simulink model "dynamic_model"  (R2018b)
settings: Solver=ode15s  StartTime=0.0  StopTime=60  FixedStep=0.0001  RelTol=1e-4
undefined symbols (not defined in the file): X, Y, Z
libraries: sm_lib x47, nesl_utility x7
(part 2 of 13)

== matlab function dynamic_model/Dynamic Model/Inertia_matrix ==
  data: q1 input; H output; q2 input; q3 input; q4 input; q5 input; q6 input
function H = Inertia_matrix(q1,q2,q3,q4,q5,q6)
%#codegen

%    This function was generated by the Symbolic Math Toolbox version 9.0.
%    08-Oct-2021 16:14:21

t2 = conj(q1);
t3 = conj(q2);
t4 = conj(q3);
t5 = conj(q4);
t6 = conj(q5);
t7 = conj(q6);
t8 = cos(q1);
t9 = cos(q2);
t10 = cos(q4);
t11 = cos(q5);
t12 = cos(q6);
t13 = sin(q1);
t14 = sin(q2);
t15 = sin(q4);
t16 = sin(q5);
t17 = sin(q6);
t23 = q1+q2;
t44 = 9.007199254740992e+15;
t18 = cos(t2);
t19 = cos(t3);
t20 = cos(t5);
t21 = cos(t6);
t22 = cos(t7);
t24 = sin(t2);
t25 = sin(t3);
t26 = sin(t5);
t27 = sin(t6);
t28 = sin(t7);
t29 = cos(t23);
t30 = sin(t23);
t31 = t2+t3;
t45 = t11.*3.347317932164228e+33;
t48 = t8.*4.990478e-2;
t50 = t13.*4.990478e-2;
t51 = t8.*2.167433e-2;
t52 = t13.*2.167433e-2;
t53 = t10.*t12.*3.315051378778914e+33;
t54 = t8.*t9.*3.641522e-2;
t55 = t8.*t14.*3.641522e-2;
t56 = t9.*t13.*3.641522e-2;
t57 = t15.*t16.*1.990083581481952e+33;
t58 = t13.*t14.*3.641522e-2;
t62 = t13.*t14.*2.462267e-2;
t65 = t11.*t12.*1.025883768304404e+34;
t66 = t11.*t17.*5.575912001630188e+33;
t67 = t10.*t17.*6.099194893302011e+33;
t70 = t8.*t9.*2.462267e-2;
t71 = t8.*t14.*2.462267e-2;
t72 = t9.*t13.*2.462267e-2;
t74 = t15.*t16.*t17.*3.315051378778914e+33;
t81 = t12.*t15.*t16.*6.099194893302011e+33;
t89 = t15.*7.746286054220548e+49;
t92 = t10.*t11.*1.830618490855195e+48;
t94 = t10.*t16.*7.290917220067534e+49;
t96 = t10.*6.997781708721691e+52;
t100 = t10.*t11.*t17.*5.84291401185902e+49;
t102 = t15.*t16.*7.183572847808854e+52;
t103 = t10.*t11.*t12.*1.075008113939401e+50;
t104 = (q3.*t44)./9.007199254740992e+15;
t105 = t10.*t12.*1.196628789628727e+53;
t106 = (t4.*t44)./9.007199254740992e+15;
t109 = t10.*t17.*2.201616617347892e+53;
t110 = q3.*t44.*2.220446049250313e-16i;
t113 = t4.*t44.*2.220446049250313e-16i;
t118 = q3.*t44.*1.110223024625157e-16i;
t119 = t15.*t16.*t17.*1.196628789628727e+53;
t121 = t4.*t44.*1.110223024625157e-16i;
t124 = t12.*t15.*t16.*2.201616617347892e+53;
t128 = t10.*t16.*t44.*4.323455642275676e+17i;
t138 = t12.*t15.*t44.*7.201947557068188e+17i;
t140 = t15.*t17.*t44.*1.325049802940888e+18i;
t152 = t10.*t12.*t16.*t44.*1.325049802940888e+18i;
t154 = t10.*t16.*t17.*t44.*7.201947557068188e+17i;
t193 = t16.*t44.*1.746965228796509e+32i;
t210 = t10.*t44.*4.394953650240249e+33i;
t213 = t11.*t15.*t44.*1.03862462117543e+32i;
t217 = t11.*t44.*6.957746211523004e+33i;
t222 = t15.*t16.*t44.*4.136594366080324e+33i;
t224 = t15.*t44.*3.97028021545552e+36i;
t225 = t12.*t16.*t44.*1.025883768304404e+34i;
t226 = t16.*t17.*t44.*5.575912001630188e+33i;
t229 = t11.*t15.*t17.*t44.*3.315051378778914e+33i;
t234 = t10.*t16.*t44.*4.075691174875038e+36i;
t237 = t11.*t12.*t15.*t44.*6.099194893302011e+33i;
t239 = t12.*t15.*t44.*6.789225223739216e+36i;
t240 = t15.*t17.*t44.*1.249115114148252e+37i;
t249 = t10.*t12.*t16.*t44.*1.249115114148252e+37i;
t251 = t10.*t16.*t17.*t44.*6.789225223739216e+36i;
t284 = t8.*t9.*3.15365435562893e-2;
t285 = t8.*t14.*3.15365435562893e-2;
t286 = t9.*t13.*3.15365435562893e-2;
t287 = t8.*t9.*2.561099610858757e-2;
t289 = t13.*t14.*3.15365435562893e-2;
t290 = t8.*t14.*2.561099610858757e-2;
t291 = t9.*t13.*2.561099610858757e-2;
t292 = t13.*t14.*2.561099610858757e-2;
t294 = t8.*t9.*1.57299335562893e-2;
t296 = t8.*t14.*1.57299335562893e-2;
t297 = t9.*t13.*1.57299335562893e-2;
t298 = t13.*t14.*1.57299335562893e-2;
t299 = t8.*t9.*4.804434610858757e-2;
t300 = t8.*t14.*4.804434610858757e-2;
t301 = t9.*t13.*4.804434610858757e-2;
t302 = t13.*t14.*4.804434610858757e-2;
t311 = t8.*t9.*1.919581841189621e-2;
t313 = t8.*t9.*4.735389991350965e-2;
t315 = t8.*t14.*1.919581841189621e-2;
t316 = t9.*t13.*1.919581841189621e-2;
t317 = t8.*t14.*4.735389991350965e-2;
t318 = t9.*t13.*4.735389991350965e-2;
t319 = t13.*t14.*1.919581841189621e-2;
t320 = t13.*t14.*4.735389991350965e-2;
t321 = t8.*t9.*2.273122991350965e-2;
t322 = t8.*t9.*3.603517512464e-2;
t323 = t8.*t14.*2.273122991350965e-2;
t324 = t9.*t13.*2.273122991350965e-2;
t325 = t8.*t14.*3.603517512464e-2;
t326 = t9.*t13.*3.603517512464e-2;
t327 = t13.*t14.*2.273122991350965e-2;
t328 = t13.*t14.*3.603517512464e-2;
t330 = t8.*t9.*1.141250512464e-2;
t331 = t8.*t14.*1.141250512464e-2;
t332 = t9.*t13.*1.141250512464e-2;
t333 = t13.*t14.*1.141250512464e-2;
t337 = t8.*t9.*5.561103841189621e-2;
t338 = t8.*t14.*5.561103841189621e-2;
t339 = t9.*t13.*5.561103841189621e-2;
t341 = t13.*t14.*5.561103841189621e-2;
t342 = t8.*t9.*3.823389842399381e-2;
t343 = t8.*t14.*3.823389842399381e-2;
t344 = t9.*t13.*3.823389842399381e-2;
t346 = t8.*t9.*7.464911842399381e-2;
t349 = t13.*t14.*3.823389842399381e-2;
t350 = t8.*t14.*7.464911842399381e-2;
t351 = t9.*t13.*7.464911842399381e-2;
t354 = t13.*t14.*7.464911842399381e-2;
t374 = t8.*t9.*t10.*t16.*2.498039274760989e-3;
t375 = t8.*t10.*t14.*t16.*2.498039274760989e-3;
t376 = t9.*t10.*t13.*t16.*2.498039274760989e-3;
t378 = t8.*t9.*t10.*t11.*5.478347731418506e-3;
t379 = t10.*t13.*t14.*t16.*2.498039274760989e-3;
t384 = t8.*t10.*t11.*t14.*5.478347731418506e-3;
t385 = t9.*t10.*t11.*t13.*5.478347731418506e-3;
t388 = t10.*t11.*t13.*t14.*5.478347731418506e-3;
t397 = t8.*t9.*t10.*t16.*4.201698731382561e-3;
t398 = t8.*t10.*t14.*t16.*4.201698731382561e-3;
t399 = t9.*t10.*t13.*t16.*4.201698731382561e-3;
t402 = t10.*t13.*t14.*t16.*4.201698731382561e-3;
t403 = t8.*t9.*t10.*t11.*9.214573584066668e-3;
t404 = t8.*t10.*t11.*t14.*9.214573584066668e-3;
t405 = t9.*t10.*t11.*t13.*9.214573584066668e-3;
t406 = t10.*t11.*t13.*t14.*9.214573584066668e-3;
t410 = t8.*t9.*t15.*2.538961213904336e-3;
t411 = t8.*t14.*t15.*2.538961213904336e-3;
t412 = t9.*t13.*t15.*2.538961213904336e-3;
t413 = t13.*t14.*t15.*2.538961213904336e-3;
t415 = t8.*t9.*t10.*2.842045365580232e-6;
t416 = t8.*t10.*t14.*2.842045365580232e-6;
t417 = t9.*t10.*t13.*2.842045365580232e-6;
t418 = t10.*t13.*t14.*2.842045365580232e-6;
t419 = t10.*t13.*t14.*4.780316517734772e-6;
t420 = t8.*t9.*t15.*4.270529378491088e-3;
t421 = t8.*t14.*t15.*4.270529378491088e-3;
t422 = t9.*t13.*t15.*4.270529378491088e-3;
t423 = t13.*t14.*t15.*4.270529378491088e-3;
t425 = t8.*t9.*t10.*4.780316517734772e-6;
t426 = t8.*t10.*t14.*4.780316517734772e-6;
t427 = t9.*t10.*t13.*4.780316517734772e-6;
t32 = cos(t31);
t33 = sin(t31);
t34 = t30.*7.742227997977903e+15;
t35 = t29.*4.602992943936994e+15;
t36 = t30.*4.602992943936994e+15;
t37 = t29.*7.742227997977903e+15;
t46 = t21.*3.347317932164228e+33;
t47 = t29.*1.580661e-2;
t49 = t30.*1.580661e-2;
t61 = -t52;
t63 = -t53;
t64 = -t54;
t68 = t29.*2.243335e-2;
t69 = t30.*2.243335e-2;
t73 = -t62;
t76 = t20.*t22.*3.315051378778914e+33;
t77 = t26.*t27.*1.990083581481952e+33;
t78 = t21.*t22.*1.025883768304404e+34;
t79 = t21.*t28.*5.575912001630188e+33;
t80 = t20.*t28.*6.099194893302011e+33;
t85 = t26.*t27.*t28.*3.315051378778914e+33;
t86 = t22.*t26.*t27.*6.099194893302011e+33;
t90 = t26.*7.746286054220548e+49;
t91 = -t89;
t95 = -t94;
t97 = t20.*t21.*1.830618490855195e+48;
t98 = t20.*t27.*7.290917220067534e+49;
t99 = t20.*6.997781708721691e+52;
t107 = cos(t104);
t108 = sin(t104);
t111 = t20.*t21.*t28.*5.84291401185902e+49;
t112 = -t105;
t114 = exp(t110);
t115 = cos(t106);
t116 = sin(t106);
t117 = t26.*t27.*7.183572847808854e+52;
t120 = -t113;
t122 = exp(t118);
t123 = t20.*t28.*2.201616617347892e+53;
t125 = t20.*t21.*t22.*1.075008113939401e+50;
t126 = t20.*t22.*1.196628789628727e+53;
t127 = -t118;
t129 = -t121;
t134 = exp(t121);
t141 = t20.*t27.*t44.*4.323455642275676e+17i;
t144 = t26.*t27.*t28.*1.196628789628727e+53;
t148 = -t140;
t149 = t22.*t26.*t27.*2.201616617347892e+53;
t151 = t22.*t26.*t44.*7.201947557068188e+17i;
t153 = t26.*t28.*t44.*1.325049802940888e+18i;
t159 = t20.*t22.*t27.*t44.*1.325049802940888e+18i;
t160 = t20.*t27.*t28.*t44.*7.201947557068188e+17i;
t163 = t18.*7.234522890390001e-5;
t164 = t24.*7.234522890390001e-5;
t165 = t18.*1.665736718274e-4;
t166 = t24.*1.665736718274e-4;
t168 = t18.*1.4420704809832e-3;
t169 = t24.*1.4420704809832e-3;
t170 = t18.*5.42809301582e-4;
t171 = t24.*2.35749519977e-4;
t172 = t24.*5.42809301582e-4;
t173 = t18.*3.62675502933e-4;
t174 = t18.*6.263109763852e-4;
t175 = t24.*3.62675502933e-4;
t176 = t24.*6.263109763852e-4;
t177 = t18.*1.575149421255e-4;
t178 = t24.*1.575149421255e-4;
t180 = t18.*2.35749519977e-4;
t195 = t18.*t19.*2.64642149067e-4;
t196 = t18.*t25.*2.64642149067e-4;
t197 = t19.*t24.*2.64642149067e-4;
t198 = t24.*t25.*2.64642149067e-4;
t201 = t18.*t25.*1.789415608245e-4;
t202 = t19.*t24.*1.789415608245e-4;
t204 = t24.*t25.*1.789415608245e-4;
t211 = t27.*t44.*1.746965228796509e+32i;
t212 = t18.*t19.*1.789415608245e-4;
t215 = t20.*t44.*4.394953650240249e+33i;
t219 = -t210;
t221 = -t213;
t223 = t21.*t44.*6.957746211523004e+33i;
t227 = t21.*t26.*t44.*1.03862462117543e+32i;
t230 = -t224;
t231 = t26.*t27.*t44.*4.136594366080324e+33i;
t232 = t26.*t44.*3.97028021545552e+36i;
t233 = -t229;
t235 = t22.*t27.*t44.*1.025883768304404e+34i;
t236 = t27.*t28.*t44.*5.575912001630188e+33i;
t243 = -t237;
t244 = t20.*t27.*t44.*4.075691174875038e+36i;
t245 = t21.*t26.*t28.*t44.*3.315051378778914e+33i;
t246 = -t240;
t248 = t22.*t26.*t44.*6.789225223739216e+36i;
t250 = t26.*t28.*t44.*1.249115114148252e+37i;
t252 = t21.*t22.*t26.*t44.*6.099194893302011e+33i;
t254 = t20.*t22.*t27.*t44.*1.249115114148252e+37i;
t255 = t20.*t27.*t28.*t44.*6.789225223739216e+36i;
t303 = -t287;
t304 = -t289;
t308 = -t298;
t309 = -t299;
t334 = -t311;
t335 = -t315;
t336 = -t316;
t340 = -t320;
t345 = -t322;
t347 = -t323;
t348 = -t324;
t352 = -t327;
t353 = -t328;
t355 = -t330;
t356 = t18.*t19.*2.273122991350965e-2;
t357 = -t337;
t358 = t18.*t25.*2.273122991350965e-2;
t359 = t19.*t24.*2.273122991350965e-2;
t360 = -t338;
t361 = -t339;
t362 = t24.*t25.*2.273122991350965e-2;
t363 = -t346;
t364 = t18.*t19.*1.141250512464e-2;
t365 = -t349;
t366 = t18.*t25.*1.141250512464e-2;
t367 = t19.*t24.*1.141250512464e-2;
t368 = t24.*t25.*1.141250512464e-2;
t369 = t18.*t19.*1.919581841189621e-2;
t370 = t18.*t25.*1.919581841189621e-2;
t371 = t19.*t24.*1.919581841189621e-2;
t373 = t24.*t25.*1.919581841189621e-2;
t377 = t18.*t19.*3.823389842399381e-2;
t380 = t18.*t25.*3.823389842399381e-2;
t381 = t19.*t24.*3.823389842399381e-2;
t386 = t24.*t25.*3.823389842399381e-2;
t394 = -t374;
t395 = -t375;
t396 = -t376;
t401 = -t388;
t407 = -t398;
t408 = -t399;
t409 = -t402;
t414 = -t403;
t424 = -t413;
t428 = -t418;
t429 = -t420;
t430 = -t425;
t493 = t24.*t25.*5.250384412218911e-5;
t496 = t18.*t19.*8.548515114112684e-5;
t497 = t18.*t25.*8.548515114112684e-5;
t498 = t19.*t24.*8.548515114112684e-5;
t499 = t18.*t19.*1.052636211784891e-4;
t500 = t24.*t25.*8.548515114112684e-5;
t502 = t18.*t25.*1.052636211784891e-4;
t503 = t19.*t24.*1.052636211784891e-4;
t504 = t24.*t25.*1.052636211784891e-4;
t505 = t18.*t19.*5.250384412218911e-5;
t507 = t18.*t25.*5.250384412218911e-5;
t508 = t19.*t24.*5.250384412218911e-5;
t515 = t18.*t19.*1.603638597716268e-4;
t517 = t18.*t25.*1.603638597716268e-4;
t518 = t19.*t24.*1.603638597716268e-4;
t520 = t24.*t25.*1.603638597716268e-4;
t529 = t18.*t19.*1.041288275878652e-3;
t532 = t18.*t25.*1.041288275878652e-3;
t533 = t19.*t24.*1.041288275878652e-3;
t534 = t24.*t25.*1.041288275878652e-3;
t538 = t18.*t19.*5.150636339692531e-4;
t540 = t18.*t25.*5.150636339692531e-4;
t541 = t19.*t24.*5.150636339692531e-4;
t542 = t24.*t25.*5.150636339692531e-4;
t546 = t18.*t19.*8.119509961859382e-4;
t547 = t18.*t19.*1.606961034807054e-3;
t548 = t18.*t25.*8.119509961859382e-4;
t549 = t19.*t24.*8.119509961859382e-4;
t550 = t18.*t25.*1.606961034807054e-3;
t551 = t19.*t24.*1.606961034807054e-3;
t552 = t24.*t25.*8.119509961859382e-4;
t553 = t24.*t25.*1.606961034807054e-3;
t575 = t18.*t19.*t26.*2.761602722751607e-5;
t576 = t18.*t25.*t26.*2.761602722751607e-5;
t577 = t19.*t24.*t26.*2.761602722751607e-5;
t578 = t24.*t25.*t26.*2.761602722751607e-5;
t581 = t18.*t19.*t20.*t21.*5.958744043986595e-5;
t582 = t18.*t20.*t21.*t25.*5.958744043986595e-5;
t583 = t19.*t20.*t21.*t24.*5.958744043986595e-5;
t584 = t20.*t21.*t24.*t25.*5.958744043986595e-5;
t586 = t18.*t19.*t20.*t27.*2.71709233876478e-5;
t587 = t18.*t20.*t25.*t27.*2.71709233876478e-5;
t588 = t19.*t20.*t24.*t27.*2.71709233876478e-5;
t589 = t20.*t24.*t25.*t27.*2.71709233876478e-5;
t591 = t18.*t19.*t20.*t27.*4.570145693137498e-5;
t592 = t18.*t20.*t25.*t27.*4.570145693137498e-5;
t593 = t19.*t20.*t24.*t27.*4.570145693137498e-5;
t594 = t18.*t19.*t20.*3.091264323687963e-8;
t597 = t20.*t24.*t25.*t27.*4.570145693137498e-5;
t598 = t18.*t20.*t25.*3.091264323687963e-8;
t599 = t19.*t20.*t24.*3.091264323687963e-8;
t601 = t20.*t24.*t25.*3.091264323687963e-8;
t603 = t18.*t19.*t26.*4.645012099690971e-5;
t604 = t18.*t25.*t26.*4.645012099690971e-5;
t605 = t19.*t24.*t26.*4.645012099690971e-5;
t606 = t24.*t25.*t26.*4.645012099690971e-5;
t610 = t18.*t19.*t20.*t21.*1.002259954165347e-4;
t612 = t18.*t20.*t21.*t25.*1.002259954165347e-4;
t613 = t19.*t20.*t21.*t24.*1.002259954165347e-4;
t616 = t20.*t21.*t24.*t25.*1.002259954165347e-4;
t625 = t18.*t19.*t20.*5.199502473174935e-8;
t626 = t18.*t20.*t25.*5.199502473174935e-8;
t627 = t19.*t20.*t24.*5.199502473174935e-8;
t628 = t20.*t24.*t25.*5.199502473174935e-8;
t38 = -t36;
t39 = t32.*4.602992943936994e+15;
t40 = t33.*4.602992943936994e+15;
t41 = t32.*7.742227997977903e+15;
t42 = t33.*7.742227997977903e+15;
t59 = -t47;
t60 = -t49;
t75 = -t69;
t82 = -t76;
t83 = t34+t35;
t93 = -t90;
t101 = -t98;
t130 = 1.0./t122;
t131 = t10.*t107;
t132 = t15.*t107;
t133 = exp(t120);
t135 = -t126;
t136 = -t115;
t137 = exp(t129);
t139 = t108.*1i;
t142 = t116.*1i;
t143 = t20.*t115;
t145 = t26.*t115;
t146 = t122-1.0;
t150 = -t141;
t157 = -t151;
t161 = -t159;
t162 = -t160;
t167 = -t164;
t181 = -t171;
t182 = t33.*1.71926916309e-4;
t183 = t32.*4.567547574683999e-4;
t184 = t33.*4.567547574683999e-4;
t185 = -t176;
t186 = t32.*1.148721671835e-4;
t187 = t33.*1.148721671835e-4;
t188 = -t178;
t189 = t32.*1.71926916309e-4;
t200 = t32.*2.44005304615e-4;
t203 = t33.*2.44005304615e-4;
t205 = t32.*6.48243952274e-4;
t206 = t33.*6.48243952274e-4;
t207 = -t195;
t208 = t32.*1.630310061225e-4;
t209 = t33.*1.630310061225e-4;
t216 = -t204;
t220 = -t211;
t228 = -t223;
t238 = -t231;
t241 = -t235;
t242 = -t236;
t247 = -t244;
t253 = -t248;
t256 = -t254;
t257 = -t255;
t258 = t114.*3.064357668490995e+34;
t259 = t45.*t114;
t263 = t53.*t114;
t265 = t57.*t114;
t269 = t10.*t12.*t114.*-3.315051378778914e+33;
t271 = t65.*t114;
t272 = t66.*t114;
t274 = t67.*t114;
t276 = t74.*t114;
t295 = t81.*t114;
t382 = -t358;
t383 = -t359;
t387 = -t362;
t390 = -t364;
t391 = -t369;
t392 = -t370;
t393 = -t371;
t400 = -t386;
t431 = t89.*t114;
t432 = t15.*t114.*-7.746286054220548e+49;
t433 = t92.*t114;
t434 = t94.*t114;
t435 = t10.*t16.*t114.*-7.290917220067534e+49;
t436 = t96.*t114;
t438 = t100.*t114;
t440 = t103.*t114;
t442 = t102.*t114;
t443 = t109.*t114;
t444 = t105.*t114;
t447 = t10.*t12.*t114.*-1.196628789628727e+53;
t449 = t114.*t124;
t450 = t114.*t119;
t451 = t114.*t128;
t454 = t114.*t138;
t455 = t114.*t140;
t457 = t10.*t16.*t44.*t114.*-4.323455642275676e+17i;
t460 = t12.*t15.*t44.*t114.*-7.201947557068188e+17i;
t465 = t114.*t152;
t466 = t114.*t154;
t468 = t107.*7.38843356682345e-1;
t469 = t107.*2.61156643317655e-1;
t472 = t10.*t12.*t16.*t44.*t114.*-1.325049802940888e+18i;
t473 = t10.*t16.*t17.*t44.*t114.*-7.201947557068188e+17i;
t476 = t115.*7.38843356682345e-1;
t477 = t115.*2.61156643317655e-1;
t481 = t107.*4.721390555247569e-2;
t482 = t16.*t107.*1.07201054193752e-2;
t483 = t11.*t107.*4.888197259476159e-3;
t492 = t114.*t193;
t494 = t114.*t210;
t501 = t16.*t44.*t114.*-1.746965228796509e+32i;
t509 = -t493;
t512 = t114.*t213;
t513 = -t496;
t514 = -t504;
t516 = t114.*t217;
t521 = t114.*t222;
t524 = -t515;
t525 = t11.*t44.*t114.*-6.957746211523004e+33i;
t526 = t114.*t225;
t527 = t114.*t226;
t528 = t15.*t16.*t44.*t114.*-4.136594366080324e+33i;
t531 = t114.*t224;
t535 = t12.*t16.*t44.*t114.*-1.025883768304404e+34i;
t536 = t16.*t17.*t44.*t114.*-5.575912001630188e+33i;
t537 = t114.*t229;
t543 = -t529;
t545 = -t534;
t555 = t114.*t234;
H = ft_1({t10,t100,t101,t102,t103,t107,t108,t109,t11,t111,t112,t114,t115,t116,t117,t119,t12,t123,t124,t125,t126,t128,t13,t130,t131,t132,t133,t134,t135,t136,t137,t138,t139,t14,t141,t142,t143,t144,t145,t146,t148,t149,t15,t150,t151,t152,t153,t154,t157,t159,t16,t160,t161,t162,t163,t164,t165,t166,t167,t168,t169,t17,t170,t172,t173,t174,t175,t176,t177,t18,t180,t181,t182,t183,t184,t185,t186,t187,t188,t189,t19,t193,t196,t197,t198,t20,t200,t201,t202,t203,t205,t206,t207,t208,t209,t21,t211,t212,t215,t216,t217,t219,t22,t220,t221,t222,t223,t225,t226,t227,t228,t230,t231,t232,t233,t234,t235,t236,t237,t238,t239,t24,t240,t241,t242,t243,t244,t245,t246,t247,t248,t249,t25,t250,t251,t252,t253,t254,t255,t256,t257,t258,t259,t26,t265,t269,t27,t271,t272,t274,t276,t28,t284,t285,t286,t29,t290,t291,t292,t294,t295,t296,t297,t30,t300,t301,t302,t303,t304,t308,t309,t313,t317,t318,t319,t32,t320,t321,t322,t323,t324,t325,t326,t328,t33,t331,t332,t333,t334,t335,t336,t338,t339,t340,t341,t342,t343,t344,t345,t347,t348,t349,t350,t351,t352,t353,t354,t355,t356,t357,t358,t359,t36,t360,t361,t363,t365,t366,t367,t368,t37,t373,t375,t376,t377,t378,t379,t38,t380,t381,t382,t383,t384,t385,t386,t387,t39,t390,t391,t392,t393,t394,t395,t396,t397,t40,t400,t401,t402,t403,t404,t405,t406,t407,t408,t409,t41,t410,t411,t412,t414,t415,t416,t417,t419,t42,t420,t421,t422,t423,t424,t425,t426,t427,t428,t429,t430,t432,t433,t435,t436,t438,t44,t440,t442,t443,t447,t449,t45,t450,t455,t457,t46,t460,t468,t469,t47,t472,t473,t476,t477,t48,t481,t482,t483,t49,t493,t494,t497,t498,t499,t50,t500,t501,t502,t503,t504,t505,t507,t508,t509,t51,t512,t513,t514,t517,t518,t52,t520,t524,t525,t528,t529,t531,t532,t533,t534,t535,t536,t537,t538,t540,t541,t542,t543,t545,t546,t547,t548,t549,t55,t550,t551,t552,t553,t56,t57,t575,t576,t577,t578,t58,t581,t582,t583,t584,t586,t587,t588,t589,t59,t591,t592,t593,t594,t597,t598,t599,t60,t601,t603,t604,t605,t606,t61,t610,t612,t613,t616,t625,t626,t627,t628,t63,t64,t65,t66,t67,t68,t69,t70,t71,t72,t73,t74,t75,t76,t77,t78,t79,t8,t80,t81,t82,t83,t85,t86,t9,t90,t91,t92,t93,t95,t96,t97,t98,t99});
end
function H = ft_1(ct)
t10 = ct{1};
t100 = ct{2};
t101 = ct{3};
t102 = ct{4};
t103 = ct{5};
t107 = ct{6};
t108 = ct{7};
t109 = ct{8};
t11 = ct{9};
t111 = ct{10};
t112 = ct{11};
t114 = ct{12};
t115 = ct{13};
t116 = ct{14};
t117 = ct{15};
t119 = ct{16};
t12 = ct{17};
t123 = ct{18};
t124 = ct{19};
t125 = ct{20};
t126 = ct{21};
t128 = ct{22};
t13 = ct{23};
t130 = ct{24};
t131 = ct{25};
t132 = ct{26};
t133 = ct{27};
t134 = ct{28};
t135 = ct{29};
t136 = ct{30};
t137 = ct{31};
t138 = ct{32};
t139 = ct{33};
t14 = ct{34};
t141 = ct{35};
t142 = ct{36};
t143 = ct{37};
t144 = ct{38};
t145 = ct{39};
t146 = ct{40};
t148 = ct{41};
t149 = ct{42};
t15 = ct{43};
t150 = ct{44};
t151 = ct{45};
t152 = ct{46};
t153 = ct{47};
t154 = ct{48};
t157 = ct{49};
t159 = ct{50};
t16 = ct{51};
t160 = ct{52};
t161 = ct{53};
t162 = ct{54};
t163 = ct{55};
t164 = ct{56};
t165 = ct{57};
t166 = ct{58};
t167 = ct{59};
t168 = ct{60};
t169 = ct{61};
t17 = ct{62};
t170 = ct{63};
t172 = ct{64};
t173 = ct{65};
t174 = ct{66};
t175 = ct{67};
t176 = ct{68};
t177 = ct{69};
t18 = ct{70};
t180 = ct{71};
t181 = ct{72};
t182 = ct{73};
t183 = ct{74};
t184 = ct{75};
t185 = ct{76};
t186 = ct{77};
t187 = ct{78};
t188 = ct{79};
t189 = ct{80};
t19 = ct{81};
t193 = ct{82};
t196 = ct{83};
t197 = ct{84};
t198 = ct{85};
t20 = ct{86};
t200 = ct{87};
t201 = ct{88};
t202 = ct{89};
t203 = ct{90};
t205 = ct{91};
t206 = ct{92};
t207 = ct{93};
t208 = ct{94};
t209 = ct{95};
t21 = ct{96};
t211 = ct{97};
t212 = ct{98};
t215 = ct{99};
t216 = ct{100};
t217 = ct{101};
t219 = ct{102};
t22 = ct{103};
t220 = ct{104};
t221 = ct{105};
t222 = ct{106};
t223 = ct{107};
t225 = ct{108};
t226 = ct{109};
t227 = ct{110};
t228 = ct{111};
t230 = ct{112};
t231 = ct{113};
t232 = ct{114};
t233 = ct{115};
t234 = ct{116};
t235 = ct{117};
t236 = ct{118};
t237 = ct{119};
t238 = ct{120};
t239 = ct{121};
t24 = ct{122};
t240 = ct{123};
t241 = ct{124};
t242 = ct{125};
t243 = ct{126};
t244 = ct{127};
t245 = ct{128};
t246 = ct{129};
t247 = ct{130};
t248 = ct{131};
t249 = ct{132};
t25 = ct{133};
t250 = ct{134};
t251 = ct{135};
t252 = ct{136};
t253 = ct{137};
t254 = ct{138};
t255 = ct{139};
t256 = ct{140};
t257 = ct{141};
t258 = ct{142};
t259 = ct{143};
t26 = ct{144};
t265 = ct{145};
t269 = ct{146};
t27 = ct{147};
t271 = ct{148};
t272 = ct{149};
t274 = ct{150};
t276 = ct{151};
t28 = ct{152};
t284 = ct{153};
t285 = ct{154};
t286 = ct{155};
t29 = ct{156};
t290 = ct{157};
t291 = ct{158};
t292 = ct{159};
t294 = ct{160};
t295 = ct{161};
t296 = ct{162};
t297 = ct{163};
t30 = ct{164};
t300 = ct{165};
t301 = ct{166};
t302 = ct{167};
t303 = ct{168};
t304 = ct{169};
t308 = ct{170};
t309 = ct{171};
t313 = ct{172};
t317 = ct{173};
t318 = ct{174};
t319 = ct{175};
t32 = ct{176};
t320 = ct{177};
t321 = ct{178};
t322 = ct{179};
t323 = ct{180};
t324 = ct{181};
t325 = ct{182};
t326 = ct{183};
t328 = ct{184};
t33 = ct{185};
t331 = ct{186};
t332 = ct{187};
t333 = ct{188};
t334 = ct{189};
t335 = ct{190};
t336 = ct{191};
t338 = ct{192};
t339 = ct{193};
t340 = ct{194};
t341 = ct{195};
t342 = ct{196};
t343 = ct{197};
t344 = ct{198};
t345 = ct{199};
t347 = ct{200};
t348 = ct{201};
t349 = ct{202};
t350 = ct{203};
t351 = ct{204};
t352 = ct{205};
t353 = ct{206};
t354 = ct{207};
t355 = ct{208};
t356 = ct{209};
t357 = ct{210};
t358 = ct{211};
t359 = ct{212};
t36 = ct{213};
t360 = ct{214};
t361 = ct{215};
t363 = ct{216};
t365 = ct{217};
t366 = ct{218};
t367 = ct{219};
t368 = ct{220};
t37 = ct{221};
t373 = ct{222};
t375 = ct{223};
t376 = ct{224};
t377 = ct{225};
t378 = ct{226};
t379 = ct{227};
t38 = ct{228};
t380 = ct{229};
t381 = ct{230};
t382 = ct{231};
t383 = ct{232};
t384 = ct{233};
t385 = ct{234};
t386 = ct{235};
t387 = ct{236};
t39 = ct{237};
t390 = ct{238};
t391 = ct{239};
t392 = ct{240};
t393 = ct{241};
t394 = ct{242};
t395 = ct{243};
t396 = ct{244};
t397 = ct{245};
t40 = ct{246};
t400 = ct{247};
t401 = ct{248};
t402 = ct{249};
t403 = ct{250};
t404 = ct{251};
t405 = ct{252};
t406 = ct{253};
t407 = ct{254};
t408 = ct{255};
t409 = ct{256};
t41 = ct{257};
t410 = ct{258};
t411 = ct{259};
t412 = ct{260};
t414 = ct{261};
t415 = ct{262};
t416 = ct{263};
t417 = ct{264};
t419 = ct{265};
t42 = ct{266};
t420 = ct{267};
t421 = ct{268};
t422 = ct{269};
t423 = ct{270};
t424 = ct{271};
t425 = ct{272};
t426 = ct{273};
t427 = ct{274};
t428 = ct{275};
t429 = ct{276};
t430 = ct{277};
t432 = ct{278};
t433 = ct{279};
t435 = ct{280};
t436 = ct{281};
t438 = ct{282};
t44 = ct{283};
t440 = ct{284};
t442 = ct{285};
t443 = ct{286};
t447 = ct{287};
t449 = ct{288};
t45 = ct{289};
t450 = ct{290};
t455 = ct{291};
t457 = ct{292};
t46 = ct{293};
t460 = ct{294};
t468 = ct{295};
t469 = ct{296};
t47 = ct{297};
t472 = ct{298};
t473 = ct{299};
t476 = ct{300};
t477 = ct{301};
t48 = ct{302};
t481 = ct{303};
t482 = ct{304};
t483 = ct{305};
t49 = ct{306};
t493 = ct{307};
t494 = ct{308};
t497 = ct{309};
t498 = ct{310};
t499 = ct{311};
t50 = ct{312};
t500 = ct{313};
t501 = ct{314};
t502 = ct{315};
t503 = ct{316};
t504 = ct{317};
t505 = ct{318};
t507 = ct{319};
t508 = ct{320};
t509 = ct{321};
t51 = ct{322};
t512 = ct{323};
t513 = ct{324};
t514 = ct{325};
t517 = ct{326};
t518 = ct{327};
t52 = ct{328};
t520 = ct{329};
t524 = ct{330};
t525 = ct{331};
t528 = ct{332};
t529 = ct{333};
t531 = ct{334};
t532 = ct{335};
t533 = ct{336};
t534 = ct{337};
t535 = ct{338};
t536 = ct{339};
t537 = ct{340};
t538 = ct{341};
t540 = ct{342};
t541 = ct{343};
t542 = ct{344};
t543 = ct{345};
t545 = ct{346};
t546 = ct{347};
t547 = ct{348};
t548 = ct{349};
t549 = ct{350};
t55 = ct{351};
t550 = ct{352};
t551 = ct{353};
t552 = ct{354};
t553 = ct{355};
t56 = ct{356};
t57 = ct{357};
t575 = ct{358};
t576 = ct{359};
t577 = ct{360};
t578 = ct{361};
t58 = ct{362};
t581 = ct{363};
t582 = ct{364};
t583 = ct{365};
t584 = ct{366};
t586 = ct{367};
t587 = ct{368};
t588 = ct{369};
t589 = ct{370};
t59 = ct{371};
t591 = ct{372};
t592 = ct{373};
t593 = ct{374};
t594 = ct{375};
t597 = ct{376};
t598 = ct{377};
t599 = ct{378};
t60 = ct{379};
t601 = ct{380};
t603 = ct{381};
t604 = ct{382};
t605 = ct{383};
t606 = ct{384};
t61 = ct{385};
t610 = ct{386};
t612 = ct{387};
t613 = ct{388};
t616 = ct{389};
t625 = ct{390};
t626 = ct{391};
t627 = ct{392};
t628 = ct{393};
t63 = ct{394};
t64 = ct{395};
t65 = ct{396};
t66 = ct{397};
t67 = ct{398};
t68 = ct{399};
t69 = ct{400};
t70 = ct{401};
t71 = ct{402};
t72 = ct{403};
t73 = ct{404};
t74 = ct{405};
t75 = ct{406};
t76 = ct{407};
t77 = ct{408};
t78 = ct{409};
t79 = ct{410};
t8 = ct{411};
t80 = ct{412};
t81 = ct{413};
t82 = ct{414};
t83 = ct{415};
t85 = ct{416};
t86 = ct{417};
t9 = ct{418};
t90 = ct{419};
t91 = ct{420};
t92 = ct{421};
t93 = ct{422};
t95 = ct{423};
t96 = ct{424};
t97 = ct{425};
t98 = ct{426};
t99 = ct{427};
t556 = -t542;
t557 = t114.*t237;
t558 = -t546;
t559 = -t547;
t560 = -t550;
t561 = -t551;
t564 = t10.*t16.*t44.*t114.*-4.075691174875038e+36i;
t565 = t114.*t239;
t567 = t114.*t240;
t570 = t12.*t15.*t44.*t114.*-6.789225223739216e+36i;
t572 = t114.*t249;
t573 = t114.*t251;
t579 = t10.*t12.*t16.*t44.*t114.*-1.249115114148252e+37i;
t580 = t10.*t16.*t17.*t44.*t114.*-6.789225223739216e+36i;
t595 = -t576;
t596 = -t577;
t600 = -t578;
t607 = -t582;
t608 = -t583;
t609 = -t584;
t614 = -t586;
t617 = -t591;
t618 = -t592;
t619 = -t593;
t620 = -t598;
t621 = -t599;
t622 = -t601;
t624 = -t606;
t630 = -t616;
t631 = -t628;
t633 = t10.*t44.*t108.*5.673626844500105e-17;
t634 = t15.*t44.*t108.*5.673626844500105e-17;
t635 = t11.*t44.*t108.*9.543032792050485e-17;
t636 = t16.*t44.*t108.*9.543032792050485e-17;
t640 = t20.*t44.*t116.*5.673626844500105e-17;
t641 = t26.*t44.*t116.*5.673626844500105e-17;
t642 = t21.*t44.*t116.*9.543032792050485e-17;
t643 = t27.*t44.*t116.*9.543032792050485e-17;
t646 = t11.*t44.*t108.*5.725819675230291e-19;
t647 = t15.*t44.*t108.*7.194245199571015e-21;
t648 = t10.*t11.*t44.*t108.*1.384627967837559e-18;
t649 = t10.*t16.*t44.*t108.*6.313682909819818e-19;
t652 = t21.*t44.*t116.*5.725819675230291e-19;
t654 = t10.*t44.*t108.*5.673626844500105e-25;
t655 = t16.*t44.*t108.*9.543032792050485e-25;
t656 = t107.*t115.*2.2e-7;
t657 = t8.*t9.*t107.*1.374006108587572e-3;
t658 = t8.*t14.*t107.*1.374006108587572e-3;
t659 = t9.*t13.*t107.*1.374006108587572e-3;
t660 = t13.*t14.*t107.*1.374006108587572e-3;
t661 = t13.*t14.*t107.*6.463878411896211e-3;
t662 = t8.*t9.*t107.*2.311076443710702e-3;
t665 = t8.*t14.*t107.*2.311076443710702e-3;
t666 = t9.*t13.*t107.*2.311076443710702e-3;
t668 = t13.*t14.*t107.*2.311076443710702e-3;
t669 = t8.*t9.*t107.*6.463878411896211e-3;
t670 = t8.*t14.*t107.*6.463878411896211e-3;
t671 = t9.*t13.*t107.*6.463878411896211e-3;
t673 = t8.*t9.*t107.*1.087223487536e-2;
t675 = t8.*t14.*t107.*1.087223487536e-2;
t676 = t9.*t13.*t107.*1.087223487536e-2;
t677 = t13.*t14.*t107.*1.087223487536e-2;
t678 = t8.*t9.*t107.*2.550195842399381e-2;
t679 = t8.*t14.*t107.*2.550195842399381e-2;
t680 = t9.*t13.*t107.*2.550195842399381e-2;
t681 = t13.*t14.*t107.*2.550195842399381e-2;
t682 = t115.*5.135409293037228e-4;
t691 = t8.*t9.*t107.*4.289426008649035e-2;
t692 = t8.*t14.*t107.*4.289426008649035e-2;
t693 = t9.*t13.*t107.*4.289426008649035e-2;
t694 = t13.*t14.*t107.*4.289426008649035e-2;
t695 = t18.*t19.*t115.*6.463878411896211e-3;
t696 = t18.*t25.*t115.*6.463878411896211e-3;
t697 = t19.*t24.*t115.*6.463878411896211e-3;
t698 = t24.*t25.*t115.*6.463878411896211e-3;
t700 = t21.*t115.*5.316843277159623e-5;
t701 = t27.*t115.*1.166015146360021e-4;
t710 = t18.*t19.*t115.*1.087223487536e-2;
t715 = t18.*t25.*t115.*1.087223487536e-2;
t716 = t19.*t24.*t115.*1.087223487536e-2;
t720 = t24.*t25.*t115.*1.087223487536e-2;
t728 = t18.*t19.*t115.*2.550195842399381e-2;
t729 = t18.*t25.*t115.*2.550195842399381e-2;
t730 = t19.*t24.*t115.*2.550195842399381e-2;
t731 = t24.*t25.*t115.*2.550195842399381e-2;
t735 = t18.*t25.*t115.*4.289426008649035e-2;
t736 = t19.*t24.*t115.*4.289426008649035e-2;
t737 = t24.*t25.*t115.*4.289426008649035e-2;
t757 = t18.*t19.*t115.*4.289426008649035e-2;
t779 = t10.*t44.*t108.*(t36-t37).*(-1.232595164407831e-32);
t781 = t15.*t44.*t108.*(t36-t37).*(-1.232595164407831e-32);
t782 = (t10.*t44.*t108.*(t36-t37))./8.112963841460668e+31;
t783 = t44.*t108.*1.930470600839964e-18;
t784 = t15.*t44.*t108.*5.582848814988104e-22;
t785 = t44.*t108.*3.311325901843639e-18;
t786 = t44.*t108.*5.241796502683603e-18;
t787 = t44.*t116.*1.930470600839964e-18;
t788 = t44.*t116.*3.311325901843639e-18;
t790 = t44.*t116.*5.241796502683603e-18;
t791 = t11.*t44.*t108.*5.426989146380022e-19;
t793 = t10.*t44.*t108.*3.31613276532711e-19;
t795 = t16.*t44.*t108.*1.190170786299927e-18;
t798 = t10.*t44.*t108.*3.676510195236068e-21;
t800 = t10.*t44.*t108.*4.442449819243582e-22;
t802 = t10.*t44.*t108.*3.517648643590065e-23;
t803 = t44.*t108.*3.091942624624357e-22;
t805 = t10.*t11.*t44.*t108.*7.075931802640439e-19;
t809 = t10.*t44.*t108.*1.838255097618034e-22;
t810 = t10.*t16.*t44.*t108.*3.226512155691387e-19;
t811 = t21.*t44.*t116.*5.426989146380022e-19;
t812 = t20.*t44.*t116.*3.31613276532711e-19;
t813 = t44.*t108.*2.967883198327701e-22;
t814 = t27.*t44.*t116.*1.190170786299927e-18;
t817 = t15.*t44.*t108.*3.279367663374749e-19;
t819 = t10.*t44.*t108.*3.670836568391568e-22;
t820 = t15.*t44.*t108.*3.670836568391568e-22;
t822 = t11.*t44.*t108.*2.988305288502687e-20;
t823 = t20.*t44.*t116.*3.676510195236068e-21;
t824 = t11.*t44.*t108.*5.439528691468777e-23;
t825 = t16.*t44.*t108.*9.733893447891495e-23;
t829 = t16.*t44.*t108.*2.290327870092116e-23;
t830 = t26.*t44.*t116.*3.670836568391568e-22;
t831 = t21.*t44.*t116.*2.988305288502687e-20;
t832 = t8.*t9.*t15.*t16.*t44.*t108.*3.226512155691387e-19;
t833 = t8.*t14.*t15.*t16.*t44.*t108.*3.226512155691387e-19;
t834 = t9.*t13.*t15.*t16.*t44.*t108.*3.226512155691387e-19;
t835 = t13.*t14.*t15.*t16.*t44.*t108.*3.226512155691387e-19;
t836 = t8.*t9.*t15.*t16.*t44.*t108.*5.426989146380022e-19;
t837 = t8.*t14.*t15.*t16.*t44.*t108.*5.426989146380022e-19;
t838 = t9.*t13.*t15.*t16.*t44.*t108.*5.426989146380022e-19;
t839 = t26.*t44.*t116.*7.825108561121397e-23;
t841 = t13.*t14.*t15.*t16.*t44.*t108.*5.426989146380022e-19;
t842 = t8.*t9.*t11.*t15.*t44.*t108.*1.190170786299927e-18;
t844 = t8.*t11.*t14.*t15.*t44.*t108.*1.190170786299927e-18;
t845 = t9.*t11.*t13.*t15.*t44.*t108.*1.190170786299927e-18;
t846 = t11.*t13.*t14.*t15.*t44.*t108.*1.190170786299927e-18;
t847 = t8.*t9.*t11.*t15.*t44.*t108.*7.075931802640439e-19;
t848 = t8.*t11.*t14.*t15.*t44.*t108.*7.075931802640439e-19;
t849 = t9.*t11.*t13.*t15.*t44.*t108.*7.075931802640439e-19;
t850 = t11.*t13.*t14.*t15.*t44.*t108.*7.075931802640439e-19;
t851 = t11.*t44.*t108.*3.817213116820194e-24;
t852 = t16.*t44.*t108.*3.817213116820194e-24;
t854 = t20.*t27.*t44.*t116.*6.867329764181918e-21;
t862 = t20.*t21.*t44.*t116.*1.506045994337235e-20;
t864 = t8.*t9.*t10.*t44.*t108.*3.279367663374749e-19;
t867 = t8.*t10.*t14.*t44.*t108.*3.279367663374749e-19;
t868 = t9.*t10.*t13.*t44.*t108.*3.279367663374749e-19;
t870 = t10.*t13.*t14.*t44.*t108.*3.279367663374749e-19;
t871 = t8.*t14.*t15.*t44.*t108.*(-3.670836568391568e-22);
t872 = t9.*t13.*t15.*t44.*t108.*(-3.670836568391568e-22);
t873 = t8.*t9.*t15.*t44.*t108.*6.174342216456664e-22;
t874 = t13.*t14.*t15.*t44.*t108.*(-3.670836568391568e-22);
t875 = t8.*t14.*t15.*t44.*t108.*6.174342216456664e-22;
t876 = t9.*t13.*t15.*t44.*t108.*6.174342216456664e-22;
t877 = t13.*t14.*t15.*t44.*t108.*6.174342216456664e-22;
t879 = t8.*t9.*t10.*t44.*t108.*5.515892039870764e-19;
t880 = t8.*t10.*t14.*t44.*t108.*5.515892039870764e-19;
t881 = t9.*t10.*t13.*t44.*t108.*5.515892039870764e-19;
t882 = t10.*t13.*t14.*t44.*t108.*5.515892039870764e-19;
t892 = t18.*t19.*t115.*7.713980286110892e-6;
t893 = t18.*t25.*t115.*7.713980286110892e-6;
t894 = t19.*t24.*t115.*7.713980286110892e-6;
t895 = t24.*t25.*t115.*7.713980286110892e-6;
t896 = t18.*t19.*t115.*4.586198809426854e-6;
t897 = t18.*t25.*t115.*4.586198809426854e-6;
t898 = t19.*t24.*t115.*4.586198809426854e-6;
t899 = t24.*t25.*t115.*4.586198809426854e-6;
t904 = t24.*t25.*t115.*1.867830746966542e-4;
t909 = t18.*t19.*t115.*1.867830746966542e-4;
t910 = t18.*t25.*t115.*1.867830746966542e-4;
t911 = t19.*t24.*t115.*1.867830746966542e-4;
t915 = t18.*t19.*t115.*4.665565775347468e-4;
t916 = t18.*t25.*t115.*4.665565775347468e-4;
t917 = t19.*t24.*t115.*4.665565775347468e-4;
t918 = t18.*t19.*t115.*2.773822515819383e-4;
t919 = t24.*t25.*t115.*4.665565775347468e-4;
t920 = t18.*t19.*t115.*3.141688827417478e-4;
t921 = t18.*t25.*t115.*2.773822515819383e-4;
t922 = t19.*t24.*t115.*2.773822515819383e-4;
t923 = t18.*t25.*t115.*3.141688827417478e-4;
t924 = t19.*t24.*t115.*3.141688827417478e-4;
t925 = t24.*t25.*t115.*2.773822515819383e-4;
t926 = t24.*t25.*t115.*3.141688827417478e-4;
t983 = t15.*t44.*t108.*(t36-t37).*(-7.204296868834178e-35);
t986 = t15.*t44.*t108.*(t36-t37).*(-7.987216665362745e-37);
t987 = t15.*t44.*t108.*(t36-t37).*7.204296868834178e-35;
t990 = t10.*t44.*t108.*(t36-t37).*(-7.974890713718666e-38);
t993 = t10.*t44.*t108.*(t36-t37).*7.974890713718666e-38;
t1006 = t20.*t21.*t44.*t116.*7.696420262413979e-21;
t1007 = t26.*t44.*t116.*3.566935413776081e-21;
t1011 = t20.*t27.*t44.*t116.*3.509445006623964e-21;
t1017 = t20.*t44.*t116.*3.992732227073824e-24;
t1018 = t108.*t116.*7.913131956031502e-8;
t1019 = t108.*t116.*2.393852475650798e-6;
t1021 = t108.*t116.*2.297802839282093e-6;
t1022 = t18.*t19.*t26.*t27.*t44.*t116.*3.509445006623964e-21;
t1023 = t18.*t25.*t26.*t27.*t44.*t116.*3.509445006623964e-21;
t1024 = t19.*t24.*t26.*t27.*t44.*t116.*3.509445006623964e-21;
t1026 = t24.*t25.*t26.*t27.*t44.*t116.*3.509445006623964e-21;
t1027 = t18.*t19.*t21.*t26.*t44.*t116.*7.696420262413979e-21;
t1028 = t18.*t19.*t20.*t44.*t116.*3.566935413776081e-21;
t1029 = t18.*t21.*t25.*t26.*t44.*t116.*7.696420262413979e-21;
t1030 = t19.*t21.*t24.*t26.*t44.*t116.*7.696420262413979e-21;
t1031 = t18.*t20.*t25.*t44.*t116.*3.566935413776081e-21;
t1032 = t19.*t20.*t24.*t44.*t116.*3.566935413776081e-21;
t1033 = t21.*t24.*t25.*t26.*t44.*t116.*7.696420262413979e-21;
t1034 = t20.*t24.*t25.*t44.*t116.*3.566935413776081e-21;
t1035 = t18.*t19.*t26.*t44.*t116.*3.992732227073824e-24;
t1036 = t18.*t25.*t26.*t44.*t116.*3.992732227073824e-24;
t1037 = t19.*t24.*t26.*t44.*t116.*3.992732227073824e-24;
t1038 = t18.*t19.*t26.*t27.*t44.*t116.*5.902881824626087e-21;
t1040 = t18.*t19.*t21.*t26.*t44.*t116.*1.294536862550567e-20;
t1043 = t24.*t25.*t26.*t44.*t116.*3.992732227073824e-24;
t1044 = t18.*t25.*t26.*t27.*t44.*t116.*5.902881824626087e-21;
t1045 = t19.*t24.*t26.*t27.*t44.*t116.*5.902881824626087e-21;
t1046 = t18.*t19.*t20.*t44.*t116.*5.999580612847032e-21;
t1048 = t18.*t21.*t25.*t26.*t44.*t116.*1.294536862550567e-20;
t1049 = t19.*t21.*t24.*t26.*t44.*t116.*1.294536862550567e-20;
t1050 = t24.*t25.*t26.*t27.*t44.*t116.*5.902881824626087e-21;
t1051 = t18.*t20.*t25.*t44.*t116.*5.999580612847032e-21;
t1052 = t19.*t20.*t24.*t44.*t116.*5.999580612847032e-21;
t1055 = t21.*t24.*t25.*t26.*t44.*t116.*1.294536862550567e-20;
t1056 = t20.*t24.*t25.*t44.*t116.*5.999580612847032e-21;
t1059 = t18.*t19.*t26.*t44.*t116.*6.715770285417749e-24;
t1063 = t18.*t25.*t26.*t44.*t116.*6.715770285417749e-24;
t1064 = t19.*t24.*t26.*t44.*t116.*6.715770285417749e-24;
t1065 = t24.*t25.*t26.*t44.*t116.*6.715770285417749e-24;
t43 = -t40;
t84 = t37+t38;
t87 = t39+t42;
t147 = -t139;
t155 = t146.^2;
t156 = t137-1.0;
t179 = t132./1.0e+8;
t190 = -t182;
t191 = -t184;
t192 = -t186;
t194 = -t187;
t199 = -t189;
t214 = -t203;
t218 = -t209;
t260 = t132.*5.84482e-3;
t261 = t131.*9.840000000000001e-6;
t262 = t133.*3.064357668490995e+34;
t264 = t132.*6.48e-5;
t266 = t11.*t132.*1.247162e-2;
t267 = t145.*5.84482e-3;
t268 = t46.*t133;
t273 = t16.*t132.*5.68686e-3;
t275 = t145.*6.48e-5;
t277 = t131.*5.78002e-3;
t278 = t132.*3.24e-6;
t279 = t131.*6.47e-6;
t280 = t132.*7.83e-6;
t281 = t132.*6.47e-6;
t282 = t132.*6.2e-7;
t305 = t143.*6.47e-6;
t306 = t76.*t133;
t307 = t77.*t133;
t310 = t78.*t133;
t312 = t79.*t133;
t314 = t80.*t133;
t329 = t20.*t22.*t133.*-3.315051378778914e+33;
t372 = t85.*t133;
t389 = t86.*t133;
t437 = t90.*t133;
t439 = t26.*t133.*-7.746286054220548e+49;
t441 = t97.*t133;
t445 = t99.*t133;
t446 = t98.*t133;
t448 = t20.*t27.*t133.*-7.290917220067534e+49;
t452 = t117.*t133;
t453 = t111.*t133;
t456 = t123.*t133;
t458 = t125.*t133;
t459 = t126.*t133;
t462 = t20.*t22.*t133.*-1.196628789628727e+53;
t463 = t115+t142;
t464 = t107+t139-1.0;
t467 = t133.*t144;
t470 = t133.*t149;
t471 = t133.*t141;
t474 = t133.*t151;
t475 = t133.*t153;
t479 = t26.*t28.*t44.*t133.*-1.325049802940888e+18i;
t480 = t136+t142+1.0;
t484 = t133.*t159;
t485 = t133.*t160;
t486 = t131.*3.311505989057797e-5;
t488 = t16.*t132.*2.906183788415621e-3;
t490 = t11.*t132.*6.373432765934105e-3;
t495 = t21.*t145.*1.35652563578e-4;
t506 = t27.*t145.*6.1855407534e-5;
t510 = t145.*7.0373543e-8;
t511 = t143.*6.2868699538e-5;
t523 = t133.*t211;
t530 = t133.*t215;
t539 = t133.*t223;
t544 = t20.*t44.*t133.*-4.394953650240249e+33i;
t554 = t133.*t227;
t562 = t133.*t231;
t563 = t21.*t26.*t44.*t133.*-1.03862462117543e+32i;
t566 = t133.*t232;
t568 = t133.*t235;
t569 = t133.*t236;
t571 = t26.*t44.*t133.*-3.97028021545552e+36i;
t574 = t133.*t245;
t585 = t133.*t244;
t590 = t21.*t26.*t28.*t44.*t133.*-3.315051378778914e+33i;
t602 = t133.*t252;
t611 = t133.*t248;
t615 = t133.*t250;
t623 = t21.*t22.*t26.*t44.*t133.*-6.099194893302011e+33i;
t629 = t26.*t28.*t44.*t133.*-1.249115114148252e+37i;
t632 = t133.*t255;
t637 = t133.*t254;
t638 = -t634;
t639 = -t635;
t644 = -t641;
t645 = -t642;
t650 = -t646;
t651 = -t648;
t653 = -t652;
t663 = -t658;
t664 = -t659;
t667 = -t660;
t672 = -t661;
t674 = -t668;
t683 = -t670;
t684 = -t671;
t685 = -t673;
t686 = -t677;
t687 = -t678;
t688 = -t679;
t689 = -t680;
t690 = -t681;
t699 = t143.*3.601891949238275e-7;
t702 = -t692;
t703 = -t693;
t704 = -t694;
t705 = t13.*t14.*t132.*1.509490621508912e-3;
t706 = -t698;
t708 = t8.*t9.*t16.*t131.*2.498039274760989e-3;
t709 = t8.*t9.*t11.*t131.*3.257046415933332e-3;
t711 = t8.*t14.*t16.*t131.*2.498039274760989e-3;
t712 = t9.*t13.*t16.*t131.*2.498039274760989e-3;
t713 = t8.*t11.*t14.*t131.*3.257046415933332e-3;
t714 = t9.*t11.*t13.*t131.*3.257046415933332e-3;
t717 = t8.*t9.*t11.*t131.*5.478347731418506e-3;
t718 = t13.*t14.*t16.*t131.*2.498039274760989e-3;
t719 = t11.*t13.*t14.*t131.*3.257046415933332e-3;
t721 = t8.*t9.*t16.*t131.*1.485161268617439e-3;
t722 = t8.*t11.*t14.*t131.*5.478347731418506e-3;
t723 = t9.*t11.*t13.*t131.*5.478347731418506e-3;
t724 = t8.*t14.*t16.*t131.*1.485161268617439e-3;
t725 = t9.*t13.*t16.*t131.*1.485161268617439e-3;
t726 = t11.*t13.*t14.*t131.*5.478347731418506e-3;
t727 = t13.*t14.*t16.*t131.*1.485161268617439e-3;
t732 = t8.*t9.*t132.*1.509490621508912e-3;
t733 = t8.*t14.*t132.*1.509490621508912e-3;
t734 = t9.*t13.*t132.*1.509490621508912e-3;
t738 = t8.*t9.*t131.*1.689683482265228e-6;
t739 = t8.*t14.*t131.*1.689683482265228e-6;
t740 = t9.*t13.*t131.*1.689683482265228e-6;
t741 = t13.*t14.*t131.*1.689683482265228e-6;
t743 = -t710;
t751 = -t728;
t752 = -t729;
t753 = -t730;
t754 = t27.*t145.*3.161027044821787e-5;
t756 = t21.*t145.*6.932319085178867e-5;
t758 = -t735;
t759 = -t736;
t760 = -t737;
t762 = t8.*t9.*t131.*2.842045365580232e-6;
t763 = t8.*t14.*t131.*2.842045365580232e-6;
t764 = t9.*t13.*t131.*2.842045365580232e-6;
t765 = t13.*t14.*t131.*2.842045365580232e-6;
t766 = t8.*t9.*t132.*2.538961213904336e-3;
t767 = t8.*t14.*t132.*2.538961213904336e-3;
t768 = t9.*t13.*t132.*2.538961213904336e-3;
t770 = t13.*t14.*t132.*2.538961213904336e-3;
t777 = (t10.*t44.*t83.*t108)./8.112963841460668e+31;
t778 = (t15.*t44.*t83.*t108)./8.112963841460668e+31;
t789 = -t784;
t792 = -t785;
t794 = -t786;
t796 = -t788;
t801 = -t790;
t804 = t20.*t44.*t116.*(t40-t41).*(-1.232595164407831e-32);
t806 = -t798;
t808 = t26.*t44.*t116.*(t40-t41).*(-1.232595164407831e-32);
t815 = -t803;
t816 = (t20.*t44.*t116.*(t40-t41))./8.112963841460668e+31;
t818 = -t810;
t821 = -t813;
t826 = -t820;
t827 = -t822;
t828 = -t823;
t840 = -t830;
t843 = -t831;
t853 = -t832;
t855 = t8.*t9.*t820;
t856 = -t836;
t857 = t8.*t14.*t820;
t858 = t9.*t13.*t820;
t859 = -t837;
t860 = -t838;
t861 = t13.*t14.*t820;
t863 = -t846;
t865 = -t848;
t866 = -t849;
t869 = -t850;
t878 = -t862;
t883 = -t864;
t884 = -t877;
t885 = -t879;
t886 = -t880;
t887 = -t881;
t888 = t468+2.61156643317655e-1;
t889 = t469+7.38843356682345e-1;
t890 = t476+2.61156643317655e-1;
t891 = t477+7.38843356682345e-1;
t900 = -t895;
t901 = -t897;
t902 = -t898;
t903 = -t899;
t912 = -t904;
t913 = -t910;
t914 = -t911;
t927 = -t919;
t928 = -t920;
t929 = -t921;
t930 = -t922;
t931 = -t925;
t932 = -t926;
t937 = t18.*t19.*t21.*t143.*3.542656816146526e-5;
t938 = t18.*t21.*t25.*t143.*3.542656816146526e-5;
t939 = t19.*t21.*t24.*t143.*3.542656816146526e-5;
t940 = t21.*t24.*t25.*t143.*3.542656816146526e-5;
t941 = t18.*t19.*t145.*1.641857854109028e-5;
t942 = t18.*t25.*t145.*1.641857854109028e-5;
t943 = t19.*t24.*t145.*1.641857854109028e-5;
t944 = t24.*t25.*t145.*1.641857854109028e-5;
t945 = t18.*t25.*t145.*2.761602722751607e-5;
t946 = t19.*t24.*t145.*2.761602722751607e-5;
t947 = t24.*t25.*t145.*2.761602722751607e-5;
t948 = t18.*t19.*t27.*t143.*1.615395060262503e-5;
t949 = t18.*t19.*t143.*1.837851826825065e-8;
t950 = t18.*t25.*t27.*t143.*1.615395060262503e-5;
t951 = t19.*t24.*t27.*t143.*1.615395060262503e-5;
t953 = t18.*t25.*t143.*1.837851826825065e-8;
t954 = t19.*t24.*t143.*1.837851826825065e-8;
t955 = t18.*t19.*t21.*t143.*5.958744043986595e-5;
t956 = t24.*t25.*t27.*t143.*1.615395060262503e-5;
t957 = t24.*t25.*t143.*1.837851826825065e-8;
t958 = t18.*t21.*t25.*t143.*5.958744043986595e-5;
t959 = t19.*t21.*t24.*t143.*5.958744043986595e-5;
t960 = t21.*t24.*t25.*t143.*5.958744043986595e-5;
t961 = t18.*t19.*t27.*t143.*2.71709233876478e-5;
t962 = t18.*t25.*t27.*t143.*2.71709233876478e-5;
t963 = t19.*t24.*t27.*t143.*2.71709233876478e-5;
t964 = t24.*t25.*t27.*t143.*2.71709233876478e-5;
t966 = t18.*t19.*t145.*2.761602722751607e-5;
t967 = t18.*t19.*t143.*3.091264323687963e-8;
t968 = t18.*t25.*t143.*3.091264323687963e-8;
t969 = t19.*t24.*t143.*3.091264323687963e-8;
t970 = t24.*t25.*t143.*3.091264323687963e-8;
t981 = t15.*t44.*t83.*t108.*7.204296868834178e-35;
t982 = t15.*t44.*t83.*t108.*7.987216665362745e-37;
t984 = t132+t633;
t989 = t10.*t44.*t83.*t108.*7.974890713718666e-38;
t997 = t145+t640;
t999 = t26.*t44.*t116.*(t40-t41).*(-7.204296868834178e-35);
t1003 = t26.*t44.*t116.*(t40-t41).*(-7.987216665362745e-37);
t1004 = t26.*t44.*t116.*(t40-t41).*7.204296868834178e-35;
t1008 = t20.*t44.*t116.*(t40-t41).*(-7.974890713718666e-38);
t1012 = t20.*t44.*t116.*(t40-t41).*7.974890713718666e-38;
t1016 = -t1011;
t1042 = -t1026;
t1047 = -t1027;
t1053 = -t1029;
t1054 = -t1030;
t1057 = -t1034;
t1058 = -t1035;
t1060 = -t1036;
t1061 = -t1037;
t1062 = -t1038;
t1066 = -t1046;
t1067 = -t1048;
t1068 = -t1049;
t1069 = -t1055;
t1070 = -t1063;
t1071 = -t1064;
t1072 = -t1065;
t1125 = t26.*t44.*t116.*(t40-t41).*(-2.081785322124547e-36);
t1129 = t26.*t44.*t116.*(t40-t41).*2.081785322124547e-36;
t1131 = t26.*t44.*t116.*(t40-t41).*(-8.687615694748404e-39);
t1134 = t20.*t44.*t116.*(t40-t41).*(-2.304459510155286e-39);
t1138 = t20.*t44.*t116.*(t40-t41).*2.304459510155286e-39;
H = ft_2({t10,t100,t1003,t1004,t1006,t1007,t101,t1012,t1016,t1017,t1018,t1019,t102,t1021,t1022,t1023,t1024,t1026,t1027,t1028,t103,t1031,t1032,t1033,t1034,t1035,t1040,t1042,t1043,t1044,t1045,t1047,t1048,t1049,t1050,t1051,t1052,t1053,t1054,t1056,t1057,t1058,t1059,t1060,t1061,t1062,t1063,t1064,t1066,t1067,t1068,t1069,t107,t1070,t1071,t1072,t108,t109,t11,t111,t112,t1125,t1129,t1131,t1134,t1138,t115,t116,t117,t119,t12,t123,t124,t125,t128,t130,t131,t132,t134,t135,t138,t143,t144,t145,t147,t148,t149,t15,t150,t152,t153,t154,t155,t156,t157,t16,t161,t162,t163,t164,t165,t166,t167,t168,t169,t17,t170,t172,t173,t174,t175,t176,t177,t179,t18,t180,t181,t183,t185,t188,t189,t190,t191,t192,t193,t194,t196,t197,t198,t199,t20,t200,t201,t202,t203,t205,t206,t207,t208,t21,t212,t214,t215,t216,t217,t218,t219,t22,t220,t221,t222,t225,t226,t227,t228,t230,t232,t233,t234,t238,t239,t24,t241,t242,t243,t245,t246,t247,t249,t250,t251,t252,t253,t256,t257,t258,t259,t26,t260,t261,t262,t264,t265,t266,t267,t268,t269,t27,t271,t272,t273,t274,t275,t276,t277,t278,t279,t28,t280,t281,t282,t284,t285,t286,t29,t290,t291,t292,t294,t295,t296,t297,t30,t300,t301,t302,t303,t304,t305,t307,t308,t309,t310,t312,t313,t314,t317,t318,t319,t32,t320,t321,t322,t323,t324,t325,t326,t328,t329,t33,t331,t332,t333,t334,t335,t336,t338,t339,t340,t341,t342,t343,t344,t345,t347,t348,t349,t350,t351,t352,t353,t354,t355,t356,t357,t358,t359,t36,t360,t361,t363,t365,t366,t367,t368,t37,t372,t373,t375,t376,t377,t378,t379,t380,t381,t382,t383,t384,t385,t386,t387,t389,t390,t391,t392,t393,t394,t395,t396,t397,t40,t400,t401,t402,t403,t404,t405,t406,t407,t408,t409,t41,t410,t411,t412,t414,t415,t416,t417,t419,t420,t421,t422,t423,t424,t425,t426,t427,t428,t429,t43,t430,t432,t433,t435,t436,t438,t439,t44,t440,t441,t442,t443,t445,t447,t448,t449,t45,t450,t452,t453,t455,t456,t457,t458,t46,t460,t462,t463,t464,t467,t47,t470,t471,t472,t473,t474,t479,t48,t480,t481,t482,t483,t484,t485,t486,t488,t49,t490,t493,t494,t495,t497,t498,t499,t50,t500,t501,t502,t503,t504,t505,t506,t507,t508,t509,t51,t510,t511,t512,t513,t514,t517,t518,t52,t520,t523,t524,t525,t528,t529,t531,t532,t533,t534,t535,t536,t537,t538,t539,t540,t541,t542,t543,t544,t545,t548,t549,t55,t550,t551,t552,t553,t556,t557,t558,t559,t56,t560,t561,t562,t563,t564,t567,t568,t569,t57,t570,t571,t575,t576,t577,t579,t58,t580,t581,t582,t583,t585,t587,t588,t589,t59,t590,t591,t594,t595,t596,t597,t598,t599,t60,t600,t603,t604,t605,t606,t607,t608,t609,t61,t610,t611,t612,t613,t614,t616,t617,t618,t619,t620,t621,t622,t623,t624,t625,t626,t627,t628,t629,t63,t630,t631,t632,t635,t636,t637,t638,t639,t64,t642,t643,t644,t645,t646,t647,t649,t65,t650,t651,t652,t653,t654,t655,t656,t657,t66,t662,t663,t664,t665,t666,t667,t669,t67,t670,t671,t672,t673,t674,t675,t676,t677,t678,t679,t68,t680,t681,t682,t683,t684,t685,t686,t687,t688,t689,t69,t690,t691,t692,t693,t694,t695,t696,t697,t699,t70,t700,t701,t702,t703,t704,t705,t706,t708,t709,t71,t711,t712,t713,t714,t715,t716,t717,t718,t719,t72,t720,t721,t722,t723,t724,t725,t726,t727,t728,t73,t731,t732,t733,t734,t735,t736,t738,t739,t74,t740,t741,t743,t75,t751,t752,t753,t754,t756,t757,t758,t759,t760,t762,t763,t764,t765,t766,t767,t768,t77,t770,t777,t778,t78,t781,t782,t783,t786,t787,t789,t79,t790,t791,t792,t793,t794,t795,t796,t8,t80,t800,t801,t802,t805,t806,t808,t809,t81,t811,t812,t814,t815,t816,t817,t818,t819,t82,t821,t824,t825,t826,t827,t828,t829,t83,t832,t833,t834,t835,t837,t838,t839,t840,t841,t842,t843,t844,t845,t847,t85,t850,t851,t852,t853,t854,t855,t856,t859,t86,t860,t861,t863,t864,t865,t866,t867,t868,t869,t87,t870,t871,t872,t873,t874,t875,t876,t878,t880,t881,t882,t883,t884,t885,t886,t887,t888,t889,t890,t891,t892,t893,t894,t895,t896,t897,t898,t9,t900,t901,t902,t903,t909,t91,t910,t911,t912,t913,t914,t915,t916,t917,t918,t919,t92,t920,t921,t922,t923,t924,t926,t927,t928,t929,t93,t930,t931,t932,t937,t938,t939,t940,t941,t942,t943,t944,t945,t946,t947,t948,t949,t95,t950,t951,t953,t954,t955,t956,t957,t958,t959,t96,t960,t961,t962,t963,t964,t966,t967,t968,t969,t97,t970,t981,t982,t983,t984,t986,t987,t989,t99,t990,t993,t997});
end
function H = ft_2(ct)
t10 = ct{1};
t100 = ct{2};
t1003 = ct{3};
t1004 = ct{4};
t1006 = ct{5};
t1007 = ct{6};
t101 = ct{7};
t1012 = ct{8};
t1016 = ct{9};
t1017 = ct{10};
t1018 = ct{11};
t1019 = ct{12};
t102 = ct{13};
t1021 = ct{14};
t1022 = ct{15};
t1023 = ct{16};
t1024 = ct{17};
t1026 = ct{18};
t1027 = ct{19};
t1028 = ct{20};
t103 = ct{21};
t1031 = ct{22};
t1032 = ct{23};
t1033 = ct{24};
t1034 = ct{25};
t1035 = ct{26};
t1040 = ct{27};
t1042 = ct{28};
t1043 = ct{29};
t1044 = ct{30};
t1045 = ct{31};
t1047 = ct{32};
t1048 = ct{33};
t1049 = ct{34};
t1050 = ct{35};
t1051 = ct{36};
t1052 = ct{37};
t1053 = ct{38};
t1054 = ct{39};
t1056 = ct{40};
t1057 = ct{41};
t1058 = ct{42};
t1059 = ct{43};
t1060 = ct{44};
t1061 = ct{45};
t1062 = ct{46};
t1063 = ct{47};
t1064 = ct{48};
t1066 = ct{49};
t1067 = ct{50};
t1068 = ct{51};
t1069 = ct{52};
t107 = ct{53};
t1070 = ct{54};
t1071 = ct{55};
t1072 = ct{56};
t108 = ct{57};
t109 = ct{58};
t11 = ct{59};
t111 = ct{60};
t112 = ct{61};
t1125 = ct{62};
t1129 = ct{63};
t1131 = ct{64};
t1134 = ct{65};
t1138 = ct{66};
t115 = ct{67};
t116 = ct{68};
t117 = ct{69};
t119 = ct{70};
t12 = ct{71};
t123 = ct{72};
t124 = ct{73};
t125 = ct{74};
t128 = ct{75};
t130 = ct{76};
t131 = ct{77};
t132 = ct{78};
t134 = ct{79};
t135 = ct{80};
t138 = ct{81};
t143 = ct{82};
t144 = ct{83};
t145 = ct{84};
t147 = ct{85};
t148 = ct{86};
t149 = ct{87};
t15 = ct{88};
t150 = ct{89};
t152 = ct{90};
t153 = ct{91};
t154 = ct{92};
t155 = ct{93};
t156 = ct{94};
t157 = ct{95};
t16 = ct{96};
t161 = ct{97};
t162 = ct{98};
t163 = ct{99};
t164 = ct{100};
t165 = ct{101};
t166 = ct{102};
t167 = ct{103};
t168 = ct{104};
t169 = ct{105};
t17 = ct{106};
t170 = ct{107};
t172 = ct{108};
t173 = ct{109};
t174 = ct{110};
t175 = ct{111};
t176 = ct{112};
t177 = ct{113};
t179 = ct{114};
t18 = ct{115};
t180 = ct{116};
t181 = ct{117};
t183 = ct{118};
t185 = ct{119};
t188 = ct{120};
t189 = ct{121};
t190 = ct{122};
t191 = ct{123};
t192 = ct{124};
t193 = ct{125};
t194 = ct{126};
t196 = ct{127};
t197 = ct{128};
t198 = ct{129};
t199 = ct{130};
t20 = ct{131};
t200 = ct{132};
t201 = ct{133};
t202 = ct{134};
t203 = ct{135};
t205 = ct{136};
t206 = ct{137};
t207 = ct{138};
t208 = ct{139};
t21 = ct{140};
t212 = ct{141};
t214 = ct{142};
t215 = ct{143};
t216 = ct{144};
t217 = ct{145};
t218 = ct{146};
t219 = ct{147};
t22 = ct{148};
t220 = ct{149};
t221 = ct{150};
t222 = ct{151};
t225 = ct{152};
t226 = ct{153};
t227 = ct{154};
t228 = ct{155};
t230 = ct{156};
t232 = ct{157};
t233 = ct{158};
t234 = ct{159};
t238 = ct{160};
t239 = ct{161};
t24 = ct{162};
t241 = ct{163};
t242 = ct{164};
t243 = ct{165};
t245 = ct{166};
t246 = ct{167};
t247 = ct{168};
t249 = ct{169};
t250 = ct{170};
t251 = ct{171};
t252 = ct{172};
t253 = ct{173};
t256 = ct{174};
t257 = ct{175};
t258 = ct{176};
t259 = ct{177};
t26 = ct{178};
t260 = ct{179};
t261 = ct{180};
t262 = ct{181};
t264 = ct{182};
t265 = ct{183};
t266 = ct{184};
t267 = ct{185};
t268 = ct{186};
t269 = ct{187};
t27 = ct{188};
t271 = ct{189};
t272 = ct{190};
t273 = ct{191};
t274 = ct{192};
t275 = ct{193};
t276 = ct{194};
t277 = ct{195};
t278 = ct{196};
t279 = ct{197};
t28 = ct{198};
t280 = ct{199};
t281 = ct{200};
t282 = ct{201};
t284 = ct{202};
t285 = ct{203};
t286 = ct{204};
t29 = ct{205};
t290 = ct{206};
t291 = ct{207};
t292 = ct{208};
t294 = ct{209};
t295 = ct{210};
t296 = ct{211};
t297 = ct{212};
t30 = ct{213};
t300 = ct{214};
t301 = ct{215};
t302 = ct{216};
t303 = ct{217};
t304 = ct{218};
t305 = ct{219};
t307 = ct{220};
t308 = ct{221};
t309 = ct{222};
t310 = ct{223};
t312 = ct{224};
t313 = ct{225};
t314 = ct{226};
t317 = ct{227};
t318 = ct{228};
t319 = ct{229};
t32 = ct{230};
t320 = ct{231};
t321 = ct{232};
t322 = ct{233};
t323 = ct{234};
t324 = ct{235};
t325 = ct{236};
t326 = ct{237};
t328 = ct{238};
t329 = ct{239};
t33 = ct{240};
t331 = ct{241};
t332 = ct{242};
t333 = ct{243};
t334 = ct{244};
t335 = ct{245};
t336 = ct{246};
t338 = ct{247};
t339 = ct{248};
t340 = ct{249};
t341 = ct{250};
t342 = ct{251};
t343 = ct{252};
t344 = ct{253};
t345 = ct{254};
t347 = ct{255};
t348 = ct{256};
t349 = ct{257};
t350 = ct{258};
t351 = ct{259};
t352 = ct{260};
t353 = ct{261};
t354 = ct{262};
t355 = ct{263};
t356 = ct{264};
t357 = ct{265};
t358 = ct{266};
t359 = ct{267};
t36 = ct{268};
t360 = ct{269};
t361 = ct{270};
t363 = ct{271};
t365 = ct{272};
t366 = ct{273};
t367 = ct{274};
t368 = ct{275};
t37 = ct{276};
t372 = ct{277};
t373 = ct{278};
t375 = ct{279};
t376 = ct{280};
t377 = ct{281};
t378 = ct{282};
t379 = ct{283};
t380 = ct{284};
t381 = ct{285};
t382 = ct{286};
t383 = ct{287};
t384 = ct{288};
t385 = ct{289};
t386 = ct{290};
t387 = ct{291};
t389 = ct{292};
t390 = ct{293};
t391 = ct{294};
t392 = ct{295};
t393 = ct{296};
t394 = ct{297};
t395 = ct{298};
t396 = ct{299};
t397 = ct{300};
t40 = ct{301};
t400 = ct{302};
t401 = ct{303};
t402 = ct{304};
t403 = ct{305};
t404 = ct{306};
t405 = ct{307};
t406 = ct{308};
t407 = ct{309};
t408 = ct{310};
t409 = ct{311};
t41 = ct{312};
t410 = ct{313};
t411 = ct{314};
t412 = ct{315};
t414 = ct{316};
t415 = ct{317};
t416 = ct{318};
t417 = ct{319};
t419 = ct{320};
t420 = ct{321};
t421 = ct{322};
t422 = ct{323};
t423 = ct{324};
t424 = ct{325};
t425 = ct{326};
t426 = ct{327};
t427 = ct{328};
t428 = ct{329};
t429 = ct{330};
t43 = ct{331};
t430 = ct{332};
t432 = ct{333};
t433 = ct{334};
t435 = ct{335};
t436 = ct{336};
t438 = ct{337};
t439 = ct{338};
t44 = ct{339};
t440 = ct{340};
t441 = ct{341};
t442 = ct{342};
t443 = ct{343};
t445 = ct{344};
t447 = ct{345};
t448 = ct{346};
t449 = ct{347};
t45 = ct{348};
t450 = ct{349};
t452 = ct{350};
t453 = ct{351};
t455 = ct{352};
t456 = ct{353};
t457 = ct{354};
t458 = ct{355};
t46 = ct{356};
t460 = ct{357};
t462 = ct{358};
t463 = ct{359};
t464 = ct{360};
t467 = ct{361};
t47 = ct{362};
t470 = ct{363};
t471 = ct{364};
t472 = ct{365};
t473 = ct{366};
t474 = ct{367};
t479 = ct{368};
t48 = ct{369};
t480 = ct{370};
t481 = ct{371};
t482 = ct{372};
t483 = ct{373};
t484 = ct{374};
t485 = ct{375};
t486 = ct{376};
t488 = ct{377};
t49 = ct{378};
t490 = ct{379};
t493 = ct{380};
t494 = ct{381};
t495 = ct{382};
t497 = ct{383};
t498 = ct{384};
t499 = ct{385};
t50 = ct{386};
t500 = ct{387};
t501 = ct{388};
t502 = ct{389};
t503 = ct{390};
t504 = ct{391};
t505 = ct{392};
t506 = ct{393};
t507 = ct{394};
t508 = ct{395};
t509 = ct{396};
t51 = ct{397};
t510 = ct{398};
t511 = ct{399};
t512 = ct{400};
t513 = ct{401};
t514 = ct{402};
t517 = ct{403};
t518 = ct{404};
t52 = ct{405};
t520 = ct{406};
t523 = ct{407};
t524 = ct{408};
t525 = ct{409};
t528 = ct{410};
t529 = ct{411};
t531 = ct{412};
t532 = ct{413};
t533 = ct{414};
t534 = ct{415};
t535 = ct{416};
t536 = ct{417};
t537 = ct{418};
t538 = ct{419};
t539 = ct{420};
t540 = ct{421};
t541 = ct{422};
t542 = ct{423};
t543 = ct{424};
t544 = ct{425};
t545 = ct{426};
t548 = ct{427};
t549 = ct{428};
t55 = ct{429};
t550 = ct{430};
t551 = ct{431};
t552 = ct{432};
t553 = ct{433};
t556 = ct{434};
t557 = ct{435};
t558 = ct{436};
t559 = ct{437};
t56 = ct{438};
t560 = ct{439};
t561 = ct{440};
t562 = ct{441};
t563 = ct{442};
t564 = ct{443};
t567 = ct{444};
t568 = ct{445};
t569 = ct{446};
t57 = ct{447};
t570 = ct{448};
t571 = ct{449};
t575 = ct{450};
t576 = ct{451};
t577 = ct{452};
t579 = ct{453};
t58 = ct{454};
t580 = ct{455};
t581 = ct{456};
t582 = ct{457};
t583 = ct{458};
t585 = ct{459};
t587 = ct{460};
t588 = ct{461};
t589 = ct{462};
t59 = ct{463};
t590 = ct{464};
t591 = ct{465};
t594 = ct{466};
t595 = ct{467};
t596 = ct{468};
t597 = ct{469};
t598 = ct{470};
t599 = ct{471};
t60 = ct{472};
t600 = ct{473};
t603 = ct{474};
t604 = ct{475};
t605 = ct{476};
t606 = ct{477};
t607 = ct{478};
t608 = ct{479};
t609 = ct{480};
t61 = ct{481};
t610 = ct{482};
t611 = ct{483};
t612 = ct{484};
t613 = ct{485};
t614 = ct{486};
t616 = ct{487};
t617 = ct{488};
t618 = ct{489};
t619 = ct{490};
t620 = ct{491};
t621 = ct{492};
t622 = ct{493};
t623 = ct{494};
t624 = ct{495};
t625 = ct{496};
t626 = ct{497};
t627 = ct{498};
t628 = ct{499};
t629 = ct{500};
t63 = ct{501};
t630 = ct{502};
t631 = ct{503};
t632 = ct{504};
t635 = ct{505};
t636 = ct{506};
t637 = ct{507};
t638 = ct{508};
t639 = ct{509};
t64 = ct{510};
t642 = ct{511};
t643 = ct{512};
t644 = ct{513};
t645 = ct{514};
t646 = ct{515};
t647 = ct{516};
t649 = ct{517};
t65 = ct{518};
t650 = ct{519};
t651 = ct{520};
t652 = ct{521};
t653 = ct{522};
t654 = ct{523};
t655 = ct{524};
t656 = ct{525};
t657 = ct{526};
t66 = ct{527};
t662 = ct{528};
t663 = ct{529};
t664 = ct{530};
t665 = ct{531};
t666 = ct{532};
t667 = ct{533};
t669 = ct{534};
t67 = ct{535};
t670 = ct{536};
t671 = ct{537};
t672 = ct{538};
t673 = ct{539};
t674 = ct{540};
t675 = ct{541};
t676 = ct{542};
t677 = ct{543};
t678 = ct{544};
t679 = ct{545};
t68 = ct{546};
t680 = ct{547};
t681 = ct{548};
t682 = ct{549};
t683 = ct{550};
t684 = ct{551};
t685 = ct{552};
t686 = ct{553};
t687 = ct{554};
t688 = ct{555};
t689 = ct{556};
t69 = ct{557};
t690 = ct{558};
t691 = ct{559};
t692 = ct{560};
t693 = ct{561};
t694 = ct{562};
t695 = ct{563};
t696 = ct{564};
t697 = ct{565};
t699 = ct{566};
t70 = ct{567};
t700 = ct{568};
t701 = ct{569};
t702 = ct{570};
t703 = ct{571};
t704 = ct{572};
t705 = ct{573};
t706 = ct{574};
t708 = ct{575};
t709 = ct{576};
t71 = ct{577};
t711 = ct{578};
t712 = ct{579};
t713 = ct{580};
t714 = ct{581};
t715 = ct{582};
t716 = ct{583};
t717 = ct{584};
t718 = ct{585};
t719 = ct{586};
t72 = ct{587};
t720 = ct{588};
t721 = ct{589};
t722 = ct{590};
t723 = ct{591};
t724 = ct{592};
t725 = ct{593};
t726 = ct{594};
t727 = ct{595};
t728 = ct{596};
t73 = ct{597};
t731 = ct{598};
t732 = ct{599};
t733 = ct{600};
t734 = ct{601};
t735 = ct{602};
t736 = ct{603};
t738 = ct{604};
t739 = ct{605};
t74 = ct{606};
t740 = ct{607};
t741 = ct{608};
t743 = ct{609};
t75 = ct{610};
t751 = ct{611};
t752 = ct{612};
t753 = ct{613};
t754 = ct{614};
t756 = ct{615};
t757 = ct{616};
t758 = ct{617};
t759 = ct{618};
t760 = ct{619};
t762 = ct{620};
t763 = ct{621};
t764 = ct{622};
t765 = ct{623};
t766 = ct{624};
t767 = ct{625};
t768 = ct{626};
t77 = ct{627};
t770 = ct{628};
t777 = ct{629};
t778 = ct{630};
t78 = ct{631};
t781 = ct{632};
t782 = ct{633};
t783 = ct{634};
t786 = ct{635};
t787 = ct{636};
t789 = ct{637};
t79 = ct{638};
t790 = ct{639};
t791 = ct{640};
t792 = ct{641};
t793 = ct{642};
t794 = ct{643};
t795 = ct{644};
t796 = ct{645};
t8 = ct{646};
t80 = ct{647};
t800 = ct{648};
t801 = ct{649};
t802 = ct{650};
t805 = ct{651};
t806 = ct{652};
t808 = ct{653};
t809 = ct{654};
t81 = ct{655};
t811 = ct{656};
t812 = ct{657};
t814 = ct{658};
t815 = ct{659};
t816 = ct{660};
t817 = ct{661};
t818 = ct{662};
t819 = ct{663};
t82 = ct{664};
t821 = ct{665};
t824 = ct{666};
t825 = ct{667};
t826 = ct{668};
t827 = ct{669};
t828 = ct{670};
t829 = ct{671};
t83 = ct{672};
t832 = ct{673};
t833 = ct{674};
t834 = ct{675};
t835 = ct{676};
t837 = ct{677};
t838 = ct{678};
t839 = ct{679};
t840 = ct{680};
t841 = ct{681};
t842 = ct{682};
t843 = ct{683};
t844 = ct{684};
t845 = ct{685};
t847 = ct{686};
t85 = ct{687};
t850 = ct{688};
t851 = ct{689};
t852 = ct{690};
t853 = ct{691};
t854 = ct{692};
t855 = ct{693};
t856 = ct{694};
t859 = ct{695};
t86 = ct{696};
t860 = ct{697};
t861 = ct{698};
t863 = ct{699};
t864 = ct{700};
t865 = ct{701};
t866 = ct{702};
t867 = ct{703};
t868 = ct{704};
t869 = ct{705};
t87 = ct{706};
t870 = ct{707};
t871 = ct{708};
t872 = ct{709};
t873 = ct{710};
t874 = ct{711};
t875 = ct{712};
t876 = ct{713};
t878 = ct{714};
t880 = ct{715};
t881 = ct{716};
t882 = ct{717};
t883 = ct{718};
t884 = ct{719};
t885 = ct{720};
t886 = ct{721};
t887 = ct{722};
t888 = ct{723};
t889 = ct{724};
t890 = ct{725};
t891 = ct{726};
t892 = ct{727};
t893 = ct{728};
t894 = ct{729};
t895 = ct{730};
t896 = ct{731};
t897 = ct{732};
t898 = ct{733};
t9 = ct{734};
t900 = ct{735};
t901 = ct{736};
t902 = ct{737};
t903 = ct{738};
t909 = ct{739};
t91 = ct{740};
t910 = ct{741};
t911 = ct{742};
t912 = ct{743};
t913 = ct{744};
t914 = ct{745};
t915 = ct{746};
t916 = ct{747};
t917 = ct{748};
t918 = ct{749};
t919 = ct{750};
t92 = ct{751};
t920 = ct{752};
t921 = ct{753};
t922 = ct{754};
t923 = ct{755};
t924 = ct{756};
t926 = ct{757};
t927 = ct{758};
t928 = ct{759};
t929 = ct{760};
t93 = ct{761};
t930 = ct{762};
t931 = ct{763};
t932 = ct{764};
t937 = ct{765};
t938 = ct{766};
t939 = ct{767};
t940 = ct{768};
t941 = ct{769};
t942 = ct{770};
t943 = ct{771};
t944 = ct{772};
t945 = ct{773};
t946 = ct{774};
t947 = ct{775};
t948 = ct{776};
t949 = ct{777};
t95 = ct{778};
t950 = ct{779};
t951 = ct{780};
t953 = ct{781};
t954 = ct{782};
t955 = ct{783};
t956 = ct{784};
t957 = ct{785};
t958 = ct{786};
t959 = ct{787};
t96 = ct{788};
t960 = ct{789};
t961 = ct{790};
t962 = ct{791};
t963 = ct{792};
t964 = ct{793};
t966 = ct{794};
t967 = ct{795};
t968 = ct{796};
t969 = ct{797};
t97 = ct{798};
t970 = ct{799};
t981 = ct{800};
t982 = ct{801};
t983 = ct{802};
t984 = ct{803};
t986 = ct{804};
t987 = ct{805};
t989 = ct{806};
t99 = ct{807};
t990 = ct{808};
t993 = ct{809};
t997 = ct{810};
t1176 = t44.*t107.*t116.*(t40-t41).*(-2.711709361697228e-39);
t1633 = t45+t57+t63+t65+t66+t67+t74+t81+t128+t138+t148+t152+t154+t258+t259+t265+t269+t271+t272+t274+t276+t295+t455+t457+t460+t472+t473+3.064357668490995e+34;
t1638 = t92+t95+t100+t103+t193+t217+t221+t222+t225+t226+t233+t243+t433+t435+t438+t440+t501+t512+t525+t528+t535+t536+t537+t557;
t1685 = t91+t96+t102+t109+t112+t119+t124+t219+t230+t234+t239+t246+t249+t251+t432+t436+t442+t443+t447+t449+t450+t494+t531+t564+t567+t570+t579+t580;
t88 = t41+t43;
t158 = t156.^2;
t270 = -t264;
t283 = -t273;
t288 = -t275;
t293 = -t277;
t461 = t107+t147;
t478 = t464.^2;
t487 = t480.^2;
t489 = -t486;
t491 = -t490;
t519 = -t506;
t522 = -t511;
t707 = -t699;
t742 = -t709;
t744 = -t717;
t745 = -t718;
t746 = -t722;
t747 = -t723;
t748 = -t724;
t749 = -t725;
t750 = -t727;
t755 = -t732;
t761 = -t738;
t769 = -t756;
t771 = -t762;
t772 = -t763;
t773 = -t764;
t774 = -t766;
t775 = -t767;
t776 = -t768;
t780 = -t778;
t797 = (t20.*t44.*t87.*t116)./8.112963841460668e+31;
t799 = (t26.*t44.*t87.*t116)./8.112963841460668e+31;
t905 = t29.*t888;
t906 = t29.*t889;
t907 = t30.*t888;
t908 = t30.*t889;
t933 = t32.*t890;
t934 = t32.*t891;
t935 = t33.*t890;
t936 = t33.*t891;
t952 = -t940;
t965 = -t944;
t971 = -t948;
t972 = -t950;
t973 = -t951;
t974 = -t955;
t975 = -t957;
t976 = -t962;
t977 = -t963;
t978 = -t964;
t979 = -t966;
t980 = -t967;
t985 = -t982;
t988 = t131+t638;
t991 = t12.*t984;
t992 = t17.*t984;
t994 = t26.*t44.*t87.*t116.*7.204296868834178e-35;
t998 = t26.*t44.*t87.*t116.*7.987216665362745e-37;
t1001 = t143+t644;
t1005 = t20.*t44.*t87.*t116.*7.974890713718666e-38;
t1009 = t22.*t997;
t1010 = t28.*t997;
t1073 = t29.*t130.*t155.*2.79634861451666e-3;
t1074 = t30.*t130.*t155.*2.79634861451666e-3;
t1081 = t29.*t130.*t155.*1.44134945686578e-2;
t1083 = t30.*t130.*t155.*1.44134945686578e-2;
t1122 = t26.*t44.*t87.*t116.*2.081785322124547e-36;
t1126 = t26.*t44.*t87.*t116.*8.687615694748404e-39;
t1132 = t20.*t44.*t87.*t116.*2.304459510155286e-39;
t1174 = t44.*t87.*t107.*t116.*2.711709361697228e-39;
t1177 = t261+t789;
t1207 = t44.*t116.*t984.*9.543032792050485e-25;
t1216 = t44.*t116.*t984.*5.916680331071301e-23;
t1218 = t44.*t116.*t984.*3.091942624624357e-22;
t1219 = t44.*t116.*t984.*7.472194676175529e-22;
t1236 = (t984.*t997)./1.0e+8;
t1238 = t984.*t997.*6.2e-7;
t1239 = t280+t800+t815;
t1240 = t278+t809+t821;
t1404 = t260+t279+t792+t793+t826;
t1408 = t267+t305+t796+t812+t840;
t1462 = t292+t296+t297+t303+t657+t665+t666+t667;
t1463 = t290+t291+t294+t308+t662+t663+t664+t674;
t1469 = t50+t51+t285+t286+t302+t309+t657+t665+t666+t667;
t1470 = t48+t61+t284+t300+t301+t304+t662+t663+t664+t674;
t1530 = t500+t507+t508+t513+t893+t894+t896+t903;
t1531 = t497+t498+t505+t509+t892+t900+t901+t902;
t1551 = t163+t166+t502+t503+t520+t524+t893+t894+t896+t903;
t1552 = t165+t167+t499+t514+t517+t518+t892+t900+t901+t902;
t1634 = t46+t77+t78+t79+t80+t82+t85+t86+t150+t153+t157+t161+t162+t262+t268+t307+t310+t312+t314+t329+t372+t389+t471+t474+t479+t484+t485+3.064357668490995e+34;
t1660 = t97+t101+t111+t125+t220+t227+t228+t238+t241+t242+t245+t252+t441+t448+t453+t458+t523+t539+t562+t563+t568+t569+t590+t623;
t1692 = t93+t99+t117+t123+t135+t144+t149+t215+t232+t247+t250+t253+t256+t257+t439+t445+t452+t456+t462+t467+t470+t544+t571+t585+t611+t629+t632+t637;
t807 = -t799;
t995 = t11.*t988;
t996 = t16.*t988;
t1000 = -t992;
t1002 = -t998;
t1013 = t21.*t1001;
t1014 = t27.*t1001;
t1075 = t905.*5.110348748545983e-1;
t1076 = -t1073;
t1077 = t907.*5.110348748545983e-1;
t1078 = -t1074;
t1079 = t906.*8.595599785252598e-1;
t1082 = t908.*8.595599785252598e-1;
t1084 = t905.*2.311164e-2;
t1085 = t907.*2.311164e-2;
t1086 = -t1081;
t1087 = t906.*1.273194e-2;
t1088 = -t1083;
t1089 = t905.*4.251385e-2;
t1090 = t908.*1.273194e-2;
t1091 = t907.*4.251385e-2;
t1094 = t933.*5.110348748545983e-1;
t1095 = t905.*6.562549e-2;
t1097 = t935.*5.110348748545983e-1;
t1098 = t907.*6.562549e-2;
t1100 = t32.*t134.*t158.*2.79634861451666e-3;
t1101 = t33.*t134.*t158.*2.79634861451666e-3;
t1103 = t934.*8.595599785252598e-1;
t1105 = t936.*8.595599785252598e-1;
t1108 = t934.*1.273194e-2;
t1109 = t933.*4.251385e-2;
t1110 = t936.*1.273194e-2;
t1111 = t935.*4.251385e-2;
t1112 = t32.*t134.*t158.*1.44134945686578e-2;
t1113 = t33.*t134.*t158.*1.44134945686578e-2;
t1115 = t933.*6.562549e-2;
t1117 = t935.*6.562549e-2;
t1123 = t991.*9.99471e-3;
t1124 = t992.*1.838876e-2;
t1136 = t991.*9.3e-7;
t1137 = t992.*1.02e-6;
t1140 = t1009.*9.99471e-3;
t1141 = t1010.*1.838876e-2;
t1146 = t991.*9.0e-8;
t1148 = t992.*9.0e-8;
t1159 = t32.*t134.*t158.*2.032204410370765e-5;
t1160 = t33.*t134.*t158.*2.032204410370765e-5;
t1163 = t933.*6.678441185616e-4;
t1164 = t935.*6.678441185616e-4;
t1165 = t934.*9.2527464159e-5;
t1166 = t936.*9.2527464159e-5;
t1167 = t32.*t134.*t158.*1.047479097535352e-4;
t1168 = t33.*t134.*t158.*1.047479097535352e-4;
t1171 = t933.*4.769234047515e-4;
t1172 = t935.*4.769234047515e-4;
t1175 = -t1174;
t1178 = t29.*t461.*t478.*2.196325630278387e-1;
t1179 = t30.*t461.*t478.*2.196325630278387e-1;
t1182 = t33.*t463.*t487.*2.196325630278387e-1;
t1183 = t32.*t463.*t487.*2.196325630278387e-1;
t1186 = t29.*t461.*t478.*1.122398993609262e-1;
t1187 = t30.*t461.*t478.*1.122398993609262e-1;
t1190 = t29.*t461.*t478.*1.887873611596568e-1;
t1191 = t30.*t461.*t478.*1.887873611596568e-1;
t1193 = t29.*t461.*t478.*5.076068728976717e-3;
t1194 = t30.*t461.*t478.*5.076068728976717e-3;
t1196 = t32.*t463.*t487.*1.122398993609262e-1;
t1197 = t33.*t463.*t487.*1.122398993609262e-1;
t1200 = t32.*t463.*t487.*1.887873611596568e-1;
t1201 = t33.*t463.*t487.*1.887873611596568e-1;
t1202 = t32.*t463.*t487.*5.076068728976717e-3;
t1203 = t33.*t463.*t487.*5.076068728976717e-3;
t1215 = t44.*t116.*t988.*9.390344267377678e-22;
t1217 = t32.*t463.*t487.*1.46680315462752e-4;
t1220 = t33.*t463.*t487.*1.46680315462752e-4;
t1221 = -t1218;
t1222 = -t1219;
t1241 = t1001.*t1177;
t1334 = t44.*t116.*t1240.*9.543032792050485e-17;
t1344 = t997.*t1239;
t1471 = t266+t281+t283+t293+t805+t817+t818+t819;
t1488 = t481+t482+t483+t488+t489+t491+t647+t649+t651;
t1546 = t495+t510+t519+t522+t1006+t1007+t1016+t1017;
t1554 = t682+t700+t701+t707+t754+t769+t839+t854+t878;
t1822 = t378+t379+t394+t401+t404+t405+t407+t408+t410+t415+t421+t422+t424+t426+t427+t428+t708+t713+t714+t726+t733+t734+t739+t740+t744+t745+t748+t749+t765+t770+t771+t774+t833+t834+t841+t842+t856+t863+t865+t866+t867+t868+t871+t872+t873+t882+t884+t885;
t1823 = t384+t385+t395+t396+t397+t406+t409+t411+t412+t414+t416+t417+t419+t423+t429+t430+t705+t711+t712+t719+t721+t741+t742+t746+t747+t750+t755+t761+t772+t773+t775+t776+t835+t844+t845+t847+t853+t855+t859+t860+t869+t870+t874+t875+t876+t883+t886+t887;
t1858 = t575+t581+t589+t594+t600+t604+t605+t609+t612+t613+t614+t618+t619+t622+t626+t627+t938+t939+t942+t943+t947+t953+t954+t960+t961+t970+t972+t973+t974+t978+t979+t980+t1023+t1024+t1031+t1032+t1040+t1050+t1053+t1054+t1056+t1059+t1060+t1061+t1062+t1066+t1069+t1072;
t1859 = t587+t588+t595+t596+t597+t603+t607+t608+t610+t617+t620+t621+t624+t625+t630+t631+t937+t941+t945+t946+t949+t952+t956+t958+t959+t965+t968+t969+t971+t975+t976+t977+t1022+t1028+t1033+t1042+t1043+t1044+t1045+t1047+t1051+t1052+t1057+t1058+t1067+t1068+t1070+t1071;
t1015 = t996.*(3.0./5.0e+2);
t1025 = t1014.*(3.0./5.0e+2);
t1041 = t995./1.0e+8;
t1080 = -t1077;
t1092 = -t1084;
t1093 = -t1087;
t1096 = -t1090;
t1099 = -t1091;
t1102 = -t1095;
t1104 = -t1097;
t1106 = -t1100;
t1107 = -t1101;
t1114 = -t1108;
t1116 = -t1110;
t1118 = -t1111;
t1119 = -t1112;
t1120 = -t1113;
t1121 = -t1115;
t1127 = -t1123;
t1128 = -t1124;
t1130 = t995.*1.247162e-2;
t1133 = t996.*5.68686e-3;
t1139 = t996.*3.131399999999998e-4;
t1142 = t996.*5.7e-7;
t1143 = t995.*1.02e-6;
t1144 = -t1137;
t1145 = -t1140;
t1147 = -t1141;
t1150 = t995.*2.4e-7;
t1151 = t1013.*1.247162e-2;
t1152 = -t1148;
t1153 = t1014.*5.68686e-3;
t1154 = t995.*4.0e-8;
t1155 = t996.*4.0e-8;
t1158 = t1014.*3.131399999999998e-4;
t1161 = -t1159;
t1162 = -t1160;
t1169 = -t1163;
t1170 = -t1165;
t1173 = -t1168;
t1180 = -t1178;
t1181 = -t1179;
t1184 = -t1182;
t1185 = -t1183;
t1188 = -t1186;
t1189 = -t1187;
t1192 = -t1190;
t1195 = -t1194;
t1198 = -t1196;
t1199 = -t1197;
t1204 = -t1200;
t1205 = t636+t995;
t1206 = t639+t996;
t1208 = -t12.*(t635-t996);
t1209 = -t17.*(t635-t996);
t1210 = t643+t1013;
t1211 = t645+t1014;
t1212 = -t22.*(t642-t1014);
t1213 = -t28.*(t642-t1014);
t1214 = t22.*(t642-t1014);
t1223 = -t1220;
t1224 = t17.*(t635-t996).*(-9.99471e-3);
t1225 = t12.*(t635-t996).*(-1.838876e-2);
t1226 = t17.*(t635-t996).*9.99471e-3;
t1227 = t12.*(t635-t996).*1.838876e-2;
t1228 = t12.*(t635-t996).*(-1.02e-6);
t1229 = t17.*(t635-t996).*(-9.3e-7);
t1230 = t12.*(t635-t996).*(-9.0e-8);
t1231 = t17.*(t635-t996).*(-9.0e-8);
t1232 = t28.*(t642-t1014).*(-9.99471e-3);
t1234 = t28.*(t642-t1014).*9.99471e-3;
t1242 = t906+t1179;
t1243 = t907+t1178;
t1258 = t934+t1182;
t1259 = t935+t1183;
t1276 = t44.*t116.*(t635-t996).*(-5.439528691468777e-23);
t1278 = t44.*t116.*(t635-t996).*5.439528691468777e-23;
t1279 = t44.*t116.*(t635-t996).*(-3.817213116820194e-24);
t1280 = t44.*t116.*(t635-t996).*3.817213116820194e-24;
t1335 = -t1334;
t1337 = t997.*(t635-t996).*(-5.7e-7);
t1339 = t997.*(t635-t996).*5.7e-7;
t1341 = t997.*(t635-t996).*(-4.0e-8);
t1342 = t997.*(t635-t996).*4.0e-8;
t1423 = t44.*t116.*(t992+t12.*(t635-t996)).*(-9.733893447891495e-23);
t1425 = t44.*t116.*(t992+t12.*(t635-t996)).*9.733893447891495e-23;
t1427 = t44.*t116.*(t992+t12.*(t635-t996)).*(-8.588729512845436e-24);
t1428 = t44.*t116.*(t992+t12.*(t635-t996)).*8.588729512845436e-24;
t1445 = t997.*(t992+t12.*(t635-t996)).*(-1.02e-6);
t1446 = t997.*(t992+t12.*(t635-t996)).*(-9.0e-8);
t1543 = t44.*t83.*t108.*(t1097-t1103+t1196-t1201).*(-2.711709361697228e-39);
t1020 = -t1015;
t1039 = -t1025;
t1135 = -t1133;
t1149 = -t1142;
t1156 = -t1153;
t1157 = -t1155;
t1233 = t1214.*(-1.838876e-2);
t1235 = t1214.*1.838876e-2;
t1237 = t825+t1143;
t1244 = t905+t1181;
t1245 = t908+t1180;
t1246 = t44.*t116.*t1205.*9.543032792050485e-25;
t1247 = t10.*t1242;
t1248 = t11.*t1243;
t1249 = t15.*t1242;
t1250 = t16.*t1243;
t1260 = t933+t1184;
t1261 = t936+t1185;
t1262 = t20.*t1258;
t1263 = t21.*t1259;
t1264 = t26.*t1258;
t1265 = t27.*t1259;
t1274 = t44.*t116.*t1205.*9.733893447891495e-23;
t1275 = t44.*t116.*t1205.*2.290327870092116e-23;
t1277 = t44.*t116.*t1205.*3.817213116820194e-24;
t1315 = t991+t1209;
t1316 = t1000+t1208;
t1317 = (t997.*t1205)./1.0e+8;
t1318 = t1009+t1213;
t1319 = t1010+t1214;
t1336 = t997.*t1205.*1.02e-6;
t1338 = t997.*t1205.*2.4e-7;
t1340 = t997.*t1205.*4.0e-8;
t1343 = t282+t655+t802+t1041;
t1363 = t44.*t108.*t1258.*4.306286555174926e-24;
t1366 = t44.*t108.*t1259.*7.660522649005482e-24;
t1429 = t1205.*t1210.*1.02e-6;
t1453 = t1210.*(t992+t12.*(t635-t996)).*(-1.02e-6);
t1455 = t1210.*(t992+t12.*(t635-t996)).*1.02e-6;
t1456 = t1210.*(t992+t12.*(t635-t996)).*(-9.0e-8);
t1457 = t1240.*t1259;
t1458 = t1210.*(t992+t12.*(t635-t996)).*9.0e-8;
t1464 = t1243.*t1259.*3.24e-6;
t1465 = t1243.*t1259.*3.11e-6;
t1472 = t1075+t1082+t1189+t1192;
t1473 = t1079+t1080+t1188+t1191;
t1477 = t1094+t1105+t1199+t1204;
t1478 = t1103+t1104+t1198+t1201;
t1534 = t1136+t1152+t1229+t1230;
t1535 = t1144+t1146+t1228+t1231;
t1560 = t1243.*(t1097-t1103+t1196-t1201).*(-1.1e-7);
t1561 = t1243.*(t1097-t1103+t1196-t1201).*(-3.24e-6);
t1563 = t1243.*(t1097-t1103+t1196-t1201).*1.1e-7;
t1564 = t1243.*(t1097-t1103+t1196-t1201).*(-3.11e-6);
t1566 = t1243.*(t1097-t1103+t1196-t1201).*3.24e-6;
t1568 = t1243.*(t1097-t1103+t1196-t1201).*3.11e-6;
t1569 = t1242.*(t1097-t1103+t1196-t1201).*(-5.0e-8);
t1570 = t1243.*(t1097-t1103+t1196-t1201).*(-5.0e-8);
t1571 = t1242.*(t1097-t1103+t1196-t1201).*(-1.6e-7);
t1573 = t1243.*(t1097-t1103+t1196-t1201).*5.0e-8;
t1584 = t1241+t1335+t1344;
t1589 = t650+t794+t1015+t1123+t1128+t1224+t1225;
t1655 = t270+t795+t806+t827+t1123+t1128+t1130+t1139+t1224+t1225;
t1251 = t10.*t1245;
t1252 = t11.*t1244;
t1253 = t15.*t1245;
t1254 = t16.*t1244;
t1255 = t1248.*(3.0./5.0e+2);
t1266 = t20.*t1261;
t1267 = t21.*t1260;
t1268 = t26.*t1261;
t1269 = t27.*t1260;
t1270 = -t1265;
t1271 = t1263.*(3.0./5.0e+2);
t1281 = t1250.*1.247162e-2;
t1282 = t1247.*5.84482e-3;
t1285 = t1248.*5.68686e-3;
t1286 = t1247.*6.48e-5;
t1293 = t1248.*3.131399999999998e-4;
t1294 = t1249.*6.47e-6;
t1299 = t1265.*1.247162e-2;
t1300 = t1262.*5.84482e-3;
t1303 = t1262.*6.48e-5;
t1308 = t1263.*3.131399999999998e-4;
t1309 = t1264.*6.47e-6;
t1310 = t1263.*4.36041e-5;
t1320 = t1265.*1.35652563578e-4;
t1321 = t1262.*1.688944904408e-4;
t1322 = t1263.*6.1855407534e-5;
t1327 = t1262.*7.0482312e-7;
t1329 = t1264.*1.869599668e-7;
t1345 = t777+t1249;
t1346 = t780+t1247;
t1351 = -t12.*(t778-t1247);
t1352 = -t17.*(t778-t1247);
t1365 = t44.*t108.*t1261.*4.306286555174926e-24;
t1367 = t44.*t108.*t1260.*7.660522649005482e-24;
t1369 = t797+t1264;
t1370 = t807+t1262;
t1375 = -t22.*(t799-t1262);
t1376 = -t28.*(t799-t1262);
t1380 = t22.*(t799-t1262);
t1390 = t12.*(t778-t1247).*(-9.99471e-3);
t1391 = t17.*(t778-t1247).*(-1.838876e-2);
t1393 = t12.*(t778-t1247).*9.99471e-3;
t1395 = t17.*(t778-t1247).*1.838876e-2;
t1407 = t28.*(t799-t1262).*(-1.838876e-2);
t1411 = t28.*(t799-t1262).*1.838876e-2;
t1421 = t44.*t116.*t1315.*8.875020496606951e-23;
t1424 = t44.*t116.*t1315.*8.588729512845436e-24;
t1433 = t28.*(t799-t1262).*(-1.33637554986e-4);
t1442 = t1210.*t1237;
t1443 = t997.*t1315.*9.3e-7;
t1444 = t997.*t1315.*9.0e-8;
t1447 = t997.*t1343;
t1448 = t824+t852+t1149+t1154;
t1449 = t1210.*t1315.*9.3e-7;
t1451 = t1210.*t1315.*9.0e-8;
t1460 = t1240.*t1260;
t1466 = t1244.*t1260.*3.24e-6;
t1467 = t1244.*t1260.*3.11e-6;
t1468 = t179+t654+t829+t851+t1150+t1157;
t1474 = -t1239.*(t799-t1262);
t1476 = t1239.*(t799-t1262);
t1489 = t1259.*(t778-t1247).*(-1.0e-8);
t1509 = t1259.*(t778-t1247).*(-6.2e-7);
t1512 = t1259.*(t778-t1247).*(-3.24e-6);
t1513 = t1259.*(t778-t1247).*(-7.83e-6);
t1516 = t1259.*(t778-t1247).*3.24e-6;
t1517 = t1259.*(t778-t1247).*7.83e-6;
t1536 = t270+t786+t791+t795+t806+t1130+t1135;
t1539 = t288+t790+t811+t814+t828+t1151+t1156;
t1540 = -t1343.*(t799-t1262);
t1544 = t44.*t108.*t1477.*(t36-t37).*(-2.711709361697228e-39);
t1545 = t44.*t108.*t1477.*(t36-t37).*2.711709361697228e-39;
t1547 = ((t778-t1247).*(t799-t1262))./1.0e+8;
t1549 = (t778-t1247).*(t799-t1262).*6.2e-7;
t1557 = t1175+t1363+t1366;
t1562 = t1244.*t1477.*1.1e-7;
t1565 = t1244.*t1477.*3.24e-6;
t1567 = t1244.*t1477.*3.11e-6;
t1572 = t1244.*t1477.*5.0e-8;
t1574 = t1245.*t1477.*5.0e-8;
t1575 = t1245.*t1477.*1.6e-7;
t1590 = t653+t801+t1025+t1140+t1147+t1232+t1233;
t1591 = ((t778-t1247).*(t1097-t1103+t1196-t1201))./1.0e+8;
t1594 = -t1318.*(-t1136+t1148+t12.*(t635-t996).*9.0e-8+t17.*(t635-t996).*9.3e-7);
t1595 = -t1319.*(t1137-t1146+t12.*(t635-t996).*1.02e-6+t17.*(t635-t996).*9.0e-8);
t1597 = (t778-t1247).*(t1097-t1103+t1196-t1201).*6.2e-7;
t1598 = (t778-t1247).*(t1097-t1103+t1196-t1201).*3.24e-6;
t1599 = (t778-t1247).*(t1097-t1103+t1196-t1201).*7.83e-6;
t1603 = t1319.*(t1137-t1146+t12.*(t635-t996).*1.02e-6+t17.*(t635-t996).*9.0e-8);
t1608 = t44.*t108.*t1584.*9.543032792050485e-17;
t1639 = t260+t279+t646+t783+t793+t826+t1020+t1124+t1127+t1226+t1227;
t1659 = t267+t305+t652+t787+t812+t840+t1039+t1141+t1145+t1234+t1235;
t1662 = t288+t814+t828+t843+t1140+t1147+t1151+t1158+t1232+t1233;
t1700 = -t1655.*(t778-t1247);
t1256 = t1252.*(3.0./5.0e+2);
t1257 = -t1255;
t1272 = t1267.*(3.0./5.0e+2);
t1273 = -t1271;
t1283 = t1254.*1.247162e-2;
t1284 = -t1281;
t1287 = -t1282;
t1288 = t1251.*5.84482e-3;
t1289 = t1252.*5.68686e-3;
t1290 = -t1286;
t1291 = t1251.*6.48e-5;
t1295 = t1252.*3.131399999999998e-4;
t1296 = t1253.*6.47e-6;
t1301 = t1269.*1.247162e-2;
t1302 = -t1299;
t1304 = -t1300;
t1305 = t1266.*5.84482e-3;
t1306 = t1266.*6.48e-5;
t1311 = t1267.*3.131399999999998e-4;
t1312 = t1268.*6.47e-6;
t1313 = t1267.*4.36041e-5;
t1323 = t1269.*1.35652563578e-4;
t1324 = -t1321;
t1325 = t1266.*1.688944904408e-4;
t1326 = t1267.*6.1855407534e-5;
t1330 = -t1327;
t1331 = t1266.*7.0482312e-7;
t1332 = t1268.*1.869599668e-7;
t1347 = t781+t1251;
t1348 = t782+t1253;
t1349 = t11.*t1345;
t1350 = t16.*t1345;
t1368 = -t1367;
t1371 = t808+t1266;
t1372 = t816+t1268;
t1373 = t21.*t1369;
t1374 = t27.*t1369;
t1406 = t1380.*(-9.99471e-3);
t1409 = t1380.*9.99471e-3;
t1422 = -t1421;
t1426 = -t1424;
t1434 = t1380.*(-7.26350557185e-5);
t1436 = t1380.*7.26350557185e-5;
t1450 = -t1449;
t1452 = t1177.*t1369;
t1454 = -t1451;
t1494 = -t1448.*(t642-t1014);
t1498 = t1448.*(t642-t1014);
t1506 = t1259.*t1345.*9.840000000000001e-6;
t1553 = t1210.*t1468;
t1593 = t1345.*(t1097-t1103+t1196-t1201).*(-9.840000000000001e-6);
t1686 = t1543+t1545;
t1688 = -t1557.*(t1077-t1079+t1186-t1191);
t1689 = t1557.*(t1077-t1079+t1186-t1191);
t1690 = -t1472.*(-t1365+t1367+t44.*t107.*t116.*(t40-t41).*2.711709361697228e-39);
t1691 = t1472.*(-t1365+t1367+t44.*t107.*t116.*(t40-t41).*2.711709361697228e-39);
t1694 = t1243.*t1639;
t1695 = t1244.*t1639;
t1696 = t1259.*t1659.*7.26735e-3;
t1697 = t1260.*t1659.*7.26735e-3;
t1723 = t1662.*(t799-t1262).*(-7.26735e-3);
t1760 = t1442+t1594+t1603;
t1803 = t1562+t1563+t1569+t1574;
t1804 = t1571+t1572+t1573+t1575;
t1292 = -t1288;
t1297 = -t1295;
H = ft_3({t10,t1001,t1002,t1003,t1004,t1005,t1012,t1014,t1018,t1019,t1020,t1021,t1022,t1026,t1027,t1028,t1033,t1034,t1035,t1039,t1043,t1044,t1045,t1048,t1049,t1051,t1052,t1063,t1064,t107,t1073,t1074,t1076,t1077,t1078,t1079,t108,t1081,t1083,t1084,t1085,t1086,t1087,t1088,t1089,t1090,t1092,t1093,t1095,t1096,t1097,t1098,t1099,t11,t1100,t1101,t1102,t1103,t1106,t1107,t1108,t1109,t1110,t1112,t1113,t1114,t1116,t1117,t1118,t1119,t1120,t1121,t1122,t1124,t1125,t1126,t1127,t1129,t1131,t1132,t1134,t1136,t1137,t1138,t1141,t1145,t1146,t1148,t115,t116,t1161,t1162,t1163,t1164,t1166,t1167,t1169,t1170,t1171,t1172,t1173,t1176,t1177,t1186,t1191,t1193,t1194,t1195,t1196,t12,t1201,t1202,t1203,t1205,t1207,t1210,t1215,t1216,t1217,t1220,t1221,t1222,t1223,t1226,t1227,t1234,t1235,t1236,t1237,t1238,t1239,t1243,t1244,t1246,t1247,t1248,t1250,t1252,t1254,t1255,t1256,t1257,t1258,t1259,t1260,t1261,t1262,t1263,t1265,t1267,t1269,t1270,t1272,t1273,t1274,t1275,t1277,t1278,t1280,t1281,t1283,t1284,t1285,t1286,t1287,t1288,t1289,t1290,t1291,t1292,t1293,t1294,t1296,t1297,t1299,t130,t1301,t1302,t1303,t1304,t1305,t1306,t1308,t1309,t131,t1310,t1311,t1312,t1313,t1317,t1318,t1319,t132,t1320,t1322,t1323,t1324,t1325,t1326,t1329,t1330,t1331,t1332,t1336,t1337,t1338,t1339,t134,t1340,t1342,t1343,t1347,t1348,t1349,t1350,t1351,t1352,t1365,t1368,t1369,t1371,t1372,t1373,t1374,t1376,t1380,t1390,t1391,t1393,t1395,t1404,t1406,t1407,t1408,t1409,t1411,t1422,t1425,t1426,t1428,t1429,t143,t1433,t1436,t1443,t1444,t1445,t1446,t1447,t1448,t145,t1450,t1452,t1454,t1455,t1457,t1458,t1460,t1462,t1463,t1464,t1465,t1466,t1467,t1468,t1469,t1470,t1471,t1472,t1476,t1477,t1488,t1489,t1498,t15,t1506,t1509,t1516,t1517,t1530,t1536,t1539,t1540,t1546,t1547,t1549,t1551,t1553,t1554,t1565,t1566,t1567,t1568,t1584,t1591,t1593,t1597,t1598,t1599,t16,t1608,t1633,t1634,t1638,t164,t165,t1655,t1660,t1662,t168,t1685,t1686,t1689,t169,t1691,t1692,t1694,t1695,t1696,t1697,t17,t170,t1700,t172,t1723,t173,t174,t175,t176,t1760,t177,t18,t180,t1803,t1804,t181,t1822,t183,t185,t1858,t188,t189,t190,t191,t192,t194,t196,t197,t198,t199,t20,t200,t201,t202,t203,t205,t206,t207,t208,t21,t212,t214,t216,t218,t22,t24,t26,t27,t28,t313,t317,t318,t319,t32,t320,t321,t322,t323,t324,t325,t326,t328,t33,t331,t332,t333,t334,t335,t336,t338,t339,t340,t341,t342,t343,t344,t345,t347,t348,t349,t350,t351,t352,t353,t354,t355,t356,t357,t358,t359,t36,t360,t361,t363,t365,t366,t367,t368,t37,t373,t375,t376,t377,t380,t381,t382,t383,t384,t385,t386,t387,t390,t391,t392,t393,t397,t40,t400,t402,t403,t406,t41,t411,t412,t416,t417,t419,t420,t423,t425,t44,t47,t48,t49,t493,t497,t498,t499,t50,t504,t505,t51,t517,t518,t52,t529,t532,t533,t534,t538,t540,t541,t542,t543,t545,t548,t549,t55,t550,t551,t552,t553,t556,t558,t559,t56,t560,t561,t576,t577,t58,t582,t583,t587,t588,t59,t591,t597,t598,t599,t60,t603,t606,t61,t610,t616,t625,t628,t635,t64,t642,t646,t652,t656,t669,t670,t671,t672,t673,t675,t676,t677,t678,t679,t68,t680,t681,t683,t684,t685,t686,t687,t688,t689,t69,t690,t691,t692,t693,t694,t695,t696,t697,t70,t702,t703,t704,t705,t706,t709,t71,t711,t712,t715,t716,t719,t72,t720,t721,t722,t723,t727,t728,t73,t731,t732,t735,t736,t738,t741,t743,t75,t751,t752,t753,t757,t758,t759,t760,t763,t764,t767,t768,t778,t786,t790,t799,t8,t832,t835,t837,t838,t844,t845,t847,t850,t861,t864,t87,t870,t875,t876,t880,t881,t892,t895,t897,t898,t9,t909,t910,t911,t912,t913,t914,t915,t916,t917,t918,t919,t920,t921,t922,t923,t924,t926,t927,t928,t929,t930,t931,t932,t937,t940,t941,t944,t945,t946,t948,t949,t956,t957,t958,t959,t962,t963,t968,t969,t981,t982,t983,t984,t985,t986,t987,t989,t990,t993,t994,t996,t997,t998});
end
function H = ft_3(ct)
t10 = ct{1};
t1001 = ct{2};
t1002 = ct{3};
t1003 = ct{4};
t1004 = ct{5};
t1005 = ct{6};
t1012 = ct{7};
t1014 = ct{8};
t1018 = ct{9};
t1019 = ct{10};
t1020 = ct{11};
t1021 = ct{12};
t1022 = ct{13};
t1026 = ct{14};
t1027 = ct{15};
t1028 = ct{16};
t1033 = ct{17};
t1034 = ct{18};
t1035 = ct{19};
t1039 = ct{20};
t1043 = ct{21};
t1044 = ct{22};
t1045 = ct{23};
t1048 = ct{24};
t1049 = ct{25};
t1051 = ct{26};
t1052 = ct{27};
t1063 = ct{28};
t1064 = ct{29};
t107 = ct{30};
t1073 = ct{31};
t1074 = ct{32};
t1076 = ct{33};
t1077 = ct{34};
t1078 = ct{35};
t1079 = ct{36};
t108 = ct{37};
t1081 = ct{38};
t1083 = ct{39};
t1084 = ct{40};
t1085 = ct{41};
t1086 = ct{42};
t1087 = ct{43};
t1088 = ct{44};
t1089 = ct{45};
t1090 = ct{46};
t1092 = ct{47};
t1093 = ct{48};
t1095 = ct{49};
t1096 = ct{50};
t1097 = ct{51};
t1098 = ct{52};
t1099 = ct{53};
t11 = ct{54};
t1100 = ct{55};
t1101 = ct{56};
t1102 = ct{57};
t1103 = ct{58};
t1106 = ct{59};
t1107 = ct{60};
t1108 = ct{61};
t1109 = ct{62};
t1110 = ct{63};
t1112 = ct{64};
t1113 = ct{65};
t1114 = ct{66};
t1116 = ct{67};
t1117 = ct{68};
t1118 = ct{69};
t1119 = ct{70};
t1120 = ct{71};
t1121 = ct{72};
t1122 = ct{73};
t1124 = ct{74};
t1125 = ct{75};
t1126 = ct{76};
t1127 = ct{77};
t1129 = ct{78};
t1131 = ct{79};
t1132 = ct{80};
t1134 = ct{81};
t1136 = ct{82};
t1137 = ct{83};
t1138 = ct{84};
t1141 = ct{85};
t1145 = ct{86};
t1146 = ct{87};
t1148 = ct{88};
t115 = ct{89};
t116 = ct{90};
t1161 = ct{91};
t1162 = ct{92};
t1163 = ct{93};
t1164 = ct{94};
t1166 = ct{95};
t1167 = ct{96};
t1169 = ct{97};
t1170 = ct{98};
t1171 = ct{99};
t1172 = ct{100};
t1173 = ct{101};
t1176 = ct{102};
t1177 = ct{103};
t1186 = ct{104};
t1191 = ct{105};
t1193 = ct{106};
t1194 = ct{107};
t1195 = ct{108};
t1196 = ct{109};
t12 = ct{110};
t1201 = ct{111};
t1202 = ct{112};
t1203 = ct{113};
t1205 = ct{114};
t1207 = ct{115};
t1210 = ct{116};
t1215 = ct{117};
t1216 = ct{118};
t1217 = ct{119};
t1220 = ct{120};
t1221 = ct{121};
t1222 = ct{122};
t1223 = ct{123};
t1226 = ct{124};
t1227 = ct{125};
t1234 = ct{126};
t1235 = ct{127};
t1236 = ct{128};
t1237 = ct{129};
t1238 = ct{130};
t1239 = ct{131};
t1243 = ct{132};
t1244 = ct{133};
t1246 = ct{134};
t1247 = ct{135};
t1248 = ct{136};
t1250 = ct{137};
t1252 = ct{138};
t1254 = ct{139};
t1255 = ct{140};
t1256 = ct{141};
t1257 = ct{142};
t1258 = ct{143};
t1259 = ct{144};
t1260 = ct{145};
t1261 = ct{146};
t1262 = ct{147};
t1263 = ct{148};
t1265 = ct{149};
t1267 = ct{150};
t1269 = ct{151};
t1270 = ct{152};
t1272 = ct{153};
t1273 = ct{154};
t1274 = ct{155};
t1275 = ct{156};
t1277 = ct{157};
t1278 = ct{158};
t1280 = ct{159};
t1281 = ct{160};
t1283 = ct{161};
t1284 = ct{162};
t1285 = ct{163};
t1286 = ct{164};
t1287 = ct{165};
t1288 = ct{166};
t1289 = ct{167};
t1290 = ct{168};
t1291 = ct{169};
t1292 = ct{170};
t1293 = ct{171};
t1294 = ct{172};
t1296 = ct{173};
t1297 = ct{174};
t1299 = ct{175};
t130 = ct{176};
t1301 = ct{177};
t1302 = ct{178};
t1303 = ct{179};
t1304 = ct{180};
t1305 = ct{181};
t1306 = ct{182};
t1308 = ct{183};
t1309 = ct{184};
t131 = ct{185};
t1310 = ct{186};
t1311 = ct{187};
t1312 = ct{188};
t1313 = ct{189};
t1317 = ct{190};
t1318 = ct{191};
t1319 = ct{192};
t132 = ct{193};
t1320 = ct{194};
t1322 = ct{195};
t1323 = ct{196};
t1324 = ct{197};
t1325 = ct{198};
t1326 = ct{199};
t1329 = ct{200};
t1330 = ct{201};
t1331 = ct{202};
t1332 = ct{203};
t1336 = ct{204};
t1337 = ct{205};
t1338 = ct{206};
t1339 = ct{207};
t134 = ct{208};
t1340 = ct{209};
t1342 = ct{210};
t1343 = ct{211};
t1347 = ct{212};
t1348 = ct{213};
t1349 = ct{214};
t1350 = ct{215};
t1351 = ct{216};
t1352 = ct{217};
t1365 = ct{218};
t1368 = ct{219};
t1369 = ct{220};
t1371 = ct{221};
t1372 = ct{222};
t1373 = ct{223};
t1374 = ct{224};
t1376 = ct{225};
t1380 = ct{226};
t1390 = ct{227};
t1391 = ct{228};
t1393 = ct{229};
t1395 = ct{230};
t1404 = ct{231};
t1406 = ct{232};
t1407 = ct{233};
t1408 = ct{234};
t1409 = ct{235};
t1411 = ct{236};
t1422 = ct{237};
t1425 = ct{238};
t1426 = ct{239};
t1428 = ct{240};
t1429 = ct{241};
t143 = ct{242};
t1433 = ct{243};
t1436 = ct{244};
t1443 = ct{245};
t1444 = ct{246};
t1445 = ct{247};
t1446 = ct{248};
t1447 = ct{249};
t1448 = ct{250};
t145 = ct{251};
t1450 = ct{252};
t1452 = ct{253};
t1454 = ct{254};
t1455 = ct{255};
t1457 = ct{256};
t1458 = ct{257};
t1460 = ct{258};
t1462 = ct{259};
t1463 = ct{260};
t1464 = ct{261};
t1465 = ct{262};
t1466 = ct{263};
t1467 = ct{264};
t1468 = ct{265};
t1469 = ct{266};
t1470 = ct{267};
t1471 = ct{268};
t1472 = ct{269};
t1476 = ct{270};
t1477 = ct{271};
t1488 = ct{272};
t1489 = ct{273};
t1498 = ct{274};
t15 = ct{275};
t1506 = ct{276};
t1509 = ct{277};
t1516 = ct{278};
t1517 = ct{279};
t1530 = ct{280};
t1536 = ct{281};
t1539 = ct{282};
t1540 = ct{283};
t1546 = ct{284};
t1547 = ct{285};
t1549 = ct{286};
t1551 = ct{287};
t1553 = ct{288};
t1554 = ct{289};
t1565 = ct{290};
t1566 = ct{291};
t1567 = ct{292};
t1568 = ct{293};
t1584 = ct{294};
t1591 = ct{295};
t1593 = ct{296};
t1597 = ct{297};
t1598 = ct{298};
t1599 = ct{299};
t16 = ct{300};
t1608 = ct{301};
t1633 = ct{302};
t1634 = ct{303};
t1638 = ct{304};
t164 = ct{305};
t165 = ct{306};
t1655 = ct{307};
t1660 = ct{308};
t1662 = ct{309};
t168 = ct{310};
t1685 = ct{311};
t1686 = ct{312};
t1689 = ct{313};
t169 = ct{314};
t1691 = ct{315};
t1692 = ct{316};
t1694 = ct{317};
t1695 = ct{318};
t1696 = ct{319};
t1697 = ct{320};
t17 = ct{321};
t170 = ct{322};
t1700 = ct{323};
t172 = ct{324};
t1723 = ct{325};
t173 = ct{326};
t174 = ct{327};
t175 = ct{328};
t176 = ct{329};
t1760 = ct{330};
t177 = ct{331};
t18 = ct{332};
t180 = ct{333};
t1803 = ct{334};
t1804 = ct{335};
t181 = ct{336};
t1822 = ct{337};
t183 = ct{338};
t185 = ct{339};
t1858 = ct{340};
t188 = ct{341};
t189 = ct{342};
t190 = ct{343};
t191 = ct{344};
t192 = ct{345};
t194 = ct{346};
t196 = ct{347};
t197 = ct{348};
t198 = ct{349};
t199 = ct{350};
t20 = ct{351};
t200 = ct{352};
t201 = ct{353};
t202 = ct{354};
t203 = ct{355};
t205 = ct{356};
t206 = ct{357};
t207 = ct{358};
t208 = ct{359};
t21 = ct{360};
t212 = ct{361};
t214 = ct{362};
t216 = ct{363};
t218 = ct{364};
t22 = ct{365};
t24 = ct{366};
t26 = ct{367};
t27 = ct{368};
t28 = ct{369};
t313 = ct{370};
t317 = ct{371};
t318 = ct{372};
t319 = ct{373};
t32 = ct{374};
t320 = ct{375};
t321 = ct{376};
t322 = ct{377};
t323 = ct{378};
t324 = ct{379};
t325 = ct{380};
t326 = ct{381};
t328 = ct{382};
t33 = ct{383};
t331 = ct{384};
t332 = ct{385};
t333 = ct{386};
t334 = ct{387};
t335 = ct{388};
t336 = ct{389};
t338 = ct{390};
t339 = ct{391};
t340 = ct{392};
t341 = ct{393};
t342 = ct{394};
t343 = ct{395};
t344 = ct{396};
t345 = ct{397};
t347 = ct{398};
t348 = ct{399};
t349 = ct{400};
t350 = ct{401};
t351 = ct{402};
t352 = ct{403};
t353 = ct{404};
t354 = ct{405};
t355 = ct{406};
t356 = ct{407};
t357 = ct{408};
t358 = ct{409};
t359 = ct{410};
t36 = ct{411};
t360 = ct{412};
t361 = ct{413};
t363 = ct{414};
t365 = ct{415};
t366 = ct{416};
t367 = ct{417};
t368 = ct{418};
t37 = ct{419};
t373 = ct{420};
t375 = ct{421};
t376 = ct{422};
t377 = ct{423};
t380 = ct{424};
t381 = ct{425};
t382 = ct{426};
t383 = ct{427};
t384 = ct{428};
t385 = ct{429};
t386 = ct{430};
t387 = ct{431};
t390 = ct{432};
t391 = ct{433};
t392 = ct{434};
t393 = ct{435};
t397 = ct{436};
t40 = ct{437};
t400 = ct{438};
t402 = ct{439};
t403 = ct{440};
t406 = ct{441};
t41 = ct{442};
t411 = ct{443};
t412 = ct{444};
t416 = ct{445};
t417 = ct{446};
t419 = ct{447};
t420 = ct{448};
t423 = ct{449};
t425 = ct{450};
t44 = ct{451};
t47 = ct{452};
t48 = ct{453};
t49 = ct{454};
t493 = ct{455};
t497 = ct{456};
t498 = ct{457};
t499 = ct{458};
t50 = ct{459};
t504 = ct{460};
t505 = ct{461};
t51 = ct{462};
t517 = ct{463};
t518 = ct{464};
t52 = ct{465};
t529 = ct{466};
t532 = ct{467};
t533 = ct{468};
t534 = ct{469};
t538 = ct{470};
t540 = ct{471};
t541 = ct{472};
t542 = ct{473};
t543 = ct{474};
t545 = ct{475};
t548 = ct{476};
t549 = ct{477};
t55 = ct{478};
t550 = ct{479};
t551 = ct{480};
t552 = ct{481};
t553 = ct{482};
t556 = ct{483};
t558 = ct{484};
t559 = ct{485};
t56 = ct{486};
t560 = ct{487};
t561 = ct{488};
t576 = ct{489};
t577 = ct{490};
t58 = ct{491};
t582 = ct{492};
t583 = ct{493};
t587 = ct{494};
t588 = ct{495};
t59 = ct{496};
t591 = ct{497};
t597 = ct{498};
t598 = ct{499};
t599 = ct{500};
t60 = ct{501};
t603 = ct{502};
t606 = ct{503};
t61 = ct{504};
t610 = ct{505};
t616 = ct{506};
t625 = ct{507};
t628 = ct{508};
t635 = ct{509};
t64 = ct{510};
t642 = ct{511};
t646 = ct{512};
t652 = ct{513};
t656 = ct{514};
t669 = ct{515};
t670 = ct{516};
t671 = ct{517};
t672 = ct{518};
t673 = ct{519};
t675 = ct{520};
t676 = ct{521};
t677 = ct{522};
t678 = ct{523};
t679 = ct{524};
t68 = ct{525};
t680 = ct{526};
t681 = ct{527};
t683 = ct{528};
t684 = ct{529};
t685 = ct{530};
t686 = ct{531};
t687 = ct{532};
t688 = ct{533};
t689 = ct{534};
t69 = ct{535};
t690 = ct{536};
t691 = ct{537};
t692 = ct{538};
t693 = ct{539};
t694 = ct{540};
t695 = ct{541};
t696 = ct{542};
t697 = ct{543};
t70 = ct{544};
t702 = ct{545};
t703 = ct{546};
t704 = ct{547};
t705 = ct{548};
t706 = ct{549};
t709 = ct{550};
t71 = ct{551};
t711 = ct{552};
t712 = ct{553};
t715 = ct{554};
t716 = ct{555};
t719 = ct{556};
t72 = ct{557};
t720 = ct{558};
t721 = ct{559};
t722 = ct{560};
t723 = ct{561};
t727 = ct{562};
t728 = ct{563};
t73 = ct{564};
t731 = ct{565};
t732 = ct{566};
t735 = ct{567};
t736 = ct{568};
t738 = ct{569};
t741 = ct{570};
t743 = ct{571};
t75 = ct{572};
t751 = ct{573};
t752 = ct{574};
t753 = ct{575};
t757 = ct{576};
t758 = ct{577};
t759 = ct{578};
t760 = ct{579};
t763 = ct{580};
t764 = ct{581};
t767 = ct{582};
t768 = ct{583};
t778 = ct{584};
t786 = ct{585};
t790 = ct{586};
t799 = ct{587};
t8 = ct{588};
t832 = ct{589};
t835 = ct{590};
t837 = ct{591};
t838 = ct{592};
t844 = ct{593};
t845 = ct{594};
t847 = ct{595};
t850 = ct{596};
t861 = ct{597};
t864 = ct{598};
t87 = ct{599};
t870 = ct{600};
t875 = ct{601};
t876 = ct{602};
t880 = ct{603};
t881 = ct{604};
t892 = ct{605};
t895 = ct{606};
t897 = ct{607};
t898 = ct{608};
t9 = ct{609};
t909 = ct{610};
t910 = ct{611};
t911 = ct{612};
t912 = ct{613};
t913 = ct{614};
t914 = ct{615};
t915 = ct{616};
t916 = ct{617};
t917 = ct{618};
t918 = ct{619};
t919 = ct{620};
t920 = ct{621};
t921 = ct{622};
t922 = ct{623};
t923 = ct{624};
t924 = ct{625};
t926 = ct{626};
t927 = ct{627};
t928 = ct{628};
t929 = ct{629};
t930 = ct{630};
t931 = ct{631};
t932 = ct{632};
t937 = ct{633};
t940 = ct{634};
t941 = ct{635};
t944 = ct{636};
t945 = ct{637};
t946 = ct{638};
t948 = ct{639};
t949 = ct{640};
t956 = ct{641};
t957 = ct{642};
t958 = ct{643};
t959 = ct{644};
t962 = ct{645};
t963 = ct{646};
t968 = ct{647};
t969 = ct{648};
t981 = ct{649};
t982 = ct{650};
t983 = ct{651};
t984 = ct{652};
t985 = ct{653};
t986 = ct{654};
t987 = ct{655};
t989 = ct{656};
t990 = ct{657};
t993 = ct{658};
t994 = ct{659};
t996 = ct{660};
t997 = ct{661};
t998 = ct{662};
t1298 = -t1296;
t1307 = -t1305;
t1314 = -t1311;
t1328 = -t1325;
t1333 = -t1332;
t1353 = t12.*t1347;
t1354 = -t1349;
t1355 = t17.*t1347;
t1356 = t11.*t1348;
t1357 = t16.*t1348;
t1360 = t1350.*(3.0./5.0e+2);
t1377 = t22.*t1371;
t1378 = t28.*t1371;
t1379 = t21.*t1372;
t1381 = t27.*t1372;
t1384 = t1374.*(3.0./5.0e+2);
t1388 = t1349.*1.247162e-2;
t1389 = t1350.*5.68686e-3;
t1397 = t1350.*3.131399999999998e-4;
t1405 = t1373.*1.247162e-2;
t1413 = t1374.*3.131399999999998e-4;
t1417 = t1374.*4.36041e-5;
t1430 = t1373.*1.35652563578e-4;
t1431 = t1374.*6.1855407534e-5;
t1459 = t1177.*t1372;
t1475 = t1239.*t1371;
t1479 = t1248+t1350;
t1490 = (t1260.*t1347)./1.0e+8;
t1492 = t1263+t1374;
t1493 = t1270+t1373;
t1507 = -t1506;
t1508 = t1260.*t1348.*9.840000000000001e-6;
t1518 = t1260.*t1347.*6.2e-7;
t1519 = t1260.*t1347.*3.24e-6;
t1520 = t1260.*t1347.*7.83e-6;
t1541 = t1343.*t1371;
t1548 = (t1347.*t1371)./1.0e+8;
t1550 = t1347.*t1371.*6.2e-7;
t1555 = -t1237.*(t1265-t1373);
t1559 = t1176+t1365+t1368;
t1592 = (t1347.*t1477)./1.0e+8;
t1596 = t1348.*t1477.*9.840000000000001e-6;
t1600 = t1347.*t1477.*6.2e-7;
t1601 = t1347.*t1477.*3.24e-6;
t1602 = t1347.*t1477.*7.83e-6;
t1635 = -t1468.*(t1265-t1373);
t1637 = t1468.*(t1265-t1373);
t1687 = t115.*t1686;
t1702 = t1347.*t1655;
t1711 = t1452+t1457+t1476;
t1724 = t1371.*t1662.*7.26735e-3;
t1725 = t50+t51+t325+t326+t341+t357+t669+t672+t675+t676+t981+t989+t1085+t1193+t1287+t1294;
t1726 = t60+t68+t325+t326+t341+t357+t669+t672+t675+t676+t981+t989+t1085+t1193+t1287+t1294;
t1733 = t1447+t1498+t1553;
t1743 = t169+t174+t532+t533+t553+t559+t909+t912+t923+t924+t1122+t1132+t1164+t1217+t1324+t1329;
t1744 = t191+t205+t532+t533+t553+t559+t909+t912+t923+t924+t1122+t1132+t1164+t1217+t1324+t1329;
t1761 = t44.*t108.*t1760.*9.543032792050485e-17;
t1762 = t984.*t1760;
t1765 = t1205.*t1760;
t1816 = t44.*t116.*t1803.*9.543032792050485e-17;
t1817 = t44.*t116.*t1804.*5.673626844500105e-17;
t1358 = -t1355;
t1359 = -t1357;
t1361 = -t1360;
t1362 = t1357.*(3.0./5.0e+2);
t1382 = -t1378;
t1383 = -t1381;
t1385 = -t1384;
t1386 = t1381.*(3.0./5.0e+2);
t1392 = -t1388;
t1394 = t1353.*9.99471e-3;
t1396 = t1355.*1.838876e-2;
t1400 = t1356.*1.247162e-2;
t1401 = t1357.*5.68686e-3;
t1403 = t1357.*3.131399999999998e-4;
t1410 = t1377.*9.99471e-3;
t1412 = t1378.*1.838876e-2;
t1416 = t1379.*1.247162e-2;
t1418 = t1381.*3.131399999999998e-4;
t1419 = t1381.*4.36041e-5;
t1432 = -t1430;
t1435 = t1378.*1.33637554986e-4;
t1437 = t1377.*7.26350557185e-5;
t1438 = t1379.*1.35652563578e-4;
t1440 = t1381.*6.1855407534e-5;
t1461 = -t1459;
t1480 = t1250+t1354;
t1481 = t12.*t1479;
t1482 = t17.*t1479;
t1483 = t1254+t1356;
t1491 = -t1490;
t1495 = t22.*t1492;
t1496 = t28.*t1492;
t1497 = t1269+t1379;
t1521 = -t1518;
t1542 = -t1541;
t1578 = t1259.*t1479.*5.7e-7;
t1579 = t1259.*t1479.*4.0e-8;
t1614 = t1479.*(t799-t1262).*(-5.7e-7);
t1615 = t1479.*(t799-t1262).*(-4.0e-8);
t1631 = t1448.*t1492;
t1643 = t1479.*(t1097-t1103+t1196-t1201).*(-5.7e-7);
t1644 = t1479.*(t1097-t1103+t1196-t1201).*(-4.0e-8);
t1693 = t1215+t1507+t1508;
t1727 = t48+t61+t322+t338+t339+t353+t673+t683+t684+t686+t983+t990+t1084+t1195+t1288+t1298;
t1728 = t47+t69+t328+t345+t360+t361+t670+t671+t677+t685+t987+t993+t1092+t1194+t1292+t1296;
t1736 = t1243.*t1711;
t1740 = t44.*t108.*t1733.*9.543032792050485e-17;
t1741 = t984.*t1733;
t1742 = t1593+t1596;
t1745 = t168+t185+t529+t545+t550+t551+t913+t914+t920+t932+t1125+t1134+t1163+t1223+t1325+t1333;
t1746 = t183+t206+t534+t543+t560+t561+t910+t911+t926+t928+t1129+t1138+t1169+t1220+t1328+t1332;
t1749 = -t1711.*(t1077-t1079+t1186-t1191);
t1771 = t1019+t1222+t1464+t1466+t1517+t1520;
t1772 = t1021+t1221+t1465+t1467+t1516+t1519;
t1818 = -t1817;
t1820 = t1565+t1566+t1599+t1602;
t1821 = t1567+t1568+t1598+t1601;
t1364 = -t1362;
t1387 = -t1386;
t1398 = -t1394;
t1399 = -t1396;
t1402 = -t1401;
t1414 = -t1410;
t1415 = -t1412;
t1420 = -t1419;
t1439 = -t1435;
t1441 = -t1440;
t1484 = -t1482;
t1485 = t1252+t1359;
t1499 = t1267+t1383;
t1500 = t1482.*9.99471e-3;
t1501 = t1481.*1.838876e-2;
t1522 = t1496.*9.99471e-3;
t1523 = t1495.*1.838876e-2;
t1532 = t1495.*1.33637554986e-4;
t1533 = t1496.*7.26350557185e-5;
t1556 = t1237.*t1497;
t1576 = (t1259.*t1480)./1.0e+8;
t1577 = (t1260.*t1483)./1.0e+8;
t1580 = t1259.*t1480.*1.02e-6;
t1581 = t1259.*t1480.*2.4e-7;
t1582 = t1259.*t1480.*4.0e-8;
t1583 = t1260.*t1483.*1.02e-6;
t1585 = t1260.*t1483.*2.4e-7;
t1586 = t1260.*t1483.*4.0e-8;
t1604 = t1352+t1481;
t1609 = t1480.*(t799-t1262).*(-1.0e-8);
t1610 = (t1371.*t1483)./1.0e+8;
t1612 = t1376+t1495;
t1613 = t1380+t1496;
t1616 = t1480.*(t799-t1262).*(-1.02e-6);
t1617 = t1480.*(t799-t1262).*(-2.4e-7);
t1618 = t1480.*(t799-t1262).*(-4.0e-8);
t1620 = t1371.*t1483.*1.02e-6;
t1622 = t1371.*t1483.*2.4e-7;
t1623 = t1371.*t1483.*4.0e-8;
t1636 = t1468.*t1497;
t1640 = t1480.*(t1097-t1103+t1196-t1201).*(-1.0e-8);
t1641 = (t1477.*t1483)./1.0e+8;
t1645 = t1480.*(t1097-t1103+t1196-t1201).*(-1.02e-6);
t1646 = t1480.*(t1097-t1103+t1196-t1201).*1.02e-6;
t1647 = t1480.*(t1097-t1103+t1196-t1201).*(-2.4e-7);
t1648 = t1480.*(t1097-t1103+t1196-t1201).*(-4.0e-8);
t1649 = t1477.*t1483.*1.02e-6;
t1650 = t1477.*t1483.*2.4e-7;
t1651 = t1477.*t1483.*4.0e-8;
t1664 = t1259.*(t1482+t12.*(t778-t1247)).*(-9.3e-7);
t1665 = t1259.*(t1482+t12.*(t778-t1247)).*9.3e-7;
t1666 = t1259.*(t1482+t12.*(t778-t1247)).*(-9.0e-8);
t1667 = t1259.*(t1482+t12.*(t778-t1247)).*9.0e-8;
t1672 = t1480.*(t1265-t1373).*(-1.02e-6);
t1673 = t1480.*(t1265-t1373).*1.02e-6;
t1674 = t1483.*t1497.*1.02e-6;
t1678 = (t1482+t12.*(t778-t1247)).*(t799-t1262).*9.3e-7;
t1680 = (t1482+t12.*(t778-t1247)).*(t799-t1262).*9.0e-8;
t1698 = t1001.*t1693;
t1704 = (t1482+t12.*(t778-t1247)).*(t1097-t1103+t1196-t1201).*9.3e-7;
t1706 = (t1482+t12.*(t778-t1247)).*(t1097-t1103+t1196-t1201).*9.0e-8;
t1712 = t1460+t1461+t1475;
t1716 = (t1482+t12.*(t778-t1247)).*(t1265-t1373).*9.3e-7;
t1718 = (t1482+t12.*(t778-t1247)).*(t1265-t1373).*9.0e-8;
t1734 = t1369.*t1693;
t1735 = t1372.*t1693;
t1737 = -t1736;
t1747 = t1001.*t1742;
t1752 = t50+t51+t317+t318+t354+t363+t678+t690+t692+t693+t982+t1281+t1285+t1290+t1389+t1392;
t1753 = t60+t68+t317+t318+t354+t363+t678+t690+t692+t693+t982+t1281+t1285+t1290+t1389+t1392;
t1757 = t1369.*t1742;
t1758 = t1372.*t1742;
t1766 = t172+t180+t540+t541+t552+t558+t916+t917+t918+t931+t1126+t1320+t1322+t1330+t1431+t1432;
t1767 = t190+t200+t540+t541+t552+t558+t916+t917+t918+t931+t1126+t1320+t1322+t1330+t1431+t1432;
t1776 = t44.*t116.*t1772.*9.543032792050485e-17;
t1777 = t997.*t1771;
t1783 = t1259.*t1772;
t1784 = t1260.*t1772;
t1786 = t1540+t1631+t1637;
t1788 = -t1771.*(t799-t1262);
t1789 = t1371.*t1771;
t1824 = t44.*t116.*t1821.*9.543032792050485e-17;
t1825 = t997.*t1820;
t1830 = t1259.*t1821;
t1831 = t1260.*t1821;
t1834 = -t1820.*(t799-t1262);
t1835 = t1371.*t1820;
t1486 = t12.*t1485;
t1487 = t17.*t1485;
t1502 = t22.*t1499;
t1503 = t28.*t1499;
t1504 = -t1500;
t1505 = -t1501;
t1524 = -t1522;
t1525 = -t1523;
t1558 = -t1556;
t1587 = t1260.*t1485.*5.7e-7;
t1588 = t1260.*t1485.*4.0e-8;
t1605 = t1351+t1484;
t1611 = -t1610;
t1621 = -t1620;
t1625 = t1371.*t1485.*5.7e-7;
t1626 = -t1622;
t1627 = -t1623;
t1629 = t1371.*t1485.*4.0e-8;
t1632 = t1448.*t1499;
t1642 = -t1641;
t1652 = t1477.*t1485.*5.7e-7;
t1653 = -t1650;
t1654 = -t1651;
t1657 = t1477.*t1485.*4.0e-8;
t1661 = t1259.*t1604.*1.02e-6;
t1663 = t1259.*t1604.*9.0e-8;
t1675 = t1604.*(t799-t1262).*(-1.02e-6);
t1676 = t1604.*(t799-t1262).*1.02e-6;
t1677 = t1604.*(t799-t1262).*(-9.0e-8);
t1679 = t1604.*(t799-t1262).*9.0e-8;
t1699 = t1604.*(t1097-t1103+t1196-t1201).*(-1.02e-6);
t1701 = t1604.*(t1097-t1103+t1196-t1201).*1.02e-6;
t1703 = t1604.*(t1097-t1103+t1196-t1201).*(-9.0e-8);
t1705 = t1604.*(t1097-t1103+t1196-t1201).*9.0e-8;
t1713 = t1604.*(t1265-t1373).*(-1.02e-6);
t1714 = t1604.*(t1265-t1373).*1.02e-6;
t1715 = t1604.*(t1265-t1373).*(-9.0e-8);
t1717 = t1604.*(t1265-t1373).*9.0e-8;
t1729 = -t1612.*(t1137-t1146+t12.*(t635-t996).*1.02e-6+t17.*(t635-t996).*9.0e-8);
t1730 = -t1613.*(-t1136+t1148+t12.*(t635-t996).*9.0e-8+t17.*(t635-t996).*9.3e-7);
t1738 = t1244.*t1712;
t1748 = t1274+t1580+t1583;
t1750 = t1472.*t1712;
t1755 = t48+t61+t313+t340+t350+t351+t688+t689+t691+t704+t986+t1283+t1289+t1291+t1400+t1402;
t1756 = t59+t75+t313+t340+t350+t351+t688+t689+t691+t704+t986+t1283+t1289+t1291+t1400+t1402;
t1763 = t1646+t1649;
t1764 = -t1210.*(-t1336+t1620+t1480.*(t799-t1262).*1.02e-6);
t1768 = t170+t181+t538+t548+t549+t556+t915+t927+t929+t930+t1131+t1323+t1326+t1331+t1438+t1441;
t1769 = t199+t214+t538+t548+t549+t556+t915+t927+t929+t930+t1131+t1323+t1326+t1331+t1438+t1441;
t1778 = -t1777;
t1779 = t1429+t1673+t1674;
t1780 = (t1265-t1373).*(-t1336+t1620+t1480.*(t799-t1262).*1.02e-6);
t1781 = -t1497.*(-t1336+t1620+t1480.*(t799-t1262).*1.02e-6);
t1782 = t1497.*(-t1336+t1620+t1480.*(t799-t1262).*1.02e-6);
t1785 = -t1783;
t1794 = t50+t51+t58+t64+t71+t72+t1078+t1081+t1093+t1098+t1255+t1360+t1391+t1393+t1500+t1501;
t1795 = t58+t60+t64+t68+t71+t72+t1078+t1081+t1093+t1098+t1255+t1360+t1391+t1393+t1500+t1501;
t1796 = t1243.*t1786;
t1800 = -t1786.*(t778-t1247);
t1805 = t1216+t1246+t1509+t1521+t1576+t1577;
t1806 = -t1786.*(t1077-t1079+t1186-t1191);
t1807 = t1786.*(t1077-t1079+t1186-t1191);
t1812 = t175+t177+t198+t201+t202+t207+t1162+t1167+t1170+t1172+t1310+t1417+t1433+t1436+t1532+t1533;
t1813 = t194+t198+t201+t202+t207+t208+t1162+t1167+t1170+t1172+t1310+t1417+t1433+t1436+t1532+t1533;
t1826 = -t1825;
t1832 = -t1830;
et1 = t1613.*(-t1136+t1148+t12.*(t635-t996).*9.0e-8+t17.*(t635-t996).*9.3e-7);
et2 = t1612.*(t1137-t1146+t12.*(t635-t996).*1.02e-6+t17.*(t635-t996).*9.0e-8)+t1237.*(t1265-t1373);
t1846 = -t1243.*(et1+et2);
et3 = t1613.*(-t1136+t1148+t12.*(t635-t996).*9.0e-8+t17.*(t635-t996).*9.3e-7);
et4 = t1612.*(t1137-t1146+t12.*(t635-t996).*1.02e-6+t17.*(t635-t996).*9.0e-8)+t1237.*(t1265-t1373);
t1847 = t1243.*(et3+et4);
et5 = t1613.*(-t1136+t1148+t12.*(t635-t996).*9.0e-8+t17.*(t635-t996).*9.3e-7);
et6 = t1612.*(t1137-t1146+t12.*(t635-t996).*1.02e-6+t17.*(t635-t996).*9.0e-8)+t1237.*(t1265-t1373);
t1852 = (et5+et6).*(t778-t1247);
t1865 = t342+t347+t348+t365+t681+t687+t702+t703+t985+t1078+t1081+t1093+t1098+t1284+t1286+t1293+t1388+t1391+t1393+t1397+t1500+t1501;
et7 = t1613.*(-t1136+t1148+t12.*(t635-t996).*9.0e-8+t17.*(t635-t996).*9.3e-7);
et8 = t1612.*(t1137-t1146+t12.*(t635-t996).*1.02e-6+t17.*(t635-t996).*9.0e-8)+t1237.*(t1265-t1373);
t1870 = (et7+et8).*(t1077-t1079+t1186-t1191);
et9 = t1613.*(-t1136+t1148+t12.*(t635-t996).*9.0e-8+t17.*(t635-t996).*9.3e-7);
et10 = t1612.*(t1137-t1146+t12.*(t635-t996).*1.02e-6+t17.*(t635-t996).*9.0e-8)+t1237.*(t1265-t1373);
t1876 = -t1480.*(et9+et10);
et11 = t1613.*(-t1136+t1148+t12.*(t635-t996).*9.0e-8+t17.*(t635-t996).*9.3e-7);
et12 = t1612.*(t1137-t1146+t12.*(t635-t996).*1.02e-6+t17.*(t635-t996).*9.0e-8)+t1237.*(t1265-t1373);
t1877 = t1480.*(et11+et12);
t1884 = t377+t382+t383+t400+t731+t751+t758+t759+t1002+t1107+t1112+t1114+t1117+t1302+t1303+t1308+t1405+t1407+t1409+t1413+t1522+t1523;
t1954 = t1735+t1784+t1789;
t1960 = t1758+t1831+t1835;
t1510 = t1487.*9.99471e-3;
t1511 = t1486.*1.838876e-2;
t1526 = t1503.*9.99471e-3;
t1527 = t1502.*1.838876e-2;
t1537 = t1502.*1.33637554986e-4;
t1538 = t1503.*7.26350557185e-5;
t1606 = t1353+t1487;
t1607 = t1358+t1486;
t1619 = t1377+t1503;
t1624 = t1382+t1502;
t1628 = -t1625;
t1630 = -t1629;
t1656 = -t1652;
t1658 = -t1657;
t1670 = t1260.*(t1355-t1486).*(-1.02e-6);
t1671 = t1260.*(t1355-t1486).*(-9.0e-8);
t1683 = t1371.*(t1355-t1486).*(-1.02e-6);
t1684 = t1371.*(t1355-t1486).*(-9.0e-8);
t1709 = t1477.*(t1355-t1486).*(-1.02e-6);
t1710 = t1477.*(t1355-t1486).*(-9.0e-8);
t1721 = t1497.*(t1355-t1486).*(-1.02e-6);
t1722 = t1497.*(t1355-t1486).*(-9.0e-8);
t1732 = (t1378-t1502).*(t1137-t1146+t12.*(t635-t996).*1.02e-6+t17.*(t635-t996).*9.0e-8);
t1739 = -t1738;
t1751 = -t1750;
t1754 = t1210.*t1748;
t1759 = t1336+t1616+t1621;
t1770 = t1210.*t1763;
t1773 = -t1748.*(t1265-t1373);
t1774 = t1497.*t1748;
t1775 = t1748.*(t1265-t1373);
t1787 = t1542+t1632+t1636;
t1790 = -t1763.*(t1265-t1373);
t1791 = t1497.*t1763;
t1792 = t1763.*(t1265-t1373);
t1793 = t1210.*t1779;
t1809 = -t1779.*(t1265-t1373);
t1810 = t1497.*t1779;
t1811 = t1779.*(t1265-t1373);
t1819 = t997.*t1805;
t1827 = -t1805.*(t799-t1262);
t1828 = t1371.*t1805;
t1833 = t1238+t1317+t1549+t1550+t1609+t1611;
t1837 = t1277+t1278+t1578+t1582+t1586+t1587;
t1838 = t1555+t1729+t1730;
t1845 = t1597+t1600+t1640+t1642;
t1853 = -t1852;
t1855 = t319+t331+t332+t334+t669+t672+t675+t676+t981+t989+t1074+t1086+t1087+t1099+t1193+t1257+t1287+t1294+t1361+t1390+t1395+t1504+t1505;
t1863 = t366+t367+t373+t391+t695+t706+t715+t716+t994+t1005+t1101+t1108+t1118+t1119+t1202+t1273+t1304+t1309+t1385+t1406+t1411+t1524+t1525;
t1882 = (t642-t1014).*(t1337-t1340+t1623+t1625+t1479.*(t799-t1262).*5.7e-7+t1480.*(t799-t1262).*4.0e-8);
t1885 = -t984.*(t323+t324-t342+t349+t678+t690+t692+t693+t982+t1074+t1086+t1087-t1098+t1281+t1290-t1293+t1390+t1392+t1395-t1397+t1504+t1505);
t1888 = t997.*(t358+t359-t377+t386+t728-t731+t735+t736+t998+t1101+t1108-t1117+t1119+t1299-t1303-t1308-t1405+t1406+t1411-t1413+t1524+t1525).*(-7.26735e-3);
t1891 = (t642-t1014).*(t1651+t1652+t1479.*(t1097-t1103+t1196-t1201).*5.7e-7+t1480.*(t1097-t1103+t1196-t1201).*4.0e-8);
t1893 = -t1492.*(t1337-t1340+t1623+t1625+t1479.*(t799-t1262).*5.7e-7+t1480.*(t799-t1262).*4.0e-8);
t1894 = -t1499.*(t1337-t1340+t1623+t1625+t1479.*(t799-t1262).*5.7e-7+t1480.*(t799-t1262).*4.0e-8);
t1895 = -t1492.*(t1651+t1652+t1479.*(t1097-t1103+t1196-t1201).*5.7e-7+t1480.*(t1097-t1103+t1196-t1201).*4.0e-8);
t1896 = -t1499.*(t1651+t1652+t1479.*(t1097-t1103+t1196-t1201).*5.7e-7+t1480.*(t1097-t1103+t1196-t1201).*4.0e-8);
t1897 = t1207+t1275+t1280+t1489+t1491+t1579+t1581+t1585+t1588;
t1935 = -t1210.*(-t1591-t1592+t1650+t1657+t1479.*(t1097-t1103+t1196-t1201).*4.0e-8+t1480.*(t1097-t1103+t1196-t1201).*2.4e-7);
t1936 = t1210.*(-t1591-t1592+t1650+t1657+t1479.*(t1097-t1103+t1196-t1201).*4.0e-8+t1480.*(t1097-t1103+t1196-t1201).*2.4e-7);
t1945 = (t1265-t1373).*(-t1591-t1592+t1650+t1657+t1479.*(t1097-t1103+t1196-t1201).*4.0e-8+t1480.*(t1097-t1103+t1196-t1201).*2.4e-7);
t1946 = -t1497.*(-t1591-t1592+t1650+t1657+t1479.*(t1097-t1103+t1196-t1201).*4.0e-8+t1480.*(t1097-t1103+t1196-t1201).*2.4e-7);
t1953 = t1734+t1785+t1788;
t1959 = t1757+t1832+t1834;
t1514 = -t1510;
t1515 = -t1511;
t1528 = -t1526;
t1529 = -t1527;
t1668 = t1260.*t1606.*9.3e-7;
t1669 = t1260.*t1606.*9.0e-8;
t1681 = t1371.*t1606.*9.3e-7;
t1682 = t1371.*t1606.*9.0e-8;
t1707 = t1477.*t1606.*9.3e-7;
t1708 = t1477.*t1606.*9.0e-8;
t1719 = t1497.*t1606.*9.3e-7;
t1720 = t1497.*t1606.*9.0e-8;
t1731 = -t1619.*(-t1136+t1148+t12.*(t635-t996).*9.0e-8+t17.*(t635-t996).*9.3e-7);
t1797 = t48+t55+t56+t61+t70+t73+t1076+t1088+t1090+t1095+t1256+t1364+t1394+t1399+t1510+t1511;
t1798 = t55+t56+t59+t70+t73+t75+t1076+t1088+t1090+t1095+t1256+t1364+t1394+t1399+t1510+t1511;
t1799 = t1244.*t1787;
t1801 = t1347.*t1787;
t1808 = t1472.*t1787;
t1814 = t173+t188+t196+t197+t212+t216+t1161+t1166+t1171+t1173+t1313+t1420+t1437+t1439+t1537+t1538;
t1815 = t192+t196+t197+t212+t216+t218+t1161+t1166+t1171+t1173+t1313+t1420+t1437+t1439+t1537+t1538;
t1829 = -t1828;
t1836 = t997.*t1833;
t1840 = -t1833.*(t799-t1262);
t1841 = t1371.*t1833;
t1843 = -t1837.*(t642-t1014);
t1844 = t1837.*(t642-t1014);
t1848 = -t1244.*(t1556-t1732+t1619.*(-t1136+t1148+t12.*(t635-t996).*9.0e-8+t17.*(t635-t996).*9.3e-7));
t1849 = t1244.*(t1556-t1732+t1619.*(-t1136+t1148+t12.*(t635-t996).*9.0e-8+t17.*(t635-t996).*9.3e-7));
t1850 = t997.*t1845;
t1854 = -t1347.*(t1556-t1732+t1619.*(-t1136+t1148+t12.*(t635-t996).*9.0e-8+t17.*(t635-t996).*9.3e-7));
t1856 = t333+t335+t336+t355+t670+t671+t677+t685+t987+t993+t1076+t1088+t1089+t1090+t1194+t1256+t1292+t1296+t1364+t1394+t1399+t1510+t1511;
t1857 = t1339+t1340+t1614+t1618+t1627+t1628;
t1860 = t44.*t108.*t1855.*9.543032792050485e-17;
t1864 = t368+t390+t392+t393+t696+t697+t720+t743+t1004+t1012+t1106+t1109+t1110+t1120+t1203+t1272+t1307+t1312+t1387+t1410+t1415+t1526+t1527;
t1867 = -t1845.*(t799-t1262);
t1868 = t1371.*t1845;
t1871 = -t1472.*(t1556-t1732+t1619.*(-t1136+t1148+t12.*(t635-t996).*9.0e-8+t17.*(t635-t996).*9.3e-7));
t1872 = t1472.*(t1556-t1732+t1619.*(-t1136+t1148+t12.*(t635-t996).*9.0e-8+t17.*(t635-t996).*9.3e-7));
t1873 = t44.*t116.*t1863.*6.935255936130809e-19;
t1878 = t1492.*t1837;
t1879 = t1499.*t1837;
t1880 = -t1483.*(t1556-t1732+t1619.*(-t1136+t1148+t12.*(t635-t996).*9.0e-8+t17.*(t635-t996).*9.3e-7));
t1881 = t1483.*(t1556-t1732+t1619.*(-t1136+t1148+t12.*(t635-t996).*9.0e-8+t17.*(t635-t996).*9.3e-7));
t1883 = -t1882;
t1889 = t1643+t1648+t1654+t1656;
t1892 = -t1891;
t1898 = t1210.*t1897;
t1906 = -t1897.*(t1265-t1373);
t1907 = t1497.*t1897;
t1908 = t1897.*(t1265-t1373);
t1911 = t1236+t1338+t1342+t1547+t1548+t1615+t1617+t1626+t1630;
t1916 = t1700+t1885;
t1922 = t1723+t1888;
t1931 = t1591+t1592+t1644+t1647+t1653+t1658;
t1947 = -t1945;
t1802 = -t1801;
t1839 = t1558+t1731+t1732;
t1842 = -t1841;
t1851 = -t1850;
t1861 = t44.*t108.*t1856.*9.543032792050485e-17;
t1866 = t321+t343+t344+t352+t688+t689+t691+t704+t986+t1073+t1083+t1096+t1102+t1283+t1291+t1297+t1396+t1398+t1400+t1403+t1514+t1515;
t1869 = -t1868;
t1874 = t44.*t116.*t1864.*6.935255936130809e-19;
t1886 = t356+t380+t381+t387+t752+t753+t757+t760+t1003+t1100+t1113+t1116+t1121+t1301+t1306+t1314+t1412+t1414+t1416+t1418+t1528+t1529;
t1899 = t1422+t1428+t1663+t1665+t1668+t1671;
t1900 = t1425+t1426+t1661+t1667+t1669+t1670;
t1904 = t1694+t1860;
t1909 = t1443+t1446+t1678+t1679+t1681+t1684;
t1910 = t1444+t1445+t1676+t1680+t1682+t1683;
t1912 = t1696+t1873;
t1914 = t1704+t1705+t1707+t1710;
t1915 = t1701+t1706+t1708+t1709;
t1918 = t1210.*t1911;
t1932 = -t1911.*(t1265-t1373);
t1933 = t1497.*t1911;
t1934 = t1911.*(t1265-t1373);
t1948 = t1450+t1458+t1716+t1717+t1719+t1722;
t1949 = t1454+t1455+t1714+t1718+t1720+t1721;
t1961 = t1765+t1877+t1881;
t1962 = t1819+t1844+t1898;
t1964 = t1827+t1878+t1908;
t1965 = t1829+t1879+t1907;
t1973 = t1850+t1892+t1935;
t1976 = t1867+t1895+t1947;
t1862 = -t1861;
t1875 = -t1874;
t1887 = t984.*t1866;
t1890 = t997.*t1886.*7.26735e-3;
t1901 = t1318.*t1899;
t1903 = t1319.*t1900;
t1919 = t1318.*t1909;
t1920 = t1319.*t1910;
t1924 = t1318.*t1914;
t1926 = t1319.*t1915;
t1927 = t1613.*t1899;
t1928 = t1612.*t1900;
t1929 = t1619.*t1899;
t1930 = -t1900.*(t1378-t1502);
t1937 = t1612.*t1910;
t1938 = t1613.*t1909;
t1939 = t1619.*t1909;
t1940 = -t1910.*(t1378-t1502);
t1941 = t1612.*t1915;
t1942 = t1613.*t1914;
t1943 = t1619.*t1914;
t1944 = -t1915.*(t1378-t1502);
t1950 = t1318.*t1948;
t1952 = t1319.*t1949;
t1955 = t1612.*t1949;
t1956 = t1613.*t1948;
t1957 = t1619.*t1948;
t1958 = -t1949.*(t1378-t1502);
t1966 = t1836+t1883+t1918;
t1971 = t1840+t1893+t1934;
t1972 = t1842+t1894+t1933;
t1977 = t1869+t1896+t1946;
t1902 = -t1901;
t1905 = t1695+t1862;
t1913 = t1697+t1875;
t1917 = t1702+t1887;
t1921 = -t1920;
t1923 = t1724+t1890;
t1925 = -t1924;
t1951 = -t1950;
t1969 = t1775+t1927+t1928;
t1970 = t1774+t1929+t1930;
t1974 = t1780+t1937+t1938;
t1975 = t1782+t1939+t1940;
t1978 = t1792+t1941+t1942;
t1979 = t1791+t1943+t1944;
t1981 = t1811+t1955+t1956;
t1982 = t1810+t1957+t1958;
t1963 = t1754+t1902+t1903;
t1967 = t1764+t1919+t1921;
t1968 = t1770+t1925+t1926;
t1980 = t1793+t1951+t1952;
et13 = t18.*1.0173523574586e-3-t24.*4.418500737171001e-4;
et14 = t32.*3.222314966007e-4+t33.*4.573233567645e-4;
et15 = t18.*4.418500737171001e-4+t24.*1.0173523574586e-3;
et16 = t32.*(-4.573233567645e-4)+t33.*3.222314966007e-4;
et17 = t656+t1018+t1584+t1733+t1760-t1768.*(t47+t69-t313+t320-t350-t351+t679+t680-t691+t694-t1283-t1289-t1291-t1400+t1401+t15.*t44.*t108.*(t36-t37).*7.987216665362745e-37)+t1462.*t1551+t1726.*t1743+t1753.*t1766+t1795.*t1812+t1798.*t1814-t1463.*(t164-t165-t499+t504-t517-t518-t892+t895+t897+t898)+t1728.*(-t168+t176+t534+t543+t560+t561+t910+t911+t926+t928+t1129+t1138+t1169+t1220+t1328+t1332);
et18 = 3.61e-6;
et19 = t375+t376-t384-t385-t397+t402+t403-t406-t411-t412-t416-t417-t419+t420-t423+t425-t705+t709-t711-t712-t719-t721+t722+t723+t727+t732+t738-t741+t763+t764+t767+t768+t832-t835+t837+t838-t844-t845-t847+t850+t861+t864-t870-t875-t876+t880+t881;
H = ft_4({et13,et14,et15,et16,et17,et18,et19,t10,t1018,t1020,t1022,t1026,t1027,t1028,t1033,t1034,t1035,t1039,t1043,t1044,t1045,t1048,t1049,t1051,t1052,t1063,t1064,t107,t1074,t1077,t1079,t108,t1086,t1087,t1092,t1097,t1098,t1101,t1103,t1108,t1117,t1119,t1124,t1127,t1129,t1138,t1141,t1145,t115,t116,t1169,t1186,t1191,t1194,t1196,t1201,t1205,t1210,t1220,t1226,t1227,t1234,t1235,t1243,t1244,t1247,t1258,t1259,t1260,t1261,t1262,t1281,t1283,t1289,t1290,t1291,t1292,t1293,t1296,t1299,t130,t1303,t1308,t131,t132,t1323,t1326,t1328,t1331,t1332,t1336,t1337,t134,t1340,t1347,t1390,t1392,t1395,t1397,t1400,t1401,t1404,t1405,t1406,t1408,t1411,t1413,t143,t1438,t1440,t145,t1462,t1463,t1469,t1470,t1471,t1472,t1477,t1479,t1480,t1483,t1488,t1492,t1497,t1499,t15,t1504,t1505,t1524,t1525,t1530,t1536,t1539,t1546,t1551,t1554,t1584,t1591,t1592,t1608,t1620,t1623,t1625,t1633,t1634,t1638,t164,t165,t1650,t1651,t1652,t1655,t1657,t1660,t1662,t168,t1685,t1686,t1687,t1689,t1691,t1692,t1698,t1725,t1726,t1728,t1733,t1734,t1737,t1739,t1740,t1741,t1743,t1744,t1746,t1747,t1749,t1751,t1752,t1753,t1755,t1757,t176,t1760,t1761,t1762,t1766,t1767,t1768,t1771,t1776,t1778,t1783,t1794,t1795,t1796,t1797,t1798,t1799,t1800,t1802,t1803,t1804,t1807,t1808,t1812,t1813,t1814,t1815,t1816,t1818,t1820,t1822,t1824,t1826,t1830,t1833,t1841,t1845,t1847,t1849,t1851,t1853,t1854,t1858,t1868,t1870,t1872,t189,t1891,t1904,t1905,t1912,t1913,t1917,t1919,t1920,t1923,t1932,t1933,t1936,t1945,t1954,t1960,t1961,t1962,t1963,t1964,t1965,t1966,t1967,t1968,t1969,t1970,t1974,t1975,t1978,t1979,t1980,t1981,t1982,t20,t203,t26,t313,t320,t323,t324,t328,t342,t345,t349,t350,t351,t358,t359,t36,t360,t361,t37,t375,t376,t377,t384,t385,t386,t397,t40,t402,t403,t406,t41,t411,t412,t416,t417,t419,t420,t423,t425,t44,t47,t48,t49,t493,t497,t498,t499,t50,t504,t505,t51,t517,t518,t52,t534,t538,t542,t543,t548,t549,t560,t561,t576,t577,t582,t583,t587,t588,t591,t597,t598,t599,t603,t606,t61,t610,t616,t625,t628,t646,t652,t656,t670,t671,t677,t678,t679,t68,t680,t685,t69,t690,t691,t692,t693,t694,t705,t709,t711,t712,t719,t721,t722,t723,t727,t728,t731,t732,t735,t736,t738,t741,t763,t764,t767,t768,t778,t786,t790,t799,t8,t832,t835,t837,t838,t844,t845,t847,t850,t861,t864,t87,t870,t875,t876,t880,t881,t892,t895,t897,t898,t9,t910,t911,t915,t919,t921,t922,t926,t928,t937,t940,t941,t944,t945,t946,t948,t949,t956,t957,t958,t959,t962,t963,t968,t969,t982,t984,t987,t993,t997,t998});
end
function H = ft_4(ct)
et13 = ct{1};
et14 = ct{2};
et15 = ct{3};
et16 = ct{4};
et17 = ct{5};
et18 = ct{6};
et19 = ct{7};
t10 = ct{8};
t1018 = ct{9};
t1020 = ct{10};
t1022 = ct{11};
t1026 = ct{12};
t1027 = ct{13};
t1028 = ct{14};
t1033 = ct{15};
t1034 = ct{16};
t1035 = ct{17};
t1039 = ct{18};
t1043 = ct{19};
t1044 = ct{20};
t1045 = ct{21};
t1048 = ct{22};
t1049 = ct{23};
t1051 = ct{24};
t1052 = ct{25};
t1063 = ct{26};
t1064 = ct{27};
t107 = ct{28};
t1074 = ct{29};
t1077 = ct{30};
t1079 = ct{31};
t108 = ct{32};
t1086 = ct{33};
t1087 = ct{34};
t1092 = ct{35};
t1097 = ct{36};
t1098 = ct{37};
t1101 = ct{38};
t1103 = ct{39};
t1108 = ct{40};
t1117 = ct{41};
t1119 = ct{42};
t1124 = ct{43};
t1127 = ct{44};
t1129 = ct{45};
t1138 = ct{46};
t1141 = ct{47};
t1145 = ct{48};
t115 = ct{49};
t116 = ct{50};
t1169 = ct{51};
t1186 = ct{52};
t1191 = ct{53};
t1194 = ct{54};
t1196 = ct{55};
t1201 = ct{56};
t1205 = ct{57};
t1210 = ct{58};
t1220 = ct{59};
t1226 = ct{60};
t1227 = ct{61};
t1234 = ct{62};
t1235 = ct{63};
t1243 = ct{64};
t1244 = ct{65};
t1247 = ct{66};
t1258 = ct{67};
t1259 = ct{68};
t1260 = ct{69};
t1261 = ct{70};
t1262 = ct{71};
t1281 = ct{72};
t1283 = ct{73};
t1289 = ct{74};
t1290 = ct{75};
t1291 = ct{76};
t1292 = ct{77};
t1293 = ct{78};
t1296 = ct{79};
t1299 = ct{80};
t130 = ct{81};
t1303 = ct{82};
t1308 = ct{83};
t131 = ct{84};
t132 = ct{85};
t1323 = ct{86};
t1326 = ct{87};
t1328 = ct{88};
t1331 = ct{89};
t1332 = ct{90};
t1336 = ct{91};
t1337 = ct{92};
t134 = ct{93};
t1340 = ct{94};
t1347 = ct{95};
t1390 = ct{96};
t1392 = ct{97};
t1395 = ct{98};
t1397 = ct{99};
t1400 = ct{100};
t1401 = ct{101};
t1404 = ct{102};
t1405 = ct{103};
t1406 = ct{104};
t1408 = ct{105};
t1411 = ct{106};
t1413 = ct{107};
t143 = ct{108};
t1438 = ct{109};
t1440 = ct{110};
t145 = ct{111};
t1462 = ct{112};
t1463 = ct{113};
t1469 = ct{114};
t1470 = ct{115};
t1471 = ct{116};
t1472 = ct{117};
t1477 = ct{118};
t1479 = ct{119};
t1480 = ct{120};
t1483 = ct{121};
t1488 = ct{122};
t1492 = ct{123};
t1497 = ct{124};
t1499 = ct{125};
t15 = ct{126};
t1504 = ct{127};
t1505 = ct{128};
t1524 = ct{129};
t1525 = ct{130};
t1530 = ct{131};
t1536 = ct{132};
t1539 = ct{133};
t1546 = ct{134};
t1551 = ct{135};
t1554 = ct{136};
t1584 = ct{137};
t1591 = ct{138};
t1592 = ct{139};
t1608 = ct{140};
t1620 = ct{141};
t1623 = ct{142};
t1625 = ct{143};
t1633 = ct{144};
t1634 = ct{145};
t1638 = ct{146};
t164 = ct{147};
t165 = ct{148};
t1650 = ct{149};
t1651 = ct{150};
t1652 = ct{151};
t1655 = ct{152};
t1657 = ct{153};
t1660 = ct{154};
t1662 = ct{155};
t168 = ct{156};
t1685 = ct{157};
t1686 = ct{158};
t1687 = ct{159};
t1689 = ct{160};
t1691 = ct{161};
t1692 = ct{162};
t1698 = ct{163};
t1725 = ct{164};
t1726 = ct{165};
t1728 = ct{166};
t1733 = ct{167};
t1734 = ct{168};
t1737 = ct{169};
t1739 = ct{170};
t1740 = ct{171};
t1741 = ct{172};
t1743 = ct{173};
t1744 = ct{174};
t1746 = ct{175};
t1747 = ct{176};
t1749 = ct{177};
t1751 = ct{178};
t1752 = ct{179};
t1753 = ct{180};
t1755 = ct{181};
t1757 = ct{182};
t176 = ct{183};
t1760 = ct{184};
t1761 = ct{185};
t1762 = ct{186};
t1766 = ct{187};
t1767 = ct{188};
t1768 = ct{189};
t1771 = ct{190};
t1776 = ct{191};
t1778 = ct{192};
t1783 = ct{193};
t1794 = ct{194};
t1795 = ct{195};
t1796 = ct{196};
t1797 = ct{197};
t1798 = ct{198};
t1799 = ct{199};
t1800 = ct{200};
t1802 = ct{201};
t1803 = ct{202};
t1804 = ct{203};
t1807 = ct{204};
t1808 = ct{205};
t1812 = ct{206};
t1813 = ct{207};
t1814 = ct{208};
t1815 = ct{209};
t1816 = ct{210};
t1818 = ct{211};
t1820 = ct{212};
t1822 = ct{213};
t1824 = ct{214};
t1826 = ct{215};
t1830 = ct{216};
t1833 = ct{217};
t1841 = ct{218};
t1845 = ct{219};
t1847 = ct{220};
t1849 = ct{221};
t1851 = ct{222};
t1853 = ct{223};
t1854 = ct{224};
t1858 = ct{225};
t1868 = ct{226};
t1870 = ct{227};
t1872 = ct{228};
t189 = ct{229};
t1891 = ct{230};
t1904 = ct{231};
t1905 = ct{232};
t1912 = ct{233};
t1913 = ct{234};
t1917 = ct{235};
t1919 = ct{236};
t1920 = ct{237};
t1923 = ct{238};
t1932 = ct{239};
t1933 = ct{240};
t1936 = ct{241};
t1945 = ct{242};
t1954 = ct{243};
t1960 = ct{244};
t1961 = ct{245};
t1962 = ct{246};
t1963 = ct{247};
t1964 = ct{248};
t1965 = ct{249};
t1966 = ct{250};
t1967 = ct{251};
t1968 = ct{252};
t1969 = ct{253};
t1970 = ct{254};
t1974 = ct{255};
t1975 = ct{256};
t1978 = ct{257};
t1979 = ct{258};
t1980 = ct{259};
t1981 = ct{260};
t1982 = ct{261};
t20 = ct{262};
t203 = ct{263};
t26 = ct{264};
t313 = ct{265};
t320 = ct{266};
t323 = ct{267};
t324 = ct{268};
t328 = ct{269};
t342 = ct{270};
t345 = ct{271};
t349 = ct{272};
t350 = ct{273};
t351 = ct{274};
t358 = ct{275};
t359 = ct{276};
t36 = ct{277};
t360 = ct{278};
t361 = ct{279};
t37 = ct{280};
t375 = ct{281};
t376 = ct{282};
t377 = ct{283};
t384 = ct{284};
t385 = ct{285};
t386 = ct{286};
t397 = ct{287};
t40 = ct{288};
t402 = ct{289};
t403 = ct{290};
t406 = ct{291};
t41 = ct{292};
t411 = ct{293};
t412 = ct{294};
t416 = ct{295};
t417 = ct{296};
t419 = ct{297};
t420 = ct{298};
t423 = ct{299};
t425 = ct{300};
t44 = ct{301};
t47 = ct{302};
t48 = ct{303};
t49 = ct{304};
t493 = ct{305};
t497 = ct{306};
t498 = ct{307};
t499 = ct{308};
t50 = ct{309};
t504 = ct{310};
t505 = ct{311};
t51 = ct{312};
t517 = ct{313};
t518 = ct{314};
t52 = ct{315};
t534 = ct{316};
t538 = ct{317};
t542 = ct{318};
t543 = ct{319};
t548 = ct{320};
t549 = ct{321};
t560 = ct{322};
t561 = ct{323};
t576 = ct{324};
t577 = ct{325};
t582 = ct{326};
t583 = ct{327};
t587 = ct{328};
t588 = ct{329};
t591 = ct{330};
t597 = ct{331};
t598 = ct{332};
t599 = ct{333};
t603 = ct{334};
t606 = ct{335};
t61 = ct{336};
t610 = ct{337};
t616 = ct{338};
t625 = ct{339};
t628 = ct{340};
t646 = ct{341};
t652 = ct{342};
t656 = ct{343};
t670 = ct{344};
t671 = ct{345};
t677 = ct{346};
t678 = ct{347};
t679 = ct{348};
t68 = ct{349};
t680 = ct{350};
t685 = ct{351};
t69 = ct{352};
t690 = ct{353};
t691 = ct{354};
t692 = ct{355};
t693 = ct{356};
t694 = ct{357};
t705 = ct{358};
t709 = ct{359};
t711 = ct{360};
t712 = ct{361};
t719 = ct{362};
t721 = ct{363};
t722 = ct{364};
t723 = ct{365};
t727 = ct{366};
t728 = ct{367};
t731 = ct{368};
t732 = ct{369};
t735 = ct{370};
t736 = ct{371};
t738 = ct{372};
t741 = ct{373};
t763 = ct{374};
t764 = ct{375};
t767 = ct{376};
t768 = ct{377};
t778 = ct{378};
t786 = ct{379};
t790 = ct{380};
t799 = ct{381};
t8 = ct{382};
t832 = ct{383};
t835 = ct{384};
t837 = ct{385};
t838 = ct{386};
t844 = ct{387};
t845 = ct{388};
t847 = ct{389};
t850 = ct{390};
t861 = ct{391};
t864 = ct{392};
t87 = ct{393};
t870 = ct{394};
t875 = ct{395};
t876 = ct{396};
t880 = ct{397};
t881 = ct{398};
t892 = ct{399};
t895 = ct{400};
t897 = ct{401};
t898 = ct{402};
t9 = ct{403};
t910 = ct{404};
t911 = ct{405};
t915 = ct{406};
t919 = ct{407};
t921 = ct{408};
t922 = ct{409};
t926 = ct{410};
t928 = ct{411};
t937 = ct{412};
t940 = ct{413};
t941 = ct{414};
t944 = ct{415};
t945 = ct{416};
t946 = ct{417};
t948 = ct{418};
t949 = ct{419};
t956 = ct{420};
t957 = ct{421};
t958 = ct{422};
t959 = ct{423};
t962 = ct{424};
t963 = ct{425};
t968 = ct{426};
t969 = ct{427};
t982 = ct{428};
t984 = ct{429};
t987 = ct{430};
t993 = ct{431};
t997 = ct{432};
t998 = ct{433};
et20 = t8.*t9.*t15.*t44.*t108.*(-3.670836568391568e-22);
et21 = t656+t1018+t1584+t1733+t1760-t1755.*(t189+t203-t538+t542-t548-t549-t915+t919+t921+t922-t1323-t1326-t1331-t1438+t1440+t26.*t44.*t116.*(t40-t41).*8.687615694748404e-39)+t1469.*t1530+t1725.*t1744+t1752.*t1767+t1794.*t1813+t1797.*t1815;
et22 = -t1470.*(t493-t497-t498-t505-t892+t895+t897+t898)+t1746.*(-t48+t52+t328+t345+t360+t361+t670+t671+t677+t685+t987+t993+t1092+t1194+t1292+t1296)+3.61e-6;
et23 = t189+t203-t538+t542-t548-t549-t915+t919+t921+t922-t1323-t1326-t1331-t1438+t1440+t26.*t44.*t116.*(t40-t41).*8.687615694748404e-39;
et24 = t47+t69-t313+t320-t350-t351+t679+t680-t691+t694-t1283-t1289-t1291-t1400+t1401+t15.*t44.*t108.*(t36-t37).*7.987216665362745e-37;
et25 = t1689+t1691+t1749+t1751+t1807+t1808+t1870+t1872+t1404.*t1744.*(t1077-t1079+t1186-t1191)-t1536.*t1767.*(t1077-t1079+t1186-t1191)-t1813.*(t1077-t1079+t1186-t1191).*(t646+t786+t1020+t1124+t1127+t1226+t1227);
et26 = t1472.*t1536.*(t189+t203-t538+t542-t548-t549-t915+t919+t921+t922-t1323-t1326-t1331-t1438+t1440+t26.*t44.*t116.*(t40-t41).*8.687615694748404e-39)-t1404.*t1472.*t1746-t1472.*t1815.*(t646+t786+t1020+t1124+t1127+t1226+t1227);
et27 = t375+t376-t384-t385-t397+t402+t403-t406-t411-t412-t416-t417-t419+t420-t423+t425-t705+t709-t711-t712-t719-t721+t722+t723+t727+t732+t738-t741+t763+t764+t767+t768+t832-t835+t837+t838-t844-t845-t847+t850+t861+t864-t870-t875-t876+t880+t881;
et28 = t8.*t9.*t15.*t44.*t108.*(-3.670836568391568e-22);
et29 = t1687+t1747+t1816+t1818+t1824+t1826+t1851+t1891+t1936+t1968+t1408.*t1725.*(t1097-t1103+t1196-t1201).*2.889644e-2-t1539.*t1752.*(t1097-t1103+t1196-t1201).*1.08769e-2-t1408.*t1477.*(-t48+t52+t328+t345+t360+t361+t670+t671+t677+t685+t987+t993+t1092+t1194+t1292+t1296).*2.889644e-2;
et30 = t1794.*(t1097-t1103+t1196-t1201).*(t652+t790+t1039+t1141+t1145+t1234+t1235).*(-7.26735e-3)-t1477.*t1539.*t1755.*1.08769e-2-t1477.*t1797.*(t652+t790+t1039+t1141+t1145+t1234+t1235).*7.26735e-3;
et31 = t1687+t1747+t1816+t1818+t1824+t1826+t1851+t1891+t1936+t1968+t1408.*t1726.*(t1097-t1103+t1196-t1201).*2.889644e-2-t1539.*t1753.*(t1097-t1103+t1196-t1201).*1.08769e-2-t1795.*(t1097-t1103+t1196-t1201).*(t652+t790+t1039+t1141+t1145+t1234+t1235).*7.26735e-3;
et32 = t1477.*t1539.*(t47+t69-t313+t320-t350-t351+t679+t680-t691+t694-t1283-t1289-t1291-t1400+t1401+t15.*t44.*t108.*(t36-t37).*7.987216665362745e-37).*1.08769e-2-t1408.*t1477.*t1728.*2.889644e-2;
et33 = t1477.*t1798.*(t652+t790+t1039+t1141+t1145+t1234+t1235).*(-7.26735e-3);
et34 = t1868+t1499.*(t1651+t1652+t1479.*(t1097-t1103+t1196-t1201).*5.7e-7+t1480.*(t1097-t1103+t1196-t1201).*4.0e-8);
et35 = t1497.*(-t1591-t1592+t1650+t1657+t1479.*(t1097-t1103+t1196-t1201).*4.0e-8+t1480.*(t1097-t1103+t1196-t1201).*2.4e-7);
et36 = t115.*8.618586366948822e-4;
et37 = t143.*(-8.631097478604537e-5);
et38 = t145.*9.554306323645785e-8+t20.*t44.*t116.*2.075672598245148e-23;
et39 = t26.*t44.*t116.*1.875105520197095e-20;
et40 = t107.*2.982577219529057e-2-t131.*2.986906857247653e-3;
et41 = t132.*3.306395640309251e-6+t10.*t44.*t108.*7.183142969324763e-22+t15.*t44.*t108.*6.489053738789607e-19;
et42 = -(t1258.*t1804-t1259.*t1803+(t44.*t87.*t116.*t1686)./8.112963841460668e+31).*(t1077-t1079+t1186-t1191)+t1488.*t1554+t1472.*t1960+t1472.*t1979+t1472.*(et34+et35)+(-t1757+t1830+t1820.*(t799-t1262)).*(t1077-t1079+t1186-t1191);
et43 = (t1945+t1845.*(t799-t1262)+t1492.*(t1651+t1652+t1479.*(t1097-t1103+t1196-t1201).*5.7e-7+t1480.*(t1097-t1103+t1196-t1201).*4.0e-8)).*(t1077-t1079+t1186-t1191)+(et36+et37+et38+et39).*(et40+et41)+t1978.*(t1077-t1079+t1186-t1191);
et44 = t1472.*(t1260.*t1803+t1261.*t1804+(t44.*t116.*t1686.*(t40-t41))./8.112963841460668e+31)+t1404.*t1408.*(t1077-t1079+t1186-t1191).*(t1097-t1103+t1196-t1201).*2.889644e-2+t1536.*t1539.*(t1077-t1079+t1186-t1191).*(t1097-t1103+t1196-t1201).*1.08769e-2;
et45 = t130.*t134.*t1633.*t1634.*4.312975891071717e-75+t1404.*t1408.*t1472.*t1477.*2.889644e-2+t1472.*t1477.*t1536.*t1539.*1.08769e-2;
et46 = (t1077-t1079+t1186-t1191).*(t1097-t1103+t1196-t1201).*(t646+t786+t1020+t1124+t1127+t1226+t1227).*(t652+t790+t1039+t1141+t1145+t1234+t1235).*7.26735e-3+t1472.*t1477.*(t646+t786+t1020+t1124+t1127+t1226+t1227).*(t652+t790+t1039+t1141+t1145+t1234+t1235).*7.26735e-3;
et47 = t1868+t1499.*(t1651+t1652+t1479.*(t1097-t1103+t1196-t1201).*5.7e-7+t1480.*(t1097-t1103+t1196-t1201).*4.0e-8);
et48 = t1497.*(-t1591-t1592+t1650+t1657+t1479.*(t1097-t1103+t1196-t1201).*4.0e-8+t1480.*(t1097-t1103+t1196-t1201).*2.4e-7);
et49 = t375+t376-t384-t385-t397+t402+t403-t406-t411-t412-t416-t417-t419+t420-t423+t425-t705+t709-t711-t712-t719-t721+t722+t723+t727+t732+t738-t741+t763+t764+t767+t768+t832-t835+t837+t838-t844-t845-t847+t850+t861+t864-t870-t875-t876+t880+t881;
et50 = t8.*t9.*t15.*t44.*t108.*(-3.670836568391568e-22);
et51 = t1243.*(t1945+t1845.*(t799-t1262)+t1492.*(t1651+t1652+t1479.*(t1097-t1103+t1196-t1201).*5.7e-7+t1480.*(t1097-t1103+t1196-t1201).*4.0e-8))-t1471.*t1554+t1244.*t1960+t1243.*t1978+t1244.*t1979+t1244.*(et47+et48)+t1243.*(-t1757+t1830+t1820.*(t799-t1262));
et52 = t44.*t108.*(t1747+t1824+t1826).*9.543032792050485e-17+t44.*t108.*(t1851+t1891+t1936).*9.543032792050485e-17+t1539.*t1822.*(t1097-t1103+t1196-t1201).*1.08769e-2;
et53 = t1904.*(t1097-t1103+t1196-t1201).*(t652+t790+t1039+t1141+t1145+t1234+t1235).*7.26735e-3+t44.*t108.*t1968.*9.543032792050485e-17+t1477.*t1905.*(t652+t790+t1039+t1141+t1145+t1234+t1235).*7.26735e-3+t1477.*t1539.*(et49+et50).*1.08769e-2;
et54 = t130.*t134.*t1634.*t1685.*2.33806891548878e-94;
et55 = t1868+t1499.*(t1651+t1652+t1479.*(t1097-t1103+t1196-t1201).*5.7e-7+t1480.*(t1097-t1103+t1196-t1201).*4.0e-8);
et56 = t1497.*(-t1591-t1592+t1650+t1657+t1479.*(t1097-t1103+t1196-t1201).*4.0e-8+t1480.*(t1097-t1103+t1196-t1201).*2.4e-7);
et57 = -(t778-t1247).*(t1945+t1845.*(t799-t1262)+t1492.*(t1651+t1652+t1479.*(t1097-t1103+t1196-t1201).*5.7e-7+t1480.*(t1097-t1103+t1196-t1201).*4.0e-8))+t984.*t1968-t1347.*t1979-t1347.*(et55+et56)-t1978.*(t778-t1247)+t984.*(t1851+t1891+t1936);
et58 = (t1655.*(t778-t1247)+t984.*(t323+t324-t342+t349+t678+t690+t692+t693+t982+t1074+t1086+t1087-t1098+t1281+t1290-t1293+t1390+t1392+t1395-t1397+t1504+t1505)).*(t1097-t1103+t1196-t1201).*(t652+t790+t1039+t1141+t1145+t1234+t1235).*7.26735e-3+t1477.*t1917.*(t652+t790+t1039+t1141+t1145+t1234+t1235).*7.26735e-3;
et59 = t130.*t134.*t1634.*t1638.*(-4.788365138921021e-91);
et60 = t47+t69-t313+t320-t350-t351+t679+t680-t691+t694-t1283-t1289-t1291-t1400+t1401+t15.*t44.*t108.*(t36-t37).*7.987216665362745e-37;
et61 = -(t576+t577+t582+t583-t587-t588+t591-t597+t598+t599-t603+t606-t610+t616-t625+t628-t937+t940-t941+t944-t945-t946+t948-t949-t956+t957-t958-t959+t962+t963-t968-t969-t1022+t1026+t1027-t1028-t1033+t1034+t1035-t1043-t1044-t1045+t1048+t1049-t1051-t1052+t1063+t1064);
et62 = -t1488.*t1546+t1472.*t1954+t1472.*t1965+t1472.*t1970+(-t1734+t1783+t1771.*(t799-t1262)).*(t1077-t1079+t1186-t1191)+t1964.*(t1077-t1079+t1186-t1191)+t1969.*(t1077-t1079+t1186-t1191)+t1536.*t1858.*(t1077-t1079+t1186-t1191)+t1912.*(t1077-t1079+t1186-t1191).*(t646+t786+t1020+t1124+t1127+t1226+t1227);
et63 = -t1472.*t1536.*(t576+t577+t582+t583-t587-t588+t591-t597+t598+t599-t603+t606-t610+t616-t625+t628-t937+t940-t941+t944-t945-t946+t948-t949-t956+t957-t958-t959+t962+t963-t968-t969-t1022+t1026+t1027-t1028-t1033+t1034+t1035-t1043-t1044-t1045+t1048+t1049-t1051-t1052+t1063+t1064)+t1472.*t1913.*(t646+t786+t1020+t1124+t1127+t1226+t1227);
et64 = t130.*t134.*t1633.*t1692.*2.33806891548878e-94;
et65 = t375+t376-t384-t385-t397+t402+t403-t406-t411-t412-t416-t417-t419+t420-t423+t425-t705+t709-t711-t712-t719-t721+t722+t723+t727+t732+t738-t741+t763+t764+t767+t768+t832-t835+t837+t838-t844-t845-t847+t850+t861+t864-t870-t875-t876+t880+t881;
et66 = t8.*t9.*t15.*t44.*t108.*(-3.670836568391568e-22);
et67 = -(et65+et66).*(t576+t577+t582+t583-t587-t588+t591-t597+t598+t599-t603+t606-t610+t616-t625+t628-t937+t940-t941+t944-t945-t946+t948-t949-t956+t957-t958-t959+t962+t963-t968-t969-t1022+t1026+t1027-t1028-t1033+t1034+t1035-t1043-t1044-t1045+t1048+t1049-t1051-t1052+t1063+t1064)+t1471.*t1546+t1244.*t1954+t1243.*t1964+t1244.*t1965+t1243.*t1969+t1244.*t1970+t1822.*t1858+t1904.*t1912+t1905.*t1913+t1243.*(-t1734+t1783+t1771.*(t799-t1262));
et68 = t44.*t108.*(t1698+t1776+t1778).*9.543032792050485e-17+t44.*t108.*t1962.*9.543032792050485e-17+t44.*t108.*t1963.*9.543032792050485e-17;
et69 = t130.*t134.*t1685.*t1692.*1.267469698796881e-113;
et70 = t984.*t1962+t984.*t1963-t1347.*t1965-t1347.*t1970+t1913.*t1917+t1912.*(t1655.*(t778-t1247)+t984.*(t323+t324-t342+t349+t678+t690+t692+t693+t982+t1074+t1086+t1087-t1098+t1281+t1290-t1293+t1390+t1392+t1395-t1397+t1504+t1505))-t1964.*(t778-t1247)-t1969.*(t778-t1247);
et71 = t130.*t134.*t1638.*t1692.*(-2.595777943136013e-110);
et72 = -t1472.*(t1841-t1933+t1499.*(t1337-t1340+t1623+t1625+t1479.*(t799-t1262).*5.7e-7+t1480.*(t799-t1262).*4.0e-8));
et73 = -(t1932+t1833.*(t799-t1262)+t1492.*(t1337-t1340+t1623+t1625+t1479.*(t799-t1262).*5.7e-7+t1480.*(t799-t1262).*4.0e-8)).*(t1077-t1079+t1186-t1191)-t1472.*t1975-t1974.*(t1077-t1079+t1186-t1191);
et74 = (t1662.*(t799-t1262).*7.26735e-3+t997.*(t358+t359-t377+t386+t728-t731+t735+t736+t998+t1101+t1108-t1117+t1119+t1299-t1303-t1308-t1405+t1406+t1411-t1413+t1524+t1525).*7.26735e-3).*(t1077-t1079+t1186-t1191).*(t646+t786+t1020+t1124+t1127+t1226+t1227)+t1472.*t1923.*(t646+t786+t1020+t1124+t1127+t1226+t1227);
et75 = t130.*t134.*t1633.*t1660.*(-4.788365138921021e-91);
et76 = -t1244.*(t1841-t1933+t1499.*(t1337-t1340+t1623+t1625+t1479.*(t799-t1262).*5.7e-7+t1480.*(t799-t1262).*4.0e-8));
et77 = t1904.*(t1662.*(t799-t1262).*7.26735e-3+t997.*(t358+t359-t377+t386+t728-t731+t735+t736+t998+t1101+t1108-t1117+t1119+t1299-t1303-t1308-t1405+t1406+t1411-t1413+t1524+t1525).*7.26735e-3)-t1243.*t1974-t1244.*t1975+t1905.*t1923;
et78 = -t1243.*(t1932+t1833.*(t799-t1262)+t1492.*(t1337-t1340+t1623+t1625+t1479.*(t799-t1262).*5.7e-7+t1480.*(t799-t1262).*4.0e-8))+t44.*t108.*t1966.*9.543032792050485e-17;
et79 = t44.*t108.*(-t1919+t1920+t1210.*(-t1336+t1620+t1480.*(t799-t1262).*1.02e-6)).*(-9.543032792050485e-17);
et80 = t130.*t134.*t1660.*t1685.*(-2.595777943136013e-110);
et81 = t1347.*(t1841-t1933+t1499.*(t1337-t1340+t1623+t1625+t1479.*(t799-t1262).*5.7e-7+t1480.*(t799-t1262).*4.0e-8))+t984.*t1966+t1347.*t1975+t1917.*t1923;
et82 = (t1662.*(t799-t1262).*7.26735e-3+t997.*(t358+t359-t377+t386+t728-t731+t735+t736+t998+t1101+t1108-t1117+t1119+t1299-t1303-t1308-t1405+t1406+t1411-t1413+t1524+t1525).*7.26735e-3).*(t1655.*(t778-t1247)+t984.*(t323+t324-t342+t349+t678+t690+t692+t693+t982+t1074+t1086+t1087-t1098+t1281+t1290-t1293+t1390+t1392+t1395-t1397+t1504+t1505));
et83 = -t984.*(-t1919+t1920+t1210.*(-t1336+t1620+t1480.*(t799-t1262).*1.02e-6))+t1974.*(t778-t1247)+(t778-t1247).*(t1932+t1833.*(t799-t1262)+t1492.*(t1337-t1340+t1623+t1625+t1479.*(t799-t1262).*5.7e-7+t1480.*(t799-t1262).*4.0e-8));
et84 = t130.*t134.*t1638.*t1660.*5.316153227542554e-107;
mt1 = [t656+t1018+t1584+t1733+t1760+(t47+t48+t61+t69).*(et13+et14)+t1469.*t1551+t1725.*t1743+t1752.*t1766+t1755.*t1768+t1794.*t1812+t1797.*t1814+(-t48+t52+t328+t345+t360+t361+t670+t671+t677+t685+t987+t993+t1092+t1194+t1292+t1296).*(-t168+t176+t534+t543+t560+t561+t910+t911+t926+t928+t1129+t1138+t1169+t1220+t1328+t1332)-t1470.*(t164-t165-t499+t504-t517-t518-t892+t895+t897+t898)+(t49+t50+t51-t68).*(et15+et16)+9.551e-5,et21+et22,et29+et30];
mt2 = [t1698+t1776+t1778+t1962+t1963-t1752.*t1858-t1794.*t1912-t1797.*t1913+t1755.*(t576+t577+t582+t583-t587-t588+t591-t597+t598+t599-t603+t606-t610+t616-t625+t628-t937+t940-t941+t944-t945-t946+t948-t949-t956+t957-t958-t959+t962+t963-t968-t969-t1022+t1026+t1027-t1028-t1033+t1034+t1035-t1043-t1044-t1045+t1048+t1049-t1051-t1052+t1063+t1064)];
mt3 = [t1966+t1967-t1794.*(t1662.*(t799-t1262).*7.26735e-3+t997.*(t358+t359-t377+t386+t728-t731+t735+t736+t998+t1101+t1108-t1117+t1119+t1299-t1303-t1308-t1405+t1406+t1411-t1413+t1524+t1525).*7.26735e-3)-t1797.*t1923,t1980,et17+et18];
mt4 = [t656+t1018+t1584+t1733+t1760+et23.*et24+t1462.*t1530+t1726.*t1744+t1728.*t1746+t1753.*t1767+t1795.*t1813+t1798.*t1815-t1463.*(t493-t497-t498-t505-t892+t895+t897+t898)+3.61e-6,et31+et32+et33,t1698+t1776+t1778+t1962+t1963-t1753.*t1858-t1795.*t1912-t1798.*t1913+et60.*et61];
mt5 = [t1966+t1967-t1795.*(t1662.*(t799-t1262).*7.26735e-3+t997.*(t358+t359-t377+t386+t728-t731+t735+t736+t998+t1101+t1108-t1117+t1119+t1299-t1303-t1308-t1405+t1406+t1411-t1413+t1524+t1525).*7.26735e-3)-t1798.*t1923,t1980];
mt6 = [t1689+t1691+t1749+t1751+t1807+t1808+t1870+t1872+t1404.*t1743.*(t1077-t1079+t1186-t1191)-t1536.*t1766.*(t1077-t1079+t1186-t1191)-t1404.*t1472.*(-t168+t176+t534+t543+t560+t561+t910+t911+t926+t928+t1129+t1138+t1169+t1220+t1328+t1332)-t1812.*(t1077-t1079+t1186-t1191).*(t646+t786+t1020+t1124+t1127+t1226+t1227)-t1472.*t1536.*t1768-t1472.*t1814.*(t646+t786+t1020+t1124+t1127+t1226+t1227),et25+et26,et42+et43+et44+et45+et46,et62+et63+et64,et72+et73+et74+et75,t1472.*t1982+t1981.*(t1077-t1079+t1186-t1191),t1608+t1737+t1739+t1740+t1761+t1796+t1799+t1847+t1849-t1766.*t1822-t1812.*t1904-t1814.*t1905-t1768.*(et19+et20)];
mt7 = [t1608+t1737+t1739+t1740+t1761+t1796+t1799+t1847+t1849+(t189+t203-t538+t542-t548-t549-t915+t919+t921+t922-t1323-t1326-t1331-t1438+t1440+t26.*t44.*t116.*(t40-t41).*8.687615694748404e-39).*(et27+et28)-t1767.*t1822-t1813.*t1904-t1815.*t1905,et51+et52+et53+et54,et67+et68+et69,et76+et77+et78+et79+et80];
mt8 = [t1243.*t1981+t1244.*t1982+t44.*t108.*t1980.*9.543032792050485e-17,t1741+t1762+t1800+t1802+t1853+t1854-t1814.*t1917-t1812.*(t1655.*(t778-t1247)+t984.*(t323+t324-t342+t349+t678+t690+t692+t693+t982+t1074+t1086+t1087-t1098+t1281+t1290-t1293+t1390+t1392+t1395-t1397+t1504+t1505)),t1741+t1762+t1800+t1802+t1853+t1854-t1815.*t1917-t1813.*(t1655.*(t778-t1247)+t984.*(t323+t324-t342+t349+t678+t690+t692+t693+t982+t1074+t1086+t1087-t1098+t1281+t1290-t1293+t1390+t1392+t1395-t1397+t1504+t1505)),et57+et58+et59,et70+et71,et81+et82+et83+et84];
mt9 = [t984.*t1980-t1347.*t1982-t1981.*(t778-t1247),t1961,t1961,t1205.*t1968+t1480.*t1978+t1483.*t1979,t1205.*t1963+t1480.*t1969+t1483.*t1970,-t1480.*t1974-t1483.*t1975-t1205.*(-t1919+t1920+t1210.*(-t1336+t1620+t1480.*(t799-t1262).*1.02e-6)),t1205.*t1980+t1480.*t1981+t1483.*t1982];
H = real(reshape([mt1,mt2,mt3,mt4,mt5,mt6,mt7,mt8,mt9],6,6));
end
